simulink model "DynamicsAaa"  (R2017a)
(part 6 of 8)

% tau4 = -0.00358942*c4*(c3*(qdd(1) + qdd(2)) - qd(3)*s3*(qd(1) + qd(2))) - c5*(-3.01352e-6*c6*(-c5*(-qdd(3) + qdd(4)) - qd(5)*(c5*(-c3*s4*(qd(1) + qd(2)) + c4*s3*(qd(1) + qd(2))) - s5*(-qd(3) + qd(4))) - s5*(c4*(c3*qd(3)*(qd(1) + qd(2)) + s3*(qdd(1) + qdd(2))) + qd(4)*(-c3*c4*(qd(1) + qd(2)) - s3*s4*(qd(1) + qd(2))) - s4*(c3*(qdd(1) + qdd(2)) - qd(3)*s3*(qd(1) + qd(2))))) - 3.01352e-6*qd(6)*(c6*(c5*(-c3*s4*(qd(1) + qd(2)) + c4*s3*(qd(1) + qd(2))) - s5*(-qd(3) + qd(4))) - s6*(-c5*(-qd(3) + qd(4)) - s5*(-c3*s4*(qd(1) + qd(2)) + c4*s3*(qd(1) + qd(2))))) - 3.01352e-6*s6*(c5*(c4*(c3*qd(3)*(qd(1) + qd(2)) + s3*(qdd(1) + qdd(2))) + qd(4)*(-c3*c4*(qd(1) + qd(2)) - s3*s4*(qd(1) + qd(2))) - s4*(c3*(qdd(1) + qdd(2)) - qd(3)*s3*(qd(1) + qd(2)))) + qd(5)*(-c5*(-qd(3) + qd(4)) - s5*(-c3*s4*(qd(1) + qd(2)) + c4*s3*(qd(1) + qd(2)))) - s5*(-qdd(3) + qdd(4))) + (6.20477e-6*c6*(c5*(-c3*s4*(qd(1) + qd(2)) + c4*s3*(qd(1) + qd(2))) - s5*(-qd(3) + qd(4))) - 6.20477e-6*s6*(-c5*(-qd(3) + qd(4)) - s5*(-c3*s4*(qd(1) + qd(2)) + c4*s3*(qd(1) + qd(2)))))*(c3*c4*(qd(1) + qd(2)) - qd(5) + qd(6) + s3*s4*(qd(1) + qd(2))) - (c6*(c5*(-c3*s4*(qd(1) + qd(2)) + c4*s3*(qd(1) + qd(2))) - s5*(-qd(3) + qd(4))) - s6*(-c5*(-qd(3) + qd(4)) - s5*(-c3*s4*(qd(1) + qd(2)) + c4*s3*(qd(1) + qd(2)))))*(3.29301e-6*c3*c4*(qd(1) + qd(2)) - 3.29301e-6*qd(5) + 3.29301e-6*qd(6) + 3.29301e-6*s3*s4*(qd(1) + qd(2)))) - 0.00358942*qd(4)*(-c3*s4*(qd(1) + qd(2)) + c4*s3*(qd(1) + qd(2))) + 0.00358942*qdd(5) - 0.00358942*s4*(c3*qd(3)*(qd(1) + qd(2)) + s3*(qdd(1) + qdd(2))) - s5*(6.20477e-6*c6*(c5*(c4*(c3*qd(3)*(qd(1) + qd(2)) + s3*(qdd(1) + qdd(2))) + qd(4)*(-c3*c4*(qd(1) + qd(2)) - s3*s4*(qd(1) + qd(2))) - s4*(c3*(qdd(1) + qdd(2)) - qd(3)*s3*(qd(1) + qd(2)))) + qd(5)*(-c5*(-qd(3) + qd(4)) - s5*(-c3*s4*(qd(1) + qd(2)) + c4*s3*(qd(1) + qd(2)))) - s5*(-qdd(3) + qdd(4))) + 6.20477e-6*qd(6)*(-c6*(-c5*(-qd(3) + qd(4)) - s5*(-c3*s4*(qd(1) + qd(2)) + c4*s3*(qd(1) + qd(2)))) - s6*(c5*(-c3*s4*(qd(1) + qd(2)) + c4*s3*(qd(1) + qd(2))) - s5*(-qd(3) + qd(4)))) - 6.20477e-6*s6*(-c5*(-qdd(3) + qdd(4)) - qd(5)*(c5*(-c3*s4*(qd(1) + qd(2)) + c4*s3*(qd(1) + qd(2))) - s5*(-qd(3) + qd(4))) - s5*(c4*(c3*qd(3)*(qd(1) + qd(2)) + s3*(qdd(1) + qdd(2))) + qd(4)*(-c3*c4*(qd(1) + qd(2)) - s3*s4*(qd(1) + qd(2))) - s4*(c3*(qdd(1) + qdd(2)) - qd(3)*s3*(qd(1) + qd(2))))) + (-c6*(-c5*(-qd(3) + qd(4)) - s5*(-c3*s4*(qd(1) + qd(2)) + c4*s3*(qd(1) + qd(2)))) - s6*(c5*(-c3*s4*(qd(1) + qd(2)) + c4*s3*(qd(1) + qd(2))) - s5*(-qd(3) + qd(4))))*(3.29301e-6*c3*c4*(qd(1) + qd(2)) - 3.29301e-6*qd(5) + 3.29301e-6*qd(6) + 3.29301e-6*s3*s4*(qd(1) + qd(2))) - (-3.01352e-6*c6*(-c5*(-qd(3) + qd(4)) - s5*(-c3*s4*(qd(1) + qd(2)) + c4*s3*(qd(1) + qd(2)))) - 3.01352e-6*s6*(c5*(-c3*s4*(qd(1) + qd(2)) + c4*s3*(qd(1) + qd(2))) - s5*(-qd(3) + qd(4))))*(c3*c4*(qd(1) + qd(2)) - qd(5) + qd(6) + s3*s4*(qd(1) + qd(2)))) - (-c5*(-qd(3) + qd(4)) - s5*(-c3*s4*(qd(1) + qd(2)) + c4*s3*(qd(1) + qd(2))))*(0.000409305*c5*(-qd(3) + qd(4)) + 0.00151607*c5*(-c3*s4*(qd(1) + qd(2)) + c4*s3*(qd(1) + qd(2))) - 0.00151607*s5*(-qd(3) + qd(4)) + 0.000409305*s5*(-c3*s4*(qd(1) + qd(2)) + c4*s3*(qd(1) + qd(2)))) + (c5*(-c3*s4*(qd(1) + qd(2)) + c4*s3*(qd(1) + qd(2))) - s5*(-qd(3) + qd(4)))*(-0.00355535*c5*(-qd(3) + qd(4)) - 0.000409305*c5*(-c3*s4*(qd(1) + qd(2)) + c4*s3*(qd(1) + qd(2))) + 0.000409305*s5*(-qd(3) + qd(4)) - 0.00355535*s5*(-c3*s4*(qd(1) + qd(2)) + c4*s3*(qd(1) + qd(2))));
%  
% tau5 = 3.29301e-6*c4*(c3*(qdd(1) + qdd(2)) - qd(3)*s3*(qd(1) + qd(2))) + 3.29301e-6*qd(4)*(-c3*s4*(qd(1) + qd(2)) + c4*s3*(qd(1) + qd(2))) - 3.29301e-6*qdd(5) + 3.29301e-6*qdd(6) + 3.29301e-6*s4*(c3*qd(3)*(qd(1) + qd(2)) + s3*(qdd(1) + qdd(2))) - (-c6*(-c5*(-qd(3) + qd(4)) - s5*(-c3*s4*(qd(1) + qd(2)) + c4*s3*(qd(1) + qd(2)))) - s6*(c5*(-c3*s4*(qd(1) + qd(2)) + c4*s3*(qd(1) + qd(2))) - s5*(-qd(3) + qd(4))))*(6.20477e-6*c6*(c5*(-c3*s4*(qd(1) + qd(2)) + c4*s3*(qd(1) + qd(2))) - s5*(-qd(3) + qd(4))) - 6.20477e-6*s6*(-c5*(-qd(3) + qd(4)) - s5*(-c3*s4*(qd(1) + qd(2)) + c4*s3*(qd(1) + qd(2))))) + (-3.01352e-6*c6*(-c5*(-qd(3) + qd(4)) - s5*(-c3*s4*(qd(1) + qd(2)) + c4*s3*(qd(1) + qd(2)))) - 3.01352e-6*s6*(c5*(-c3*s4*(qd(1) + qd(2)) + c4*s3*(qd(1) + qd(2))) - s5*(-qd(3) + qd(4))))*(c6*(c5*(-c3*s4*(qd(1) + qd(2)) + c4*s3*(qd(1) + qd(2))) - s5*(-qd(3) + qd(4))) - s6*(-c5*(-qd(3) + qd(4)) - s5*(-c3*s4*(qd(1) + qd(2)) + c4*s3*(qd(1) + qd(2)))));
%  
% tau6 = 0;


%% matrix M
% m11 = diff(tau1,qdd(1))*qdd(1) ;
% m12 = diff(tau1,qdd(2))*qdd(2) ;
% m13 = diff(tau1,qdd(3))*qdd(3) ;
% m14 = diff(tau1,qdd(4))*qdd(4) ;
% m15 = diff(tau1,qdd(5))*qdd(5) ;
% m16 = diff(tau1,qdd(6))*qdd(6) ;
% 
% m21 = diff(tau2,qdd(1))*qdd(1) ;
% m22 = diff(tau2,qdd(2))*qdd(2) ;
% m23 = diff(tau2,qdd(3))*qdd(3) ;
% m24 = diff(tau2,qdd(4))*qdd(4) ;
% m25 = diff(tau2,qdd(5))*qdd(5) ;
% m26 = diff(tau2,qdd(6))*qdd(6) ;
% 
% m31 = diff(tau3,qdd(1))*qdd(1) ;
% m32 = diff(tau3,qdd(2))*qdd(2) ;
% m33 = diff(tau3,qdd(3))*qdd(3) ;
% m34 = diff(tau3,qdd(4))*qdd(4) ;
% m35 = diff(tau3,qdd(5))*qdd(5) ;
% m36 = diff(tau3,qdd(6))*qdd(6) ;
% 
% 
% m41 = diff(tau4,qdd(1))*qdd(1) ;
% m42 = diff(tau4,qdd(2))*qdd(2) ;
% m43 = diff(tau4,qdd(3))*qdd(3) ;
% m44 = diff(tau4,qdd(4))*qdd(4) ;
% m45 = diff(tau4,qdd(5))*qdd(5) ;
% m46 = diff(tau4,qdd(6))*qdd(6) ;
% 
% 
% m51 = diff(tau5,qdd(1))*qdd(1) ;
% m52 = diff(tau5,qdd(2))*qdd(2) ;
% m53 = diff(tau5,qdd(3))*qdd(3) ;
% m54 = diff(tau5,qdd(4))*qdd(4) ;
% m55 = diff(tau5,qdd(5))*qdd(5) ;
% m56 = diff(tau5,qdd(6))*qdd(6) ;
% 
% 
% m61 = diff(tau6,qdd(1))*qdd(1) ;
% m62 = diff(tau6,qdd(2))*qdd(2) ;
% m63 = diff(tau6,qdd(3))*qdd(3) ;
% m64 = diff(tau6,qdd(4))*qdd(4) ;
% m65 = diff(tau6,qdd(5))*qdd(5) ;
% m66 = diff(tau6,qdd(6))*qdd(6) ;

% m11 =  -qdd(1)*((8581632868960513*c3)/1152921504606846976 + 75*c2*(m6*(s4*(295*c3 - 270*c3*s2) - c4*(295*s3 - 270*s2*s3)) + m5*(270*c2 + 90) + m7*s5*(s6*(s5*(c4*(295*c3 - 270*c3*s2) + s4*(295*s3 - 270*s2*s3)) - 80*c5*(c3*s4 - c4*s3) + c5*(270*c2 + 90)) + c6*(c5*(c4*(295*c3 - 270*c3*s2) + s4*(295*s3 - 270*s2*s3)) + 80*s5*(c3*s4 - c4*s3) - s5*(270*c2 + 90)) + 80*c5*s6*(c3*s4 - c4*s3) - 80*c6*s5*(c3*s4 - c4*s3)) + 270*m4*s2*s3 + c5*m7*(c6*(s5*(c4*(295*c3 - 270*c3*s2) + s4*(295*s3 - 270*s2*s3)) - 80*c5*(c3*s4 - c4*s3) + c5*(270*c2 + 90)) - s6*(c5*(c4*(295*c3 - 270*c3*s2) + s4*(295*s3 - 270*s2*s3)) + 80*s5*(c3*s4 - c4*s3) - s5*(270*c2 + 90)) + 80*s5*s6*(c3*s4 - c4*s3) + 80*c5*c6*(c3*s4 - c4*s3))) - 335*c2*(c3*(c4*(m6*(c5*(c4*(295*c3 - 270*c3*s2) + s4*(295*s3 - 270*s2*s3)) - s5*(270*c2 + 90)) - m7*s5*(c6*(s5*(c4*(295*c3 - 270*c3*s2) + s4*(295*s3 - 270*s2*s3)) - 80*c5*(c3*s4 - c4*s3) + c5*(270*c2 + 90)) - s6*(c5*(c4*(295*c3 - 270*c3*s2) + s4*(295*s3 - 270*s2*s3)) + 80*s5*(c3*s4 - c4*s3) - s5*(270*c2 + 90)) + 80*s5*s6*(c3*s4 - c4*s3) + 80*c5*c6*(c3*s4 - c4*s3)) + c5*m7*(s6*(s5*(c4*(295*c3 - 270*c3*s2) + s4*(295*s3 - 270*s2*s3)) - 80*c5*(c3*s4 - c4*s3) + c5*(270*c2 + 90)) + c6*(c5*(c4*(295*c3 - 270*c3*s2) + s4*(295*s3 - 270*s2*s3)) + 80*s5*(c3*s4 - c4*s3) - s5*(270*c2 + 90)) + 80*c5*s6*(c3*s4 - c4*s3) - 80*c6*s5*(c3*s4 - c4*s3))) - s4*(m7*(s4*(295*c3 - 270*c3*s2) - c4*(295*s3 - 270*s2*s3)) - m6*(s5*(c4*(295*c3 - 270*c3*s2) + s4*(295*s3 - 270*s2*s3)) + c5*(270*c2 + 90))) + m5*(c4*(295*c3 - 270*c3*s2) - 295*c3*c4 - 295*s3*s4 + s4*(295*s3 - 270*s2*s3))) + s3*(c4*(m7*(s4*(295*c3 - 270*c3*s2) - c4*(295*s3 - 270*s2*s3)) - m6*(s5*(c4*(295*c3 - 270*c3*s2) + s4*(295*s3 - 270*s2*s3)) + c5*(270*c2 + 90))) + s4*(m6*(c5*(c4*(295*c3 - 270*c3*s2) + s4*(295*s3 - 270*s2*s3)) - s5*(270*c2 + 90)) - m7*s5*(c6*(s5*(c4*(295*c3 - 270*c3*s2) + s4*(295*s3 - 270*s2*s3)) - 80*c5*(c3*s4 - c4*s3) + c5*(270*c2 + 90)) - s6*(c5*(c4*(295*c3 - 270*c3*s2) + s4*(295*s3 - 270*s2*s3)) + 80*s5*(c3*s4 - c4*s3) - s5*(270*c2 + 90)) + 80*s5*s6*(c3*s4 - c4*s3) + 80*c5*c6*(c3*s4 - c4*s3)) + c5*m7*(s6*(s5*(c4*(295*c3 - 270*c3*s2) + s4*(295*s3 - 270*s2*s3)) - 80*c5*(c3*s4 - c4*s3) + c5*(270*c2 + 90)) + c6*(c5*(c4*(295*c3 - 270*c3*s2) + s4*(295*s3 - 270*s2*s3)) + 80*s5*(c3*s4 - c4*s3) - s5*(270*c2 + 90)) + 80*c5*s6*(c3*s4 - c4*s3) - 80*c6*s5*(c3*s4 - c4*s3))) + m5*(s4*(295*c3 - 270*c3*s2) - 295*c3*s4 + 295*c4*s3 - c4*(295*s3 - 270*s2*s3))) - 270*c3*m4*s2) - c3*(s4*(c5*((1831324867619693*s5*s6*(c3*s4 - c4*s3))/295147905179352825856 + (1831324867619693*c5*c6*(c3*s4 - c4*s3))/295147905179352825856) + s5*((7115472921728667*c5*s6*(c3*s4 - c4*s3))/2361183241434822606848 - (7115472921728667*c6*s5*(c3*s4 - c4*s3))/2361183241434822606848) + (3495819410978605*c5*(c3*s4 - c4*s3))/2305843009213693952 + 295*m7*(s4*(295*c3 - 270*c3*s2) - c4*(295*s3 - 270*s2*s3)) + (943793072886211*s5*(c3*s4 - c4*s3))/2305843009213693952 - 295*m6*(s5*(c4*(295*c3 - 270*c3*s2) + s4*(295*s3 - 270*s2*s3)) + c5*(270*c2 + 90))) - c4*((7775400025877285*c3*c4)/2361183241434822606848 + (7775400025877285*s3*s4)/2361183241434822606848 + (943793072886211*c5*(c3*s4 - c4*s3))/2305843009213693952 + (8198078942807907*s5*(c3*s4 - c4*s3))/2305843009213693952 + 295*m6*(c5*(c4*(295*c3 - 270*c3*s2) + s4*(295*s3 - 270*s2*s3)) - s5*(270*c2 + 90)) - 295*m7*s5*(c6*(s5*(c4*(295*c3 - 270*c3*s2) + s4*(295*s3 - 270*s2*s3)) - 80*c5*(c3*s4 - c4*s3) + c5*(270*c2 + 90)) - s6*(c5*(c4*(295*c3 - 270*c3*s2) + s4*(295*s3 - 270*s2*s3)) + 80*s5*(c3*s4 - c4*s3) - s5*(270*c2 + 90)) + 80*s5*s6*(c3*s4 - c4*s3) + 80*c5*c6*(c3*s4 - c4*s3)) + 295*c5*m7*(s6*(s5*(c4*(295*c3 - 270*c3*s2) + s4*(295*s3 - 270*s2*s3)) - 80*c5*(c3*s4 - c4*s3) + c5*(270*c2 + 90)) + c6*(c5*(c4*(295*c3 - 270*c3*s2) + s4*(295*s3 - 270*s2*s3)) + 80*s5*(c3*s4 - c4*s3) - s5*(270*c2 + 90)) + 80*c5*s6*(c3*s4 - c4*s3) - 80*c6*s5*(c3*s4 - c4*s3))) - (5813615622121687*c3*c4)/288230376151711744 + (1883354923850515*c3*s4)/1152921504606846976 - (1883354923850515*c4*s3)/1152921504606846976 - (5813615622121687*s3*s4)/288230376151711744 + 90*m6*(s4*(295*c3 - 270*c3*s2) - c4*(295*s3 - 270*s2*s3)) + 90*m5*(270*c2 + 90) + 90*m7*s5*(s6*(s5*(c4*(295*c3 - 270*c3*s2) + s4*(295*s3 - 270*s2*s3)) - 80*c5*(c3*s4 - c4*s3) + c5*(270*c2 + 90)) + c6*(c5*(c4*(295*c3 - 270*c3*s2) + s4*(295*s3 - 270*s2*s3)) + 80*s5*(c3*s4 - c4*s3) - s5*(270*c2 + 90)) + 80*c5*s6*(c3*s4 - c4*s3) - 80*c6*s5*(c3*s4 - c4*s3)) + 90*c5*m7*(c6*(s5*(c4*(295*c3 - 270*c3*s2) + s4*(295*s3 - 270*s2*s3)) - 80*c5*(c3*s4 - c4*s3) + c5*(270*c2 + 90)) - s6*(c5*(c4*(295*c3 - 270*c3*s2) + s4*(295*s3 - 270*s2*s3)) + 80*s5*(c3*s4 - c4*s3) - s5*(270*c2 + 90)) + 80*s5*s6*(c3*s4 - c4*s3) + 80*c5*c6*(c3*s4 - c4*s3))) + 270*c5*m7*((7145951600741313*s3)/288230376151711744 + 90450*m3*s2 + 335*s2*(m6*(s4*(295*c3 - 270*c3*s2) - c4*(295*s3 - 270*s2*s3)) + m5*(270*c2 + 90) + m7*s5*(s6*(s5*(c4*(295*c3 - 270*c3*s2) + s4*(295*s3 - 270*s2*s3)) - 80*c5*(c3*s4 - c4*s3) + c5*(270*c2 + 90)) + c6*(c5*(c4*(295*c3 - 270*c3*s2) + s4*(295*s3 - 270*s2*s3)) + 80*s5*(c3*s4 - c4*s3) - s5*(270*c2 + 90)) + 80*c5*s6*(c3*s4 - c4*s3) - 80*c6*s5*(c3*s4 - c4*s3)) + 270*m4*s2*s3 + c5*m7*(c6*(s5*(c4*(295*c3 - 270*c3*s2) + s4*(295*s3 - 270*s2*s3)) - 80*c5*(c3*s4 - c4*s3) + c5*(270*c2 + 90)) - s6*(c5*(c4*(295*c3 - 270*c3*s2) + s4*(295*s3 - 270*s2*s3)) + 80*s5*(c3*s4 - c4*s3) - s5*(270*c2 + 90)) + 80*s5*s6*(c3*s4 - c4*s3) + 80*c5*c6*(c3*s4 - c4*s3))) + s3*(c4*(c5*((1831324867619693*s5*s6*(c3*s4 - c4*s3))/295147905179352825856 + (1831324867619693*c5*c6*(c3*s4 - c4*s3))/295147905179352825856) + s5*((7115472921728667*c5*s6*(c3*s4 - c4*s3))/2361183241434822606848 - (7115472921728667*c6*s5*(c3*s4 - c4*s3))/2361183241434822606848) + (3495819410978605*c5*(c3*s4 - c4*s3))/2305843009213693952 + 295*m7*(s4*(295*c3 - 270*c3*s2) - c4*(295*s3 - 270*s2*s3)) + (943793072886211*s5*(c3*s4 - c4*s3))/2305843009213693952 - 295*m6*(s5*(c4*(295*c3 - 270*c3*s2) + s4*(295*s3 - 270*s2*s3)) + c5*(270*c2 + 90))) - (1883354923850515*c3*c4)/1152921504606846976 + s4*((7775400025877285*c3*c4)/2361183241434822606848 + (7775400025877285*s3*s4)/2361183241434822606848 + (943793072886211*c5*(c3*s4 - c4*s3))/2305843009213693952 + (8198078942807907*s5*(c3*s4 - c4*s3))/2305843009213693952 + 295*m6*(c5*(c4*(295*c3 - 270*c3*s2) + s4*(295*s3 - 270*s2*s3)) - s5*(270*c2 + 90)) - 295*m7*s5*(c6*(s5*(c4*(295*c3 - 270*c3*s2) + s4*(295*s3 - 270*s2*s3)) - 80*c5*(c3*s4 - c4*s3) + c5*(270*c2 + 90)) - s6*(c5*(c4*(295*c3 - 270*c3*s2) + s4*(295*s3 - 270*s2*s3)) + 80*s5*(c3*s4 - c4*s3) - s5*(270*c2 + 90)) + 80*s5*s6*(c3*s4 - c4*s3) + 80*c5*c6*(c3*s4 - c4*s3)) + 295*c5*m7*(s6*(s5*(c4*(295*c3 - 270*c3*s2) + s4*(295*s3 - 270*s2*s3)) - 80*c5*(c3*s4 - c4*s3) + c5*(270*c2 + 90)) + c6*(c5*(c4*(295*c3 - 270*c3*s2) + s4*(295*s3 - 270*s2*s3)) + 80*s5*(c3*s4 - c4*s3) - s5*(270*c2 + 90)) + 80*c5*s6*(c3*s4 - c4*s3) - 80*c6*s5*(c3*s4 - c4*s3))) + (1369254254579395*c3*s4)/144115188075855872 - (1369254254579395*c4*s3)/144115188075855872 - (1883354923850515*s3*s4)/1152921504606846976) + 270*m6*(s4*(295*c3 - 270*c3*s2) - c4*(295*s3 - 270*s2*s3)) + 75*s2*(c3*(c4*(m6*(c5*(c4*(295*c3 - 270*c3*s2) + s4*(295*s3 - 270*s2*s3)) - s5*(270*c2 + 90)) - m7*s5*(c6*(s5*(c4*(295*c3 - 270*c3*s2) + s4*(295*s3 - 270*s2*s3)) - 80*c5*(c3*s4 - c4*s3) + c5*(270*c2 + 90)) - s6*(c5*(c4*(295*c3 - 270*c3*s2) + s4*(295*s3 - 270*s2*s3)) + 80*s5*(c3*s4 - c4*s3) - s5*(270*c2 + 90)) + 80*s5*s6*(c3*s4 - c4*s3) + 80*c5*c6*(c3*s4 - c4*s3)) + c5*m7*(s6*(s5*(c4*(295*c3 - 270*c3*s2) + s4*(295*s3 - 270*s2*s3)) - 80*c5*(c3*s4 - c4*s3) + c5*(270*c2 + 90)) + c6*(c5*(c4*(295*c3 - 270*c3*s2) + s4*(295*s3 - 270*s2*s3)) + 80*s5*(c3*s4 - c4*s3) - s5*(270*c2 + 90)) + 80*c5*s6*(c3*s4 - c4*s3) - 80*c6*s5*(c3*s4 - c4*s3))) - s4*(m7*(s4*(295*c3 - 270*c3*s2) - c4*(295*s3 - 270*s2*s3)) - m6*(s5*(c4*(295*c3 - 270*c3*s2) + s4*(295*s3 - 270*s2*s3)) + c5*(270*c2 + 90))) + m5*(c4*(295*c3 - 270*c3*s2) - 295*c3*c4 - 295*s3*s4 + s4*(295*s3 - 270*s2*s3))) + s3*(c4*(m7*(s4*(295*c3 - 270*c3*s2) - c4*(295*s3 - 270*s2*s3)) - m6*(s5*(c4*(295*c3 - 270*c3*s2) + s4*(295*s3 - 270*s2*s3)) + c5*(270*c2 + 90))) + s4*(m6*(c5*(c4*(295*c3 - 270*c3*s2) + s4*(295*s3 - 270*s2*s3)) - s5*(270*c2 + 90)) - m7*s5*(c6*(s5*(c4*(295*c3 - 270*c3*s2) + s4*(295*s3 - 270*s2*s3)) - 80*c5*(c3*s4 - c4*s3) + c5*(270*c2 + 90)) - s6*(c5*(c4*(295*c3 - 270*c3*s2) + s4*(295*s3 - 270*s2*s3)) + 80*s5*(c3*s4 - c4*s3) - s5*(270*c2 + 90)) + 80*s5*s6*(c3*s4 - c4*s3) + 80*c5*c6*(c3*s4 - c4*s3)) + c5*m7*(s6*(s5*(c4*(295*c3 - 270*c3*s2) + s4*(295*s3 - 270*s2*s3)) - 80*c5*(c3*s4 - c4*s3) + c5*(270*c2 + 90)) + c6*(c5*(c4*(295*c3 - 270*c3*s2) + s4*(295*s3 - 270*s2*s3)) + 80*s5*(c3*s4 - c4*s3) - s5*(270*c2 + 90)) + 80*c5*s6*(c3*s4 - c4*s3) - 80*c6*s5*(c3*s4 - c4*s3))) + m5*(s4*(295*c3 - 270*c3*s2) - 295*c3*s4 + 295*c4*s3 - c4*(295*s3 - 270*s2*s3))) - 270*c3*m4*s2) - c6*(80*c5*(c3*s4 - c4*s3) - s6*(c5*(c4*(295*c3 - 270*c3*s2) + s4*(295*s3 - 270*s2*s3)) + 80*s5*(c3*s4 - c4*s3) - s5*(270*c2 + 90)) + c5*(s5*(c4*(295*c3 - 270*c3*s2) + s4*(295*s3 - 270*s2*s3)) - 270*c2 + 26550*c3^2) + 80*s5*s6*(c3*s4 - c4*s3)) + 270*m5*(270*c2 + 90) - 75*m3*(270*c2 + 270) + 270*m7*s5*(s6*(s5*(c4*(295*c3 - 270*c3*s2) + s4*(295*s3 - 270*s2*s3)) - 80*c5*(c3*s4 - c4*s3) + c5*(270*c2 + 90)) + c6*(c5*(c4*(295*c3 - 270*c3*s2) + s4*(295*s3 - 270*s2*s3)) + 80*s5*(c3*s4 - c4*s3) - s5*(270*c2 + 90)) + 80*c5*s6*(c3*s4 - c4*s3) - 80*c6*s5*(c3*s4 - c4*s3)) + 72900*m4*s2*s3 + 80*c5*c6*(c3*s4 - c4*s3) - 6288408585614741/144115188075855872))
% 
% m12 = -qdd(2)*((8581632868960513*c3)/1152921504606846976 + 75*c2*(90*m5 + m6*(295*c3*s4 - 295*c4*s3) + c5*m7*(c6*(90*c5 - 80*c5*(c3*s4 - c4*s3) + s5*(295*c3*c4 + 295*s3*s4)) - s6*(c5*(295*c3*c4 + 295*s3*s4) - 90*s5 + 80*s5*(c3*s4 - c4*s3)) + 80*s5*s6*(c3*s4 - c4*s3) + 80*c5*c6*(c3*s4 - c4*s3)) + m7*s5*(c6*(c5*(295*c3*c4 + 295*s3*s4) - 90*s5 + 80*s5*(c3*s4 - c4*s3)) + s6*(90*c5 - 80*c5*(c3*s4 - c4*s3) + s5*(295*c3*c4 + 295*s3*s4)) + 80*c5*s6*(c3*s4 - c4*s3) - 80*c6*s5*(c3*s4 - c4*s3))) + 335*c2*(c3*(c4*(m6*(90*s5 - c5*(295*c3*c4 + 295*s3*s4)) - c5*m7*(c6*(c5*(295*c3*c4 + 295*s3*s4) - 90*s5 + 80*s5*(c3*s4 - c4*s3)) + s6*(90*c5 - 80*c5*(c3*s4 - c4*s3) + s5*(295*c3*c4 + 295*s3*s4)) + 80*c5*s6*(c3*s4 - c4*s3) - 80*c6*s5*(c3*s4 - c4*s3)) + m7*s5*(c6*(90*c5 - 80*c5*(c3*s4 - c4*s3) + s5*(295*c3*c4 + 295*s3*s4)) - s6*(c5*(295*c3*c4 + 295*s3*s4) - 90*s5 + 80*s5*(c3*s4 - c4*s3)) + 80*s5*s6*(c3*s4 - c4*s3) + 80*c5*c6*(c3*s4 - c4*s3))) - s4*(m6*(90*c5 + s5*(295*c3*c4 + 295*s3*s4)) - m7*(295*c3*s4 - 295*c4*s3))) + s3*(c4*(m6*(90*c5 + s5*(295*c3*c4 + 295*s3*s4)) - m7*(295*c3*s4 - 295*c4*s3)) + s4*(m6*(90*s5 - c5*(295*c3*c4 + 295*s3*s4)) - c5*m7*(c6*(c5*(295*c3*c4 + 295*s3*s4) - 90*s5 + 80*s5*(c3*s4 - c4*s3)) + s6*(90*c5 - 80*c5*(c3*s4 - c4*s3) + s5*(295*c3*c4 + 295*s3*s4)) + 80*c5*s6*(c3*s4 - c4*s3) - 80*c6*s5*(c3*s4 - c4*s3)) + m7*s5*(c6*(90*c5 - 80*c5*(c3*s4 - c4*s3) + s5*(295*c3*c4 + 295*s3*s4)) - s6*(c5*(295*c3*c4 + 295*s3*s4) - 90*s5 + 80*s5*(c3*s4 - c4*s3)) + 80*s5*s6*(c3*s4 - c4*s3) + 80*c5*c6*(c3*s4 - c4*s3))))) - c3*(8100*m5 + s4*(c5*((1831324867619693*s5*s6*(c3*s4 - c4*s3))/295147905179352825856 + (1831324867619693*c5*c6*(c3*s4 - c4*s3))/295147905179352825856) + s5*((7115472921728667*c5*s6*(c3*s4 - c4*s3))/2361183241434822606848 - (7115472921728667*c6*s5*(c3*s4 - c4*s3))/2361183241434822606848) - 295*m6*(90*c5 + s5*(295*c3*c4 + 295*s3*s4)) + (3495819410978605*c5*(c3*s4 - c4*s3))/2305843009213693952 + 295*m7*(295*c3*s4 - 295*c4*s3) + (943793072886211*s5*(c3*s4 - c4*s3))/2305843009213693952) - (5813615622121687*c3*c4)/288230376151711744 + (1883354923850515*c3*s4)/1152921504606846976 - (1883354923850515*c4*s3)/1152921504606846976 - (5813615622121687*s3*s4)/288230376151711744 + 90*m6*(295*c3*s4 - 295*c4*s3) - c4*((7775400025877285*c3*c4)/2361183241434822606848 + (7775400025877285*s3*s4)/2361183241434822606848 - 295*m6*(90*s5 - c5*(295*c3*c4 + 295*s3*s4)) + (943793072886211*c5*(c3*s4 - c4*s3))/2305843009213693952 + (8198078942807907*s5*(c3*s4 - c4*s3))/2305843009213693952 + 295*c5*m7*(c6*(c5*(295*c3*c4 + 295*s3*s4) - 90*s5 + 80*s5*(c3*s4 - c4*s3)) + s6*(90*c5 - 80*c5*(c3*s4 - c4*s3) + s5*(295*c3*c4 + 295*s3*s4)) + 80*c5*s6*(c3*s4 - c4*s3) - 80*c6*s5*(c3*s4 - c4*s3)) - 295*m7*s5*(c6*(90*c5 - 80*c5*(c3*s4 - c4*s3) + s5*(295*c3*c4 + 295*s3*s4)) - s6*(c5*(295*c3*c4 + 295*s3*s4) - 90*s5 + 80*s5*(c3*s4 - c4*s3)) + 80*s5*s6*(c3*s4 - c4*s3) + 80*c5*c6*(c3*s4 - c4*s3))) + 90*c5*m7*(c6*(90*c5 - 80*c5*(c3*s4 - c4*s3) + s5*(295*c3*c4 + 295*s3*s4)) - s6*(c5*(295*c3*c4 + 295*s3*s4) - 90*s5 + 80*s5*(c3*s4 - c4*s3)) + 80*s5*s6*(c3*s4 - c4*s3) + 80*c5*c6*(c3*s4 - c4*s3)) + 90*m7*s5*(c6*(c5*(295*c3*c4 + 295*s3*s4) - 90*s5 + 80*s5*(c3*s4 - c4*s3)) + s6*(90*c5 - 80*c5*(c3*s4 - c4*s3) + s5*(295*c3*c4 + 295*s3*s4)) + 80*c5*s6*(c3*s4 - c4*s3) - 80*c6*s5*(c3*s4 - c4*s3))) + 270*c5*m7*(24300*m5 - 20250*m3 + (7145951600741313*s3)/288230376151711744 + 335*s2*(90*m5 + m6*(295*c3*s4 - 295*c4*s3) + c5*m7*(c6*(90*c5 - 80*c5*(c3*s4 - c4*s3) + s5*(295*c3*c4 + 295*s3*s4)) - s6*(c5*(295*c3*c4 + 295*s3*s4) - 90*s5 + 80*s5*(c3*s4 - c4*s3)) + 80*s5*s6*(c3*s4 - c4*s3) + 80*c5*c6*(c3*s4 - c4*s3)) + m7*s5*(c6*(c5*(295*c3*c4 + 295*s3*s4) - 90*s5 + 80*s5*(c3*s4 - c4*s3)) + s6*(90*c5 - 80*c5*(c3*s4 - c4*s3) + s5*(295*c3*c4 + 295*s3*s4)) + 80*c5*s6*(c3*s4 - c4*s3) - 80*c6*s5*(c3*s4 - c4*s3))) + 270*m6*(295*c3*s4 - 295*c4*s3) - c6*(80*c5*(c3*s4 - c4*s3) - s6*(c5*(295*c3*c4 + 295*s3*s4) - 90*s5 + 80*s5*(c3*s4 - c4*s3)) + c5*(s5*(295*c3*c4 + 295*s3*s4) + 26550*c3^2) + 80*s5*s6*(c3*s4 - c4*s3)) - 75*s2*(c3*(c4*(m6*(90*s5 - c5*(295*c3*c4 + 295*s3*s4)) - c5*m7*(c6*(c5*(295*c3*c4 + 295*s3*s4) - 90*s5 + 80*s5*(c3*s4 - c4*s3)) + s6*(90*c5 - 80*c5*(c3*s4 - c4*s3) + s5*(295*c3*c4 + 295*s3*s4)) + 80*c5*s6*(c3*s4 - c4*s3) - 80*c6*s5*(c3*s4 - c4*s3)) + m7*s5*(c6*(90*c5 - 80*c5*(c3*s4 - c4*s3) + s5*(295*c3*c4 + 295*s3*s4)) - s6*(c5*(295*c3*c4 + 295*s3*s4) - 90*s5 + 80*s5*(c3*s4 - c4*s3)) + 80*s5*s6*(c3*s4 - c4*s3) + 80*c5*c6*(c3*s4 - c4*s3))) - s4*(m6*(90*c5 + s5*(295*c3*c4 + 295*s3*s4)) - m7*(295*c3*s4 - 295*c4*s3))) + s3*(c4*(m6*(90*c5 + s5*(295*c3*c4 + 295*s3*s4)) - m7*(295*c3*s4 - 295*c4*s3)) + s4*(m6*(90*s5 - c5*(295*c3*c4 + 295*s3*s4)) - c5*m7*(c6*(c5*(295*c3*c4 + 295*s3*s4) - 90*s5 + 80*s5*(c3*s4 - c4*s3)) + s6*(90*c5 - 80*c5*(c3*s4 - c4*s3) + s5*(295*c3*c4 + 295*s3*s4)) + 80*c5*s6*(c3*s4 - c4*s3) - 80*c6*s5*(c3*s4 - c4*s3)) + m7*s5*(c6*(90*c5 - 80*c5*(c3*s4 - c4*s3) + s5*(295*c3*c4 + 295*s3*s4)) - s6*(c5*(295*c3*c4 + 295*s3*s4) - 90*s5 + 80*s5*(c3*s4 - c4*s3)) + 80*s5*s6*(c3*s4 - c4*s3) + 80*c5*c6*(c3*s4 - c4*s3))))) - s3*((1883354923850515*c3*c4)/1152921504606846976 - (1369254254579395*c3*s4)/144115188075855872 + (1369254254579395*c4*s3)/144115188075855872 + (1883354923850515*s3*s4)/1152921504606846976 - s4*((7775400025877285*c3*c4)/2361183241434822606848 + (7775400025877285*s3*s4)/2361183241434822606848 - 295*m6*(90*s5 - c5*(295*c3*c4 + 295*s3*s4)) + (943793072886211*c5*(c3*s4 - c4*s3))/2305843009213693952 + (8198078942807907*s5*(c3*s4 - c4*s3))/2305843009213693952 + 295*c5*m7*(c6*(c5*(295*c3*c4 + 295*s3*s4) - 90*s5 + 80*s5*(c3*s4 - c4*s3)) + s6*(90*c5 - 80*c5*(c3*s4 - c4*s3) + s5*(295*c3*c4 + 295*s3*s4)) + 80*c5*s6*(c3*s4 - c4*s3) - 80*c6*s5*(c3*s4 - c4*s3)) - 295*m7*s5*(c6*(90*c5 - 80*c5*(c3*s4 - c4*s3) + s5*(295*c3*c4 + 295*s3*s4)) - s6*(c5*(295*c3*c4 + 295*s3*s4) - 90*s5 + 80*s5*(c3*s4 - c4*s3)) + 80*s5*s6*(c3*s4 - c4*s3) + 80*c5*c6*(c3*s4 - c4*s3))) - c4*(c5*((1831324867619693*s5*s6*(c3*s4 - c4*s3))/295147905179352825856 + (1831324867619693*c5*c6*(c3*s4 - c4*s3))/295147905179352825856) + s5*((7115472921728667*c5*s6*(c3*s4 - c4*s3))/2361183241434822606848 - (7115472921728667*c6*s5*(c3*s4 - c4*s3))/2361183241434822606848) - 295*m6*(90*c5 + s5*(295*c3*c4 + 295*s3*s4)) + (3495819410978605*c5*(c3*s4 - c4*s3))/2305843009213693952 + 295*m7*(295*c3*s4 - 295*c4*s3) + (943793072886211*s5*(c3*s4 - c4*s3))/2305843009213693952)) + 270*m7*s5*(c6*(c5*(295*c3*c4 + 295*s3*s4) - 90*s5 + 80*s5*(c3*s4 - c4*s3)) + s6*(90*c5 - 80*c5*(c3*s4 - c4*s3) + s5*(295*c3*c4 + 295*s3*s4)) + 80*c5*s6*(c3*s4 - c4*s3) - 80*c6*s5*(c3*s4 - c4*s3)) + 80*c5*c6*(c3*s4 - c4*s3) - 6288408585614741/144115188075855872));
%  
% m13 = qdd(3)*(6750*c2*m4 + c3*(s4*((943793072886211*c5)/2305843009213693952 - (3495819410978605*s5)/2305843009213693952 + c5*((1831324867619693*c5*s6)/295147905179352825856 - (1831324867619693*c6*s5)/295147905179352825856) - s5*((7115472921728667*c5*c6)/2361183241434822606848 + (7115472921728667*s5*s6)/2361183241434822606848)) - c4*((8198078942807907*c5)/2305843009213693952 - (943793072886211*s5)/2305843009213693952) + 397124457897871/147573952589676412928) + 270*c5*m7*(24300*m4 + 80*c6*s5 + 30150*m4*s2 - s3*(c4*((943793072886211*c5)/2305843009213693952 - (3495819410978605*s5)/2305843009213693952 + c5*((1831324867619693*c5*s6)/295147905179352825856 - (1831324867619693*c6*s5)/295147905179352825856) - s5*((7115472921728667*c5*c6)/2361183241434822606848 + (7115472921728667*s5*s6)/2361183241434822606848)) + s4*((8198078942807907*c5)/2305843009213693952 - (943793072886211*s5)/2305843009213693952) - 4965898922391233/590295810358705651712) + 80*c5*c6*s5 + 7478065051662123/36028797018963968));
% 
% m14 = -qdd(4)*(c3*(s4*((943793072886211*c5)/2305843009213693952 - (3495819410978605*s5)/2305843009213693952 + c5*((1831324867619693*c5*s6)/295147905179352825856 - (1831324867619693*c6*s5)/295147905179352825856) - s5*((7115472921728667*c5*c6)/2361183241434822606848 + (7115472921728667*s5*s6)/2361183241434822606848)) - c4*((8198078942807907*c5)/2305843009213693952 - (943793072886211*s5)/2305843009213693952) + 397124457897871/147573952589676412928) + 270*c5*m7*(80*c6*s5 - s3*(c4*((943793072886211*c5)/2305843009213693952 - (3495819410978605*s5)/2305843009213693952 + c5*((1831324867619693*c5*s6)/295147905179352825856 - (1831324867619693*c6*s5)/295147905179352825856) - s5*((7115472921728667*c5*c6)/2361183241434822606848 + (7115472921728667*s5*s6)/2361183241434822606848)) + s4*((8198078942807907*c5)/2305843009213693952 - (943793072886211*s5)/2305843009213693952) - 4965898922391233/590295810358705651712) + 80*c5*c6*s5));
%  
% m15 = qdd(5)*((7775400025877285*c3*c4)/2361183241434822606848 + (1049679003493433475*c5*m7*s3*s4)/1180591620717411303424);
%  
% m16 = -qdd(6)*((7775400025877285*c3*c4)/2361183241434822606848 + (1049679003493433475*c5*m7*s3*s4)/1180591620717411303424);
%  
% 
% m21= -qdd1*((8581632868960513*c3)/1152921504606846976 + c3*((7145951600741313*s3)/288230376151711744 + (5813615622121687*c3*c4)/288230376151711744 + (1883354923850515*c4*s3)/1152921504606846976 + 270*m6*(s4*(295*c3 - 270*c3*s2) - c4*(295*s3 - 270*s2*s3)) + s3*(c4*(c5*((1831324867619693*s5*s6*(c3*s4 - c4*s3))/295147905179352825856 + (1831324867619693*c5*c6*(c3*s4 - c4*s3))/295147905179352825856) + s5*((7115472921728667*c5*s6*(c3*s4 - c4*s3))/2361183241434822606848 - (7115472921728667*c6*s5*(c3*s4 - c4*s3))/2361183241434822606848) + (3495819410978605*c5*(c3*s4 - c4*s3))/2305843009213693952 + 295*m7*(s4*(295*c3 - 270*c3*s2) - c4*(295*s3 - 270*s2*s3)) + (943793072886211*s5*(c3*s4 - c4*s3))/2305843009213693952 - 295*m6*(s5*(c4*(295*c3 - 270*c3*s2) + s4*(295*s3 - 270*s2*s3)) + c5*(270*c2 + 90))) - (1883354923850515*c3*c4)/1152921504606846976 + (1369254254579395*c3*s4)/144115188075855872 - (1369254254579395*c4*s3)/144115188075855872 - (1883354923850515*s3*s4)/1152921504606846976 + s4*((7775400025877285*c3*c4)/2361183241434822606848 - 295*c5*m7*((7775400025877285*s3*s4)/2361183241434822606848 - c6*(c5*(c4*(295*c3 - 270*c3*s2) + s4*(295*s3 - 270*s2*s3)) + 80*s5*(c3*s4 - c4*s3) - s5*(270*c2 + 90)) + (943793072886211*c5*(c3*s4 - c4*s3))/2305843009213693952 - s6*(c5*(270*c2 + 90) - 80*c5*(c3*s4 - c4*s3) + s5*(c4*(295*c3 - 270*c3*s2) + s4*(295*s3 - 270*c2*s2*s3))) + (8198078942807907*s5*(c3*s4 - c4*s3))/2305843009213693952 + 295*m6*(c5*(c4*(295*c3 - 270*c3*s2) + s4*(295*s3 - 270*s2*s3)) - s5*(270*c2 + 90)) - 295*m7*s5*(c6*(s5*(c4*(295*c3 - 270*c3*s2) + s4*(295*s3 - 270*s2*s3)) - 80*c5*(c3*s4 - c4*s3) + c5*(270*c2 + 90)) - s6*(c5*(c4*(295*c3 - 270*c3*s2) + s4*(295*s3 - 270*s2*s3)) + 80*s5*(c3*s4 - c4*s3) - s5*(270*c2 + 90)) + 80*s5*s6*(c3*s4 - c4*s3) + 80*c5*c6*(c3*s4 - c4*s3)) - 80*c5*s6*(c3*s4 - c4*s3) + 80*c6*s5*(c3*s4 - c4*s3)))) + c4*(s4*(c5*((1831324867619693*s5*s6*(c3*s4 - c4*s3))/295147905179352825856 + (1831324867619693*c5*c6*(c3*s4 - c4*s3))/295147905179352825856) + s5*((7115472921728667*c5*s6*(c3*s4 - c4*s3))/2361183241434822606848 - (7115472921728667*c6*s5*(c3*s4 - c4*s3))/2361183241434822606848) + (3495819410978605*c5*(c3*s4 - c4*s3))/2305843009213693952 + 295*m7*(s4*(295*c3 - 270*c3*s2) - c4*(295*s3 - 270*s2*s3)) + (943793072886211*s5*(c3*s4 - c4*s3))/2305843009213693952 - 295*m6*(s5*(c4*(295*c3 - 270*c3*s2) + s4*(295*s3 - 270*s2*s3)) + c5*(270*c2 + 90))) + (7775400025877285*c3*c4)/2361183241434822606848 + (1883354923850515*c3*s4)/1152921504606846976 - (5813615622121687*s3*s4)/288230376151711744 + (943793072886211*c5*(c3*s4 - c4*s3))/2305843009213693952 + 90*m6*(s4*(295*c3 - 270*c3*s2) - c4*(295*s3 - 270*s2*s3)) + 90*m5*(270*c2 + 90) - 295*m6*((7775400025877285*s3*s4)/2361183241434822606848 - c5*(c4*(295*c3 - 270*c3*s2) + s4*(295*s3 - 270*s2*s3)) + (8198078942807907*s5*(c3*s4 - c4*s3))/2305843009213693952 + s5*(270*c2 + 90) - 295*m7*s5*(c6*(s5*(c4*(295*c3 - 270*c3*s2) + s4*(295*s3 - 270*s2*s3)) - 80*c5*(c3*s4 - c4*s3) + c5*(270*c2 + 90)) - s6*(c5*(c4*(295*c3 - 270*c3*s2) + s4*(295*s3 - 270*s2*s3)) + 80*s5*(c3*s4 - c4*s3) - s5*(270*c2 + 90)) + 80*s5*s6*(c3*s4 - c4*s3) + 80*c5*c6*(c3*s4 - c4*s3))) + 90*m7*s5*(s6*(s5*(c4*(295*c3 - 270*c3*s2) + s4*(295*s3 - 270*s2*s3)) - 80*c5*(c3*s4 - c4*s3) + c5*(270*c2 + 90)) + c6*(c5*(c4*(295*c3 - 270*c3*s2) + s4*(295*s3 - 270*s2*s3)) + 80*s5*(c3*s4 - c4*s3) - s5*(270*c2 + 90)) + 80*c5*s6*(c3*s4 - c4*s3) - 80*c6*s5*(c3*s4 - c4*s3)) + 295*c5*m7*(s6*(s5*(c4*(295*c3 - 270*c3*s2) + s4*(295*s3 - 270*s2*s3)) - 80*c5*(c3*s4 - c4*s3) + c5*(270*c2 + 90)) + c6*(c5*(c4*(295*c3 - 270*c3*s2) + s4*(295*s3 - 270*s2*s3)) + 80*s5*(c3*s4 - c4*s3) - s5*(270*c2 + 90)) + 80*c5*s6*(c3*s4 - c4*s3) - 80*c6*s5*(c3*s4 - c4*s3)) + 90*c5*m7*(c6*(s5*(c4*(295*c3 - 270*c3*s2) + s4*(295*s3 - 270*s2*s3)) - 80*c5*(c3*s4 - c4*s3) + c5*(270*c2 + 90)) - s6*(c5*(c4*(295*c3 - 270*c3*s2) + s4*(295*s3 - 270*s2*s3)) + 80*s5*(c3*s4 - c4*s3) - s5*(270*c2 + 90)) + 80*s5*s6*(c3*s4 - c4*s3) + 80*c5*c6*(c3*s4 - c4*s3))) + 270*m5*(270*c2 + 90) + 270*m7*s5*(s6*(s5*(c4*(295*c3 - 270*c3*s2) + s4*(295*s3 - 270*s2*s3)) - 80*c5*(c3*s4 - c4*s3) + c5*(270*c2 + 90)) + c6*(c5*(c4*(295*c3 - 270*c3*s2) + s4*(295*s3 - 270*s2*s3)) + 80*s5*(c3*s4 - c4*s3) - s5*(270*c2 + 90)) + 80*c5*s6*(c3*s4 - c4*s3) - 80*c6*s5*(c3*s4 - c4*s3)) + 72900*m4*s2*s3 + 270*c5*m7*(c6*(s5*(c4*(295*c3 - 270*c3*s2) + s4*(295*s3 - 270*s2*s3)) - 80*c5*(c3*s4 - c4*s3) + c5*(270*c2 + 90)) - s6*(c5*(c4*(295*c3 - 270*c3*s2) + s4*(295*s3 - 270*s2*s3)) + 80*s5*(c3*s4 - c4*s3) - s5*(270*c2 + 90)) + 80*s5*s6*(c3*s4 - c4*s3) + 80*c5*c6*(c3*s4 - c4*s3))));
%  
% m22 = -qdd(2)*((8581632868960513*c3)/1152921504606846976 + c3*(24300*m5 + (7145951600741313*s3)/288230376151711744 + (5813615622121687*c3*c4)/288230376151711744 + (1883354923850515*c4*s3)/1152921504606846976 + 270*m6*(295*c3*s4 - 295*c4*s3) + c4*(8100*m5 + s4*(c5*((1831324867619693*s5*s6*(c3*s4 - c4*s3))/295147905179352825856 + (1831324867619693*c5*c6*(c3*s4 - c4*s3))/295147905179352825856) + s5*((7115472921728667*c5*s6*(c3*s4 - c4*s3))/2361183241434822606848 - (7115472921728667*c6*s5*(c3*s4 - c4*s3))/2361183241434822606848) - 295*m6*(90*c5 + s5*(295*c3*c4 + 295*s3*s4)) + (3495819410978605*c5*(c3*s4 - c4*s3))/2305843009213693952 + 295*m7*(295*c3*s4 - 295*c4*s3) + (943793072886211*s5*(c3*s4 - c4*s3))/2305843009213693952) + (7775400025877285*c3*c4)/2361183241434822606848 + (1883354923850515*c3*s4)/1152921504606846976 - (5813615622121687*s3*s4)/288230376151711744 + (943793072886211*c5*(c3*s4 - c4*s3))/2305843009213693952 + 90*m6*(295*c3*s4 - 295*c4*s3) - 295*m6*(90*s5 + (7775400025877285*s3*s4)/2361183241434822606848 - c5*(295*c3*c4 + 295*s3*s4) + (8198078942807907*s5*(c3*s4 - c4*s3))/2305843009213693952 - 295*m7*s5*(c6*(90*c5 - 80*c5*(c3*s4 - c4*s3) + s5*(295*c3*c4 + 295*s3*s4)) - s6*(c5*(295*c3*c4 + 295*s3*s4) - 90*s5 + 80*s5*(c3*s4 - c4*s3)) + 80*s5*s6*(c3*s4 - c4*s3) + 80*c5*c6*(c3*s4 - c4*s3))) + 295*c5*m7*(c6*(c5*(295*c3*c4 + 295*s3*s4) - 90*s5 + 80*s5*(c3*s4 - c4*s3)) + s6*(90*c5 - 80*c5*(c3*s4 - c4*s3) + s5*(295*c3*c4 + 295*s3*s4)) + 80*c5*s6*(c3*s4 - c4*s3) - 80*c6*s5*(c3*s4 - c4*s3)) + 90*c5*m7*(c6*(90*c5 - 80*c5*(c3*s4 - c4*s3) + s5*(295*c3*c4 + 295*s3*s4)) - s6*(c5*(295*c3*c4 + 295*s3*s4) - 90*s5 + 80*s5*(c3*s4 - c4*s3)) + 80*s5*s6*(c3*s4 - c4*s3) + 80*c5*c6*(c3*s4 - c4*s3)) + 90*m7*s5*(c6*(c5*(295*c3*c4 + 295*s3*s4) - 90*s5 + 80*s5*(c3*s4 - c4*s3)) + s6*(90*c5 - 80*c5*(c3*s4 - c4*s3) + s5*(295*c3*c4 + 295*s3*s4)) + 80*c5*s6*(c3*s4 - c4*s3) - 80*c6*s5*(c3*s4 - c4*s3))) - s3*((1883354923850515*c3*c4)/1152921504606846976 - (1369254254579395*c3*s4)/144115188075855872 + (1369254254579395*c4*s3)/144115188075855872 + (1883354923850515*s3*s4)/1152921504606846976 - s4*((7775400025877285*c3*c4)/2361183241434822606848 + 295*c5*m7*(c6*(c5*(295*c3*c4 + 295*s3*s4) - 90*s5 + 80*s5*(c3*s4 - c4*s3)) + s6*(90*c5 - 80*c5*(c3*s4 - c4*s3) + s5*(295*c3*c4 + 295*s3*s4)) - (7775400025877285*s3*s4)/2361183241434822606848 + 295*m6*(90*s5 - c5*(295*c3*c4 + 295*s3*s4)) - (943793072886211*c5*(c3*s4 - c4*s3))/2305843009213693952 - (8198078942807907*s5*(c3*s4 - c4*s3))/2305843009213693952 + 295*m7*s5*(c6*(90*c5 - 80*c5*(c3*s4 - c4*s3) + s5*(295*c3*c4 + 295*s3*s4)) - s6*(c5*(295*c3*c4 + 295*s3*s4) - 90*s5 + 80*s5*(c3*s4 - c4*s3)) + 80*s5*s6*(c3*s4 - c4*s3) + 80*c5*c6*(c3*s4 - c4*s3)) + 80*c5*s6*(c3*s4 - c4*s3) - 80*c6*s5*(c3*s4 - c4*s3))) - c4*(c5*((1831324867619693*s5*s6*(c3*s4 - c4*s3))/295147905179352825856 + (1831324867619693*c5*c6*(c3*s4 - c4*s3))/295147905179352825856) + s5*((7115472921728667*c5*s6*(c3*s4 - c4*s3))/2361183241434822606848 - (7115472921728667*c6*s5*(c3*s4 - c4*s3))/2361183241434822606848) - 295*m6*(90*c5 + s5*(295*c3*c4 + 295*s3*s4)) + (3495819410978605*c5*(c3*s4 - c4*s3))/2305843009213693952 + 295*m7*(295*c3*s4 - 295*c4*s3) + (943793072886211*s5*(c3*s4 - c4*s3))/2305843009213693952)) + 270*c5*m7*(c6*(90*c5 - 80*c5*(c3*s4 - c4*s3) + s5*(295*c3*c4 + 295*s3*s4)) - s6*(c5*(295*c3*c4 + 295*s3*s4) - 90*s5 + 80*s5*(c3*s4 - c4*s3)) + 80*s5*s6*(c3*s4 - c4*s3) + 80*c5*c6*(c3*s4 - c4*s3)) + 270*m7*s5*(c6*(c5*(295*c3*c4 + 295*s3*s4) - 90*s5 + 80*s5*(c3*s4 - c4*s3)) + s6*(90*c5 - 80*c5*(c3*s4 - c4*s3) + s5*(295*c3*c4 + 295*s3*s4)) + 80*c5*s6*(c3*s4 - c4*s3) - 80*c6*s5*(c3*s4 - c4*s3))));
%  
% m23 = c3*qdd(3)*(24300*m4 + s3*(295*c5*m7*s4*((8198078942807907*c5)/2305843009213693952 - (943793072886211*s5)/2305843009213693952) - c4*((943793072886211*c5)/2305843009213693952 - (3495819410978605*s5)/2305843009213693952 + c5*((1831324867619693*c5*s6)/295147905179352825856 - (1831324867619693*c6*s5)/295147905179352825856) - s5*((7115472921728667*c5*c6)/2361183241434822606848 + (7115472921728667*s5*s6)/2361183241434822606848)) + 4965898922391233/590295810358705651712) - c4*((8198078942807907*c5)/2305843009213693952 + s4*((943793072886211*c5)/2305843009213693952 - (3495819410978605*s5)/2305843009213693952 + c5*((1831324867619693*c5*s6)/295147905179352825856 - (1831324867619693*c6*s5)/295147905179352825856) - s5*((7115472921728667*c5*c6)/2361183241434822606848 + (7115472921728667*s5*s6)/2361183241434822606848)) + (278418956501432245*m6*s5)/2305843009213693952 + 397124457897871/147573952589676412928) + 7478065051662123/36028797018963968);
%  
% m24 = -c3*qdd(4)*(s3*(295*c5*m7*s4*((8198078942807907*c5)/2305843009213693952 - (943793072886211*s5)/2305843009213693952) - c4*((943793072886211*c5)/2305843009213693952 - (3495819410978605*s5)/2305843009213693952 + c5*((1831324867619693*c5*s6)/295147905179352825856 - (1831324867619693*c6*s5)/295147905179352825856) - s5*((7115472921728667*c5*c6)/2361183241434822606848 + (7115472921728667*s5*s6)/2361183241434822606848)) + 4965898922391233/590295810358705651712) - c4*((8198078942807907*c5)/2305843009213693952 + s4*((943793072886211*c5)/2305843009213693952 - (3495819410978605*s5)/2305843009213693952 + c5*((1831324867619693*c5*s6)/295147905179352825856 - (1831324867619693*c6*s5)/295147905179352825856) - s5*((7115472921728667*c5*c6)/2361183241434822606848 + (7115472921728667*s5*s6)/2361183241434822606848)) + (278418956501432245*m6*s5)/2305843009213693952 + 397124457897871/147573952589676412928));
%  
% m25 = -c3*qdd(5)*((2293743007633799075*c4*m6)/2361183241434822606848 + (2293743007633799075*c5*m7*s3*s4)/2361183241434822606848);
% 
% m26 = c3*qdd(6)*((2293743007633799075*c4*m6)/2361183241434822606848 + (2293743007633799075*c5*m7*s3*s4)/2361183241434822606848);
%  
% 
% m31 = qdd1*((1035355510473309*c3*c4)/288230376151711744 + (4965898922391233*c3*s4)/590295810358705651712 - (4965898922391233*c4*s3)/590295810358705651712 + (1035355510473309*s3*s4)/288230376151711744 - s5*((1831324867619693*s5*s6*(c3*s4 - c4*s3))/295147905179352825856 + (1831324867619693*c5*c6*(c3*s4 - c4*s3))/295147905179352825856) + 90*c4*(m7*(s4*(295*c3 - 270*c3*s2) - c4*(295*s3 - 270*s2*s3)) - m6*(s5*(c4*(295*c3 - 270*c3*s2) + s4*(295*s3 - 270*s2*s3)) + c5*(270*c2 + 90))) + c5*((7115472921728667*c5*s6*(c3*s4 - c4*s3))/2361183241434822606848 - (7115472921728667*c6*s5*(c3*s4 - c4*s3))/2361183241434822606848) + 90*s4*(m6*(c5*(c4*(295*c3 - 270*c3*s2) + s4*(295*s3 - 270*s2*s3)) - s5*(270*c2 + 90)) - m7*s5*(c6*(s5*(c4*(295*c3 - 270*c3*s2) + s4*(295*s3 - 270*s2*s3)) - 80*c5*(c3*s4 - c4*s3) + c5*(270*c2 + 90)) - s6*(c5*(c4*(295*c3 - 270*c3*s2) + s4*(295*s3 - 270*s2*s3)) + 80*s5*(c3*s4 - c4*s3) - s5*(270*c2 + 90)) + 80*s5*s6*(c3*s4 - c4*s3) + 80*c5*c6*(c3*s4 - c4*s3)) + c5*m7*(s6*(s5*(c4*(295*c3 - 270*c3*s2) + s4*(295*s3 - 270*s2*s3)) - 80*c5*(c3*s4 - c4*s3) + c5*(270*c2 + 90)) + c6*(c5*(c4*(295*c3 - 270*c3*s2) + s4*(295*s3 - 270*s2*s3)) + 80*s5*(c3*s4 - c4*s3) - s5*(270*c2 + 90)) + 80*c5*s6*(c3*s4 - c4*s3) - 80*c6*s5*(c3*s4 - c4*s3))) + 90*m5*(s4*(295*c3 - 270*c3*s2) - 295*c3*s4 + 295*c4*s3 - c4*(295*s3 - 270*s2*s3)));
%  
% m32 = qdd(2)*((1035355510473309*c3*c4)/288230376151711744 + (4965898922391233*c3*s4)/590295810358705651712 - (4965898922391233*c4*s3)/590295810358705651712 - 90*c4*(m6*(90*c5 + s5*(295*c3*c4 + 295*s3*s4)) - m7*(295*c3*s4 - 295*c4*s3)) + (1035355510473309*s3*s4)/288230376151711744 - s5*((1831324867619693*s5*s6*(c3*s4 - c4*s3))/295147905179352825856 + (1831324867619693*c5*c6*(c3*s4 - c4*s3))/295147905179352825856) - 90*s4*(m6*(90*s5 - c5*(295*c3*c4 + 295*s3*s4)) - c5*m7*(c6*(c5*(295*c3*c4 + 295*s3*s4) - 90*s5 + 80*s5*(c3*s4 - c4*s3)) + s6*(90*c5 - 80*c5*(c3*s4 - c4*s3) + s5*(295*c3*c4 + 295*s3*s4)) + 80*c5*s6*(c3*s4 - c4*s3) - 80*c6*s5*(c3*s4 - c4*s3)) + m7*s5*(c6*(90*c5 - 80*c5*(c3*s4 - c4*s3) + s5*(295*c3*c4 + 295*s3*s4)) - s6*(c5*(295*c3*c4 + 295*s3*s4) - 90*s5 + 80*s5*(c3*s4 - c4*s3)) + 80*s5*s6*(c3*s4 - c4*s3) + 80*c5*c6*(c3*s4 - c4*s3))) + c5*((7115472921728667*c5*s6*(c3*s4 - c4*s3))/2361183241434822606848 - (7115472921728667*c6*s5*(c3*s4 - c4*s3))/2361183241434822606848));
%  
% m33 = -qdd(3)*(s5*((1831324867619693*c5*s6)/295147905179352825856 - (1831324867619693*c6*s5)/295147905179352825856) + c5*((7115472921728667*c5*c6)/2361183241434822606848 + (7115472921728667*s5*s6)/2361183241434822606848) + 869375736758729/36028797018963968);
%  
% m34 = qdd(4)*(s5*((1831324867619693*c5*s6)/295147905179352825856 - (1831324867619693*c6*s5)/295147905179352825856) + c5*((7115472921728667*c5*c6)/2361183241434822606848 + (7115472921728667*s5*s6)/2361183241434822606848) + 869375736758729/36028797018963968);
% 
% m35 = -(8276639014131817*qdd(5))/2305843009213693952;
%  
% m36 = 0;
% 
% m41 = -qdd1*((8276639014131817*c3*c4)/2305843009213693952 + (8276639014131817*s3*s4)/2305843009213693952 - s5*((1831324867619693*s5*s6*(c3*s4 - c4*s3))/295147905179352825856 + (1831324867619693*c5*c6*(c3*s4 - c4*s3))/295147905179352825856) + c5*((7115472921728667*c5*s6*(c3*s4 - c4*s3))/2361183241434822606848 - (7115472921728667*c6*s5*(c3*s4 - c4*s3))/2361183241434822606848));
% 
% m42 = -qdd(2)*((8276639014131817*c3*c4)/2305843009213693952 + (8276639014131817*s3*s4)/2305843009213693952 - s5*((1831324867619693*s5*s6*(c3*s4 - c4*s3))/295147905179352825856 + (1831324867619693*c5*c6*(c3*s4 - c4*s3))/295147905179352825856) + c5*((7115472921728667*c5*s6*(c3*s4 - c4*s3))/2361183241434822606848 - (7115472921728667*c6*s5*(c3*s4 - c4*s3))/2361183241434822606848));
%  
% m43 = qdd(3)*(s5*((1831324867619693*c5*s6)/295147905179352825856 - (1831324867619693*c6*s5)/295147905179352825856) + c5*((7115472921728667*c5*c6)/2361183241434822606848 + (7115472921728667*s5*s6)/2361183241434822606848));
%  
% m44 = -qdd(4)*(s5*((1831324867619693*c5*s6)/295147905179352825856 - (1831324867619693*c6*s5)/295147905179352825856) + c5*((7115472921728667*c5*c6)/2361183241434822606848 + (7115472921728667*s5*s6)/2361183241434822606848));
%  
% m45 = (8276639014131817*qdd(5))/2305843009213693952;
%  
% m46 = 0;
% 
% m51 = qdd1*((7775400025877285*c3*c4)/2361183241434822606848 + (7775400025877285*s3*s4)/2361183241434822606848);
% 
% m52 = qdd(2)*((7775400025877285*c3*c4)/2361183241434822606848 + (7775400025877285*s3*s4)/2361183241434822606848);
%  
% m53 = 0;
% m54 = 0;
% m55 = -(7775400025877285*qdd(5))/2361183241434822606848;
%  
% m56 = (7775400025877285*qdd(6))/2361183241434822606848;
m11 =  -((8581632868960513*c3)/1152921504606846976 + 75*c2*(m6*(s4*(295*c3 - 270*c3*s2) - c4*(295*s3 - 270*s2*s3)) + m5*(270*c2 + 90) + m7*s5*(s6*(s5*(c4*(295*c3 - 270*c3*s2) + s4*(295*s3 - 270*s2*s3)) - 80*c5*(c3*s4 - c4*s3) + c5*(270*c2 + 90)) + c6*(c5*(c4*(295*c3 - 270*c3*s2) + s4*(295*s3 - 270*s2*s3)) + 80*s5*(c3*s4 - c4*s3) - s5*(270*c2 + 90)) + 80*c5*s6*(c3*s4 - c4*s3) - 80*c6*s5*(c3*s4 - c4*s3)) + 270*m4*s2*s3 + c5*m7*(c6*(s5*(c4*(295*c3 - 270*c3*s2) + s4*(295*s3 - 270*s2*s3)) - 80*c5*(c3*s4 - c4*s3) + c5*(270*c2 + 90)) - s6*(c5*(c4*(295*c3 - 270*c3*s2) + s4*(295*s3 - 270*s2*s3)) + 80*s5*(c3*s4 - c4*s3) - s5*(270*c2 + 90)) + 80*s5*s6*(c3*s4 - c4*s3) + 80*c5*c6*(c3*s4 - c4*s3))) - 335*c2*(c3*(c4*(m6*(c5*(c4*(295*c3 - 270*c3*s2) + s4*(295*s3 - 270*s2*s3)) - s5*(270*c2 + 90)) - m7*s5*(c6*(s5*(c4*(295*c3 - 270*c3*s2) + s4*(295*s3 - 270*s2*s3)) - 80*c5*(c3*s4 - c4*s3) + c5*(270*c2 + 90)) - s6*(c5*(c4*(295*c3 - 270*c3*s2) + s4*(295*s3 - 270*s2*s3)) + 80*s5*(c3*s4 - c4*s3) - s5*(270*c2 + 90)) + 80*s5*s6*(c3*s4 - c4*s3) + 80*c5*c6*(c3*s4 - c4*s3)) + c5*m7*(s6*(s5*(c4*(295*c3 - 270*c3*s2) + s4*(295*s3 - 270*s2*s3)) - 80*c5*(c3*s4 - c4*s3) + c5*(270*c2 + 90)) + c6*(c5*(c4*(295*c3 - 270*c3*s2) + s4*(295*s3 - 270*s2*s3)) + 80*s5*(c3*s4 - c4*s3) - s5*(270*c2 + 90)) + 80*c5*s6*(c3*s4 - c4*s3) - 80*c6*s5*(c3*s4 - c4*s3))) - s4*(m7*(s4*(295*c3 - 270*c3*s2) - c4*(295*s3 - 270*s2*s3)) - m6*(s5*(c4*(295*c3 - 270*c3*s2) + s4*(295*s3 - 270*s2*s3)) + c5*(270*c2 + 90))) + m5*(c4*(295*c3 - 270*c3*s2) - 295*c3*c4 - 295*s3*s4 + s4*(295*s3 - 270*s2*s3))) + s3*(c4*(m7*(s4*(295*c3 - 270*c3*s2) - c4*(295*s3 - 270*s2*s3)) - m6*(s5*(c4*(295*c3 - 270*c3*s2) + s4*(295*s3 - 270*s2*s3)) + c5*(270*c2 + 90))) + s4*(m6*(c5*(c4*(295*c3 - 270*c3*s2) + s4*(295*s3 - 270*s2*s3)) - s5*(270*c2 + 90)) - m7*s5*(c6*(s5*(c4*(295*c3 - 270*c3*s2) + s4*(295*s3 - 270*s2*s3)) - 80*c5*(c3*s4 - c4*s3) + c5*(270*c2 + 90)) - s6*(c5*(c4*(295*c3 - 270*c3*s2) + s4*(295*s3 - 270*s2*s3)) + 80*s5*(c3*s4 - c4*s3) - s5*(270*c2 + 90)) + 80*s5*s6*(c3*s4 - c4*s3) + 80*c5*c6*(c3*s4 - c4*s3)) + c5*m7*(s6*(s5*(c4*(295*c3 - 270*c3*s2) + s4*(295*s3 - 270*s2*s3)) - 80*c5*(c3*s4 - c4*s3) + c5*(270*c2 + 90)) + c6*(c5*(c4*(295*c3 - 270*c3*s2) + s4*(295*s3 - 270*s2*s3)) + 80*s5*(c3*s4 - c4*s3) - s5*(270*c2 + 90)) + 80*c5*s6*(c3*s4 - c4*s3) - 80*c6*s5*(c3*s4 - c4*s3))) + m5*(s4*(295*c3 - 270*c3*s2) - 295*c3*s4 + 295*c4*s3 - c4*(295*s3 - 270*s2*s3))) - 270*c3*m4*s2) - c3*(s4*(c5*((1831324867619693*s5*s6*(c3*s4 - c4*s3))/295147905179352825856 + (1831324867619693*c5*c6*(c3*s4 - c4*s3))/295147905179352825856) + s5*((7115472921728667*c5*s6*(c3*s4 - c4*s3))/2361183241434822606848 - (7115472921728667*c6*s5*(c3*s4 - c4*s3))/2361183241434822606848) + (3495819410978605*c5*(c3*s4 - c4*s3))/2305843009213693952 + 295*m7*(s4*(295*c3 - 270*c3*s2) - c4*(295*s3 - 270*s2*s3)) + (943793072886211*s5*(c3*s4 - c4*s3))/2305843009213693952 - 295*m6*(s5*(c4*(295*c3 - 270*c3*s2) + s4*(295*s3 - 270*s2*s3)) + c5*(270*c2 + 90))) - c4*((7775400025877285*c3*c4)/2361183241434822606848 + (7775400025877285*s3*s4)/2361183241434822606848 + (943793072886211*c5*(c3*s4 - c4*s3))/2305843009213693952 + (8198078942807907*s5*(c3*s4 - c4*s3))/2305843009213693952 + 295*m6*(c5*(c4*(295*c3 - 270*c3*s2) + s4*(295*s3 - 270*s2*s3)) - s5*(270*c2 + 90)) - 295*m7*s5*(c6*(s5*(c4*(295*c3 - 270*c3*s2) + s4*(295*s3 - 270*s2*s3)) - 80*c5*(c3*s4 - c4*s3) + c5*(270*c2 + 90)) - s6*(c5*(c4*(295*c3 - 270*c3*s2) + s4*(295*s3 - 270*s2*s3)) + 80*s5*(c3*s4 - c4*s3) - s5*(270*c2 + 90)) + 80*s5*s6*(c3*s4 - c4*s3) + 80*c5*c6*(c3*s4 - c4*s3)) + 295*c5*m7*(s6*(s5*(c4*(295*c3 - 270*c3*s2) + s4*(295*s3 - 270*s2*s3)) - 80*c5*(c3*s4 - c4*s3) + c5*(270*c2 + 90)) + c6*(c5*(c4*(295*c3 - 270*c3*s2) + s4*(295*s3 - 270*s2*s3)) + 80*s5*(c3*s4 - c4*s3) - s5*(270*c2 + 90)) + 80*c5*s6*(c3*s4 - c4*s3) - 80*c6*s5*(c3*s4 - c4*s3))) - (5813615622121687*c3*c4)/288230376151711744 + (1883354923850515*c3*s4)/1152921504606846976 - (1883354923850515*c4*s3)/1152921504606846976 - (5813615622121687*s3*s4)/288230376151711744 + 90*m6*(s4*(295*c3 - 270*c3*s2) - c4*(295*s3 - 270*s2*s3)) + 90*m5*(270*c2 + 90) + 90*m7*s5*(s6*(s5*(c4*(295*c3 - 270*c3*s2) + s4*(295*s3 - 270*s2*s3)) - 80*c5*(c3*s4 - c4*s3) + c5*(270*c2 + 90)) + c6*(c5*(c4*(295*c3 - 270*c3*s2) + s4*(295*s3 - 270*s2*s3)) + 80*s5*(c3*s4 - c4*s3) - s5*(270*c2 + 90)) + 80*c5*s6*(c3*s4 - c4*s3) - 80*c6*s5*(c3*s4 - c4*s3)) + 90*c5*m7*(c6*(s5*(c4*(295*c3 - 270*c3*s2) + s4*(295*s3 - 270*s2*s3)) - 80*c5*(c3*s4 - c4*s3) + c5*(270*c2 + 90)) - s6*(c5*(c4*(295*c3 - 270*c3*s2) + s4*(295*s3 - 270*s2*s3)) + 80*s5*(c3*s4 - c4*s3) - s5*(270*c2 + 90)) + 80*s5*s6*(c3*s4 - c4*s3) + 80*c5*c6*(c3*s4 - c4*s3))) + 270*c5*m7*((7145951600741313*s3)/288230376151711744 + 90450*m3*s2 + 335*s2*(m6*(s4*(295*c3 - 270*c3*s2) - c4*(295*s3 - 270*s2*s3)) + m5*(270*c2 + 90) + m7*s5*(s6*(s5*(c4*(295*c3 - 270*c3*s2) + s4*(295*s3 - 270*s2*s3)) - 80*c5*(c3*s4 - c4*s3) + c5*(270*c2 + 90)) + c6*(c5*(c4*(295*c3 - 270*c3*s2) + s4*(295*s3 - 270*s2*s3)) + 80*s5*(c3*s4 - c4*s3) - s5*(270*c2 + 90)) + 80*c5*s6*(c3*s4 - c4*s3) - 80*c6*s5*(c3*s4 - c4*s3)) + 270*m4*s2*s3 + c5*m7*(c6*(s5*(c4*(295*c3 - 270*c3*s2) + s4*(295*s3 - 270*s2*s3)) - 80*c5*(c3*s4 - c4*s3) + c5*(270*c2 + 90)) - s6*(c5*(c4*(295*c3 - 270*c3*s2) + s4*(295*s3 - 270*s2*s3)) + 80*s5*(c3*s4 - c4*s3) - s5*(270*c2 + 90)) + 80*s5*s6*(c3*s4 - c4*s3) + 80*c5*c6*(c3*s4 - c4*s3))) + s3*(c4*(c5*((1831324867619693*s5*s6*(c3*s4 - c4*s3))/295147905179352825856 + (1831324867619693*c5*c6*(c3*s4 - c4*s3))/295147905179352825856) + s5*((7115472921728667*c5*s6*(c3*s4 - c4*s3))/2361183241434822606848 - (7115472921728667*c6*s5*(c3*s4 - c4*s3))/2361183241434822606848) + (3495819410978605*c5*(c3*s4 - c4*s3))/2305843009213693952 + 295*m7*(s4*(295*c3 - 270*c3*s2) - c4*(295*s3 - 270*s2*s3)) + (943793072886211*s5*(c3*s4 - c4*s3))/2305843009213693952 - 295*m6*(s5*(c4*(295*c3 - 270*c3*s2) + s4*(295*s3 - 270*s2*s3)) + c5*(270*c2 + 90))) - (1883354923850515*c3*c4)/1152921504606846976 + s4*((7775400025877285*c3*c4)/2361183241434822606848 + (7775400025877285*s3*s4)/2361183241434822606848 + (943793072886211*c5*(c3*s4 - c4*s3))/2305843009213693952 + (8198078942807907*s5*(c3*s4 - c4*s3))/2305843009213693952 + 295*m6*(c5*(c4*(295*c3 - 270*c3*s2) + s4*(295*s3 - 270*s2*s3)) - s5*(270*c2 + 90)) - 295*m7*s5*(c6*(s5*(c4*(295*c3 - 270*c3*s2) + s4*(295*s3 - 270*s2*s3)) - 80*c5*(c3*s4 - c4*s3) + c5*(270*c2 + 90)) - s6*(c5*(c4*(295*c3 - 270*c3*s2) + s4*(295*s3 - 270*s2*s3)) + 80*s5*(c3*s4 - c4*s3) - s5*(270*c2 + 90)) + 80*s5*s6*(c3*s4 - c4*s3) + 80*c5*c6*(c3*s4 - c4*s3)) + 295*c5*m7*(s6*(s5*(c4*(295*c3 - 270*c3*s2) + s4*(295*s3 - 270*s2*s3)) - 80*c5*(c3*s4 - c4*s3) + c5*(270*c2 + 90)) + c6*(c5*(c4*(295*c3 - 270*c3*s2) + s4*(295*s3 - 270*s2*s3)) + 80*s5*(c3*s4 - c4*s3) - s5*(270*c2 + 90)) + 80*c5*s6*(c3*s4 - c4*s3) - 80*c6*s5*(c3*s4 - c4*s3))) + (1369254254579395*c3*s4)/144115188075855872 - (1369254254579395*c4*s3)/144115188075855872 - (1883354923850515*s3*s4)/1152921504606846976) + 270*m6*(s4*(295*c3 - 270*c3*s2) - c4*(295*s3 - 270*s2*s3)) + 75*s2*(c3*(c4*(m6*(c5*(c4*(295*c3 - 270*c3*s2) + s4*(295*s3 - 270*s2*s3)) - s5*(270*c2 + 90)) - m7*s5*(c6*(s5*(c4*(295*c3 - 270*c3*s2) + s4*(295*s3 - 270*s2*s3)) - 80*c5*(c3*s4 - c4*s3) + c5*(270*c2 + 90)) - s6*(c5*(c4*(295*c3 - 270*c3*s2) + s4*(295*s3 - 270*s2*s3)) + 80*s5*(c3*s4 - c4*s3) - s5*(270*c2 + 90)) + 80*s5*s6*(c3*s4 - c4*s3) + 80*c5*c6*(c3*s4 - c4*s3)) + c5*m7*(s6*(s5*(c4*(295*c3 - 270*c3*s2) + s4*(295*s3 - 270*s2*s3)) - 80*c5*(c3*s4 - c4*s3) + c5*(270*c2 + 90)) + c6*(c5*(c4*(295*c3 - 270*c3*s2) + s4*(295*s3 - 270*s2*s3)) + 80*s5*(c3*s4 - c4*s3) - s5*(270*c2 + 90)) + 80*c5*s6*(c3*s4 - c4*s3) - 80*c6*s5*(c3*s4 - c4*s3))) - s4*(m7*(s4*(295*c3 - 270*c3*s2) - c4*(295*s3 - 270*s2*s3)) - m6*(s5*(c4*(295*c3 - 270*c3*s2) + s4*(295*s3 - 270*s2*s3)) + c5*(270*c2 + 90))) + m5*(c4*(295*c3 - 270*c3*s2) - 295*c3*c4 - 295*s3*s4 + s4*(295*s3 - 270*s2*s3))) + s3*(c4*(m7*(s4*(295*c3 - 270*c3*s2) - c4*(295*s3 - 270*s2*s3)) - m6*(s5*(c4*(295*c3 - 270*c3*s2) + s4*(295*s3 - 270*s2*s3)) + c5*(270*c2 + 90))) + s4*(m6*(c5*(c4*(295*c3 - 270*c3*s2) + s4*(295*s3 - 270*s2*s3)) - s5*(270*c2 + 90)) - m7*s5*(c6*(s5*(c4*(295*c3 - 270*c3*s2) + s4*(295*s3 - 270*s2*s3)) - 80*c5*(c3*s4 - c4*s3) + c5*(270*c2 + 90)) - s6*(c5*(c4*(295*c3 - 270*c3*s2) + s4*(295*s3 - 270*s2*s3)) + 80*s5*(c3*s4 - c4*s3) - s5*(270*c2 + 90)) + 80*s5*s6*(c3*s4 - c4*s3) + 80*c5*c6*(c3*s4 - c4*s3)) + c5*m7*(s6*(s5*(c4*(295*c3 - 270*c3*s2) + s4*(295*s3 - 270*s2*s3)) - 80*c5*(c3*s4 - c4*s3) + c5*(270*c2 + 90)) + c6*(c5*(c4*(295*c3 - 270*c3*s2) + s4*(295*s3 - 270*s2*s3)) + 80*s5*(c3*s4 - c4*s3) - s5*(270*c2 + 90)) + 80*c5*s6*(c3*s4 - c4*s3) - 80*c6*s5*(c3*s4 - c4*s3))) + m5*(s4*(295*c3 - 270*c3*s2) - 295*c3*s4 + 295*c4*s3 - c4*(295*s3 - 270*s2*s3))) - 270*c3*m4*s2) - c6*(80*c5*(c3*s4 - c4*s3) - s6*(c5*(c4*(295*c3 - 270*c3*s2) + s4*(295*s3 - 270*s2*s3)) + 80*s5*(c3*s4 - c4*s3) - s5*(270*c2 + 90)) + c5*(s5*(c4*(295*c3 - 270*c3*s2) + s4*(295*s3 - 270*s2*s3)) - 270*c2 + 26550*c3^2) + 80*s5*s6*(c3*s4 - c4*s3)) + 270*m5*(270*c2 + 90) - 75*m3*(270*c2 + 270) + 270*m7*s5*(s6*(s5*(c4*(295*c3 - 270*c3*s2) + s4*(295*s3 - 270*s2*s3)) - 80*c5*(c3*s4 - c4*s3) + c5*(270*c2 + 90)) + c6*(c5*(c4*(295*c3 - 270*c3*s2) + s4*(295*s3 - 270*s2*s3)) + 80*s5*(c3*s4 - c4*s3) - s5*(270*c2 + 90)) + 80*c5*s6*(c3*s4 - c4*s3) - 80*c6*s5*(c3*s4 - c4*s3)) + 72900*m4*s2*s3 + 80*c5*c6*(c3*s4 - c4*s3) - 6288408585614741/144115188075855872))

m12 = -((8581632868960513*c3)/1152921504606846976 + 75*c2*(90*m5 + m6*(295*c3*s4 - 295*c4*s3) + c5*m7*(c6*(90*c5 - 80*c5*(c3*s4 - c4*s3) + s5*(295*c3*c4 + 295*s3*s4)) - s6*(c5*(295*c3*c4 + 295*s3*s4) - 90*s5 + 80*s5*(c3*s4 - c4*s3)) + 80*s5*s6*(c3*s4 - c4*s3) + 80*c5*c6*(c3*s4 - c4*s3)) + m7*s5*(c6*(c5*(295*c3*c4 + 295*s3*s4) - 90*s5 + 80*s5*(c3*s4 - c4*s3)) + s6*(90*c5 - 80*c5*(c3*s4 - c4*s3) + s5*(295*c3*c4 + 295*s3*s4)) + 80*c5*s6*(c3*s4 - c4*s3) - 80*c6*s5*(c3*s4 - c4*s3))) + 335*c2*(c3*(c4*(m6*(90*s5 - c5*(295*c3*c4 + 295*s3*s4)) - c5*m7*(c6*(c5*(295*c3*c4 + 295*s3*s4) - 90*s5 + 80*s5*(c3*s4 - c4*s3)) + s6*(90*c5 - 80*c5*(c3*s4 - c4*s3) + s5*(295*c3*c4 + 295*s3*s4)) + 80*c5*s6*(c3*s4 - c4*s3) - 80*c6*s5*(c3*s4 - c4*s3)) + m7*s5*(c6*(90*c5 - 80*c5*(c3*s4 - c4*s3) + s5*(295*c3*c4 + 295*s3*s4)) - s6*(c5*(295*c3*c4 + 295*s3*s4) - 90*s5 + 80*s5*(c3*s4 - c4*s3)) + 80*s5*s6*(c3*s4 - c4*s3) + 80*c5*c6*(c3*s4 - c4*s3))) - s4*(m6*(90*c5 + s5*(295*c3*c4 + 295*s3*s4)) - m7*(295*c3*s4 - 295*c4*s3))) + s3*(c4*(m6*(90*c5 + s5*(295*c3*c4 + 295*s3*s4)) - m7*(295*c3*s4 - 295*c4*s3)) + s4*(m6*(90*s5 - c5*(295*c3*c4 + 295*s3*s4)) - c5*m7*(c6*(c5*(295*c3*c4 + 295*s3*s4) - 90*s5 + 80*s5*(c3*s4 - c4*s3)) + s6*(90*c5 - 80*c5*(c3*s4 - c4*s3) + s5*(295*c3*c4 + 295*s3*s4)) + 80*c5*s6*(c3*s4 - c4*s3) - 80*c6*s5*(c3*s4 - c4*s3)) + m7*s5*(c6*(90*c5 - 80*c5*(c3*s4 - c4*s3) + s5*(295*c3*c4 + 295*s3*s4)) - s6*(c5*(295*c3*c4 + 295*s3*s4) - 90*s5 + 80*s5*(c3*s4 - c4*s3)) + 80*s5*s6*(c3*s4 - c4*s3) + 80*c5*c6*(c3*s4 - c4*s3))))) - c3*(8100*m5 + s4*(c5*((1831324867619693*s5*s6*(c3*s4 - c4*s3))/295147905179352825856 + (1831324867619693*c5*c6*(c3*s4 - c4*s3))/295147905179352825856) + s5*((7115472921728667*c5*s6*(c3*s4 - c4*s3))/2361183241434822606848 - (7115472921728667*c6*s5*(c3*s4 - c4*s3))/2361183241434822606848) - 295*m6*(90*c5 + s5*(295*c3*c4 + 295*s3*s4)) + (3495819410978605*c5*(c3*s4 - c4*s3))/2305843009213693952 + 295*m7*(295*c3*s4 - 295*c4*s3) + (943793072886211*s5*(c3*s4 - c4*s3))/2305843009213693952) - (5813615622121687*c3*c4)/288230376151711744 + (1883354923850515*c3*s4)/1152921504606846976 - (1883354923850515*c4*s3)/1152921504606846976 - (5813615622121687*s3*s4)/288230376151711744 + 90*m6*(295*c3*s4 - 295*c4*s3) - c4*((7775400025877285*c3*c4)/2361183241434822606848 + (7775400025877285*s3*s4)/2361183241434822606848 - 295*m6*(90*s5 - c5*(295*c3*c4 + 295*s3*s4)) + (943793072886211*c5*(c3*s4 - c4*s3))/2305843009213693952 + (8198078942807907*s5*(c3*s4 - c4*s3))/2305843009213693952 + 295*c5*m7*(c6*(c5*(295*c3*c4 + 295*s3*s4) - 90*s5 + 80*s5*(c3*s4 - c4*s3)) + s6*(90*c5 - 80*c5*(c3*s4 - c4*s3) + s5*(295*c3*c4 + 295*s3*s4)) + 80*c5*s6*(c3*s4 - c4*s3) - 80*c6*s5*(c3*s4 - c4*s3)) - 295*m7*s5*(c6*(90*c5 - 80*c5*(c3*s4 - c4*s3) + s5*(295*c3*c4 + 295*s3*s4)) - s6*(c5*(295*c3*c4 + 295*s3*s4) - 90*s5 + 80*s5*(c3*s4 - c4*s3)) + 80*s5*s6*(c3*s4 - c4*s3) + 80*c5*c6*(c3*s4 - c4*s3))) + 90*c5*m7*(c6*(90*c5 - 80*c5*(c3*s4 - c4*s3) + s5*(295*c3*c4 + 295*s3*s4)) - s6*(c5*(295*c3*c4 + 295*s3*s4) - 90*s5 + 80*s5*(c3*s4 - c4*s3)) + 80*s5*s6*(c3*s4 - c4*s3) + 80*c5*c6*(c3*s4 - c4*s3)) + 90*m7*s5*(c6*(c5*(295*c3*c4 + 295*s3*s4) - 90*s5 + 80*s5*(c3*s4 - c4*s3)) + s6*(90*c5 - 80*c5*(c3*s4 - c4*s3) + s5*(295*c3*c4 + 295*s3*s4)) + 80*c5*s6*(c3*s4 - c4*s3) - 80*c6*s5*(c3*s4 - c4*s3))) + 270*c5*m7*(24300*m5 - 20250*m3 + (7145951600741313*s3)/288230376151711744 + 335*s2*(90*m5 + m6*(295*c3*s4 - 295*c4*s3) + c5*m7*(c6*(90*c5 - 80*c5*(c3*s4 - c4*s3) + s5*(295*c3*c4 + 295*s3*s4)) - s6*(c5*(295*c3*c4 + 295*s3*s4) - 90*s5 + 80*s5*(c3*s4 - c4*s3)) + 80*s5*s6*(c3*s4 - c4*s3) + 80*c5*c6*(c3*s4 - c4*s3)) + m7*s5*(c6*(c5*(295*c3*c4 + 295*s3*s4) - 90*s5 + 80*s5*(c3*s4 - c4*s3)) + s6*(90*c5 - 80*c5*(c3*s4 - c4*s3) + s5*(295*c3*c4 + 295*s3*s4)) + 80*c5*s6*(c3*s4 - c4*s3) - 80*c6*s5*(c3*s4 - c4*s3))) + 270*m6*(295*c3*s4 - 295*c4*s3) - c6*(80*c5*(c3*s4 - c4*s3) - s6*(c5*(295*c3*c4 + 295*s3*s4) - 90*s5 + 80*s5*(c3*s4 - c4*s3)) + c5*(s5*(295*c3*c4 + 295*s3*s4) + 26550*c3^2) + 80*s5*s6*(c3*s4 - c4*s3)) - 75*s2*(c3*(c4*(m6*(90*s5 - c5*(295*c3*c4 + 295*s3*s4)) - c5*m7*(c6*(c5*(295*c3*c4 + 295*s3*s4) - 90*s5 + 80*s5*(c3*s4 - c4*s3)) + s6*(90*c5 - 80*c5*(c3*s4 - c4*s3) + s5*(295*c3*c4 + 295*s3*s4)) + 80*c5*s6*(c3*s4 - c4*s3) - 80*c6*s5*(c3*s4 - c4*s3)) + m7*s5*(c6*(90*c5 - 80*c5*(c3*s4 - c4*s3) + s5*(295*c3*c4 + 295*s3*s4)) - s6*(c5*(295*c3*c4 + 295*s3*s4) - 90*s5 + 80*s5*(c3*s4 - c4*s3)) + 80*s5*s6*(c3*s4 - c4*s3) + 80*c5*c6*(c3*s4 - c4*s3))) - s4*(m6*(90*c5 + s5*(295*c3*c4 + 295*s3*s4)) - m7*(295*c3*s4 - 295*c4*s3))) + s3*(c4*(m6*(90*c5 + s5*(295*c3*c4 + 295*s3*s4)) - m7*(295*c3*s4 - 295*c4*s3)) + s4*(m6*(90*s5 - c5*(295*c3*c4 + 295*s3*s4)) - c5*m7*(c6*(c5*(295*c3*c4 + 295*s3*s4) - 90*s5 + 80*s5*(c3*s4 - c4*s3)) + s6*(90*c5 - 80*c5*(c3*s4 - c4*s3) + s5*(295*c3*c4 + 295*s3*s4)) + 80*c5*s6*(c3*s4 - c4*s3) - 80*c6*s5*(c3*s4 - c4*s3)) + m7*s5*(c6*(90*c5 - 80*c5*(c3*s4 - c4*s3) + s5*(295*c3*c4 + 295*s3*s4)) - s6*(c5*(295*c3*c4 + 295*s3*s4) - 90*s5 + 80*s5*(c3*s4 - c4*s3)) + 80*s5*s6*(c3*s4 - c4*s3) + 80*c5*c6*(c3*s4 - c4*s3))))) - s3*((1883354923850515*c3*c4)/1152921504606846976 - (1369254254579395*c3*s4)/144115188075855872 + (1369254254579395*c4*s3)/144115188075855872 + (1883354923850515*s3*s4)/1152921504606846976 - s4*((7775400025877285*c3*c4)/2361183241434822606848 + (7775400025877285*s3*s4)/2361183241434822606848 - 295*m6*(90*s5 - c5*(295*c3*c4 + 295*s3*s4)) + (943793072886211*c5*(c3*s4 - c4*s3))/2305843009213693952 + (8198078942807907*s5*(c3*s4 - c4*s3))/2305843009213693952 + 295*c5*m7*(c6*(c5*(295*c3*c4 + 295*s3*s4) - 90*s5 + 80*s5*(c3*s4 - c4*s3)) + s6*(90*c5 - 80*c5*(c3*s4 - c4*s3) + s5*(295*c3*c4 + 295*s3*s4)) + 80*c5*s6*(c3*s4 - c4*s3) - 80*c6*s5*(c3*s4 - c4*s3)) - 295*m7*s5*(c6*(90*c5 - 80*c5*(c3*s4 - c4*s3) + s5*(295*c3*c4 + 295*s3*s4)) - s6*(c5*(295*c3*c4 + 295*s3*s4) - 90*s5 + 80*s5*(c3*s4 - c4*s3)) + 80*s5*s6*(c3*s4 - c4*s3) + 80*c5*c6*(c3*s4 - c4*s3))) - c4*(c5*((1831324867619693*s5*s6*(c3*s4 - c4*s3))/295147905179352825856 + (1831324867619693*c5*c6*(c3*s4 - c4*s3))/295147905179352825856) + s5*((7115472921728667*c5*s6*(c3*s4 - c4*s3))/2361183241434822606848 - (7115472921728667*c6*s5*(c3*s4 - c4*s3))/2361183241434822606848) - 295*m6*(90*c5 + s5*(295*c3*c4 + 295*s3*s4)) + (3495819410978605*c5*(c3*s4 - c4*s3))/2305843009213693952 + 295*m7*(295*c3*s4 - 295*c4*s3) + (943793072886211*s5*(c3*s4 - c4*s3))/2305843009213693952)) + 270*m7*s5*(c6*(c5*(295*c3*c4 + 295*s3*s4) - 90*s5 + 80*s5*(c3*s4 - c4*s3)) + s6*(90*c5 - 80*c5*(c3*s4 - c4*s3) + s5*(295*c3*c4 + 295*s3*s4)) + 80*c5*s6*(c3*s4 - c4*s3) - 80*c6*s5*(c3*s4 - c4*s3)) + 80*c5*c6*(c3*s4 - c4*s3) - 6288408585614741/144115188075855872));
 
m13 = (6750*c2*m4 + c3*(s4*((943793072886211*c5)/2305843009213693952 - (3495819410978605*s5)/2305843009213693952 + c5*((1831324867619693*c5*s6)/295147905179352825856 - (1831324867619693*c6*s5)/295147905179352825856) - s5*((7115472921728667*c5*c6)/2361183241434822606848 + (7115472921728667*s5*s6)/2361183241434822606848)) - c4*((8198078942807907*c5)/2305843009213693952 - (943793072886211*s5)/2305843009213693952) + 397124457897871/147573952589676412928) + 270*c5*m7*(24300*m4 + 80*c6*s5 + 30150*m4*s2 - s3*(c4*((943793072886211*c5)/2305843009213693952 - (3495819410978605*s5)/2305843009213693952 + c5*((1831324867619693*c5*s6)/295147905179352825856 - (1831324867619693*c6*s5)/295147905179352825856) - s5*((7115472921728667*c5*c6)/2361183241434822606848 + (7115472921728667*s5*s6)/2361183241434822606848)) + s4*((8198078942807907*c5)/2305843009213693952 - (943793072886211*s5)/2305843009213693952) - 4965898922391233/590295810358705651712) + 80*c5*c6*s5 + 7478065051662123/36028797018963968));

m14 = -(c3*(s4*((943793072886211*c5)/2305843009213693952 - (3495819410978605*s5)/2305843009213693952 + c5*((1831324867619693*c5*s6)/295147905179352825856 - (1831324867619693*c6*s5)/295147905179352825856) - s5*((7115472921728667*c5*c6)/2361183241434822606848 + (7115472921728667*s5*s6)/2361183241434822606848)) - c4*((8198078942807907*c5)/2305843009213693952 - (943793072886211*s5)/2305843009213693952) + 397124457897871/147573952589676412928) + 270*c5*m7*(80*c6*s5 - s3*(c4*((943793072886211*c5)/2305843009213693952 - (3495819410978605*s5)/2305843009213693952 + c5*((1831324867619693*c5*s6)/295147905179352825856 - (1831324867619693*c6*s5)/295147905179352825856) - s5*((7115472921728667*c5*c6)/2361183241434822606848 + (7115472921728667*s5*s6)/2361183241434822606848)) + s4*((8198078942807907*c5)/2305843009213693952 - (943793072886211*s5)/2305843009213693952) - 4965898922391233/590295810358705651712) + 80*c5*c6*s5));
 
m15 = ((7775400025877285*c3*c4)/2361183241434822606848 + (1049679003493433475*c5*m7*s3*s4)/1180591620717411303424);
 
m16 = -((7775400025877285*c3*c4)/2361183241434822606848 + (1049679003493433475*c5*m7*s3*s4)/1180591620717411303424);
 

m21= -((8581632868960513*c3)/1152921504606846976 + c3*((7145951600741313*s3)/288230376151711744 + (5813615622121687*c3*c4)/288230376151711744 + (1883354923850515*c4*s3)/1152921504606846976 + 270*m6*(s4*(295*c3 - 270*c3*s2) - c4*(295*s3 - 270*s2*s3)) + s3*(c4*(c5*((1831324867619693*s5*s6*(c3*s4 - c4*s3))/295147905179352825856 + (1831324867619693*c5*c6*(c3*s4 - c4*s3))/295147905179352825856) + s5*((7115472921728667*c5*s6*(c3*s4 - c4*s3))/2361183241434822606848 - (7115472921728667*c6*s5*(c3*s4 - c4*s3))/2361183241434822606848) + (3495819410978605*c5*(c3*s4 - c4*s3))/2305843009213693952 + 295*m7*(s4*(295*c3 - 270*c3*s2) - c4*(295*s3 - 270*s2*s3)) + (943793072886211*s5*(c3*s4 - c4*s3))/2305843009213693952 - 295*m6*(s5*(c4*(295*c3 - 270*c3*s2) + s4*(295*s3 - 270*s2*s3)) + c5*(270*c2 + 90))) - (1883354923850515*c3*c4)/1152921504606846976 + (1369254254579395*c3*s4)/144115188075855872 - (1369254254579395*c4*s3)/144115188075855872 - (1883354923850515*s3*s4)/1152921504606846976 + s4*((7775400025877285*c3*c4)/2361183241434822606848 - 295*c5*m7*((7775400025877285*s3*s4)/2361183241434822606848 - c6*(c5*(c4*(295*c3 - 270*c3*s2) + s4*(295*s3 - 270*s2*s3)) + 80*s5*(c3*s4 - c4*s3) - s5*(270*c2 + 90)) + (943793072886211*c5*(c3*s4 - c4*s3))/2305843009213693952 - s6*(c5*(270*c2 + 90) - 80*c5*(c3*s4 - c4*s3) + s5*(c4*(295*c3 - 270*c3*s2) + s4*(295*s3 - 270*c2*s2*s3))) + (8198078942807907*s5*(c3*s4 - c4*s3))/2305843009213693952 + 295*m6*(c5*(c4*(295*c3 - 270*c3*s2) + s4*(295*s3 - 270*s2*s3)) - s5*(270*c2 + 90)) - 295*m7*s5*(c6*(s5*(c4*(295*c3 - 270*c3*s2) + s4*(295*s3 - 270*s2*s3)) - 80*c5*(c3*s4 - c4*s3) + c5*(270*c2 + 90)) - s6*(c5*(c4*(295*c3 - 270*c3*s2) + s4*(295*s3 - 270*s2*s3)) + 80*s5*(c3*s4 - c4*s3) - s5*(270*c2 + 90)) + 80*s5*s6*(c3*s4 - c4*s3) + 80*c5*c6*(c3*s4 - c4*s3)) - 80*c5*s6*(c3*s4 - c4*s3) + 80*c6*s5*(c3*s4 - c4*s3)))) + c4*(s4*(c5*((1831324867619693*s5*s6*(c3*s4 - c4*s3))/295147905179352825856 + (1831324867619693*c5*c6*(c3*s4 - c4*s3))/295147905179352825856) + s5*((7115472921728667*c5*s6*(c3*s4 - c4*s3))/2361183241434822606848 - (7115472921728667*c6*s5*(c3*s4 - c4*s3))/2361183241434822606848) + (3495819410978605*c5*(c3*s4 - c4*s3))/2305843009213693952 + 295*m7*(s4*(295*c3 - 270*c3*s2) - c4*(295*s3 - 270*s2*s3)) + (943793072886211*s5*(c3*s4 - c4*s3))/2305843009213693952 - 295*m6*(s5*(c4*(295*c3 - 270*c3*s2) + s4*(295*s3 - 270*s2*s3)) + c5*(270*c2 + 90))) + (7775400025877285*c3*c4)/2361183241434822606848 + (1883354923850515*c3*s4)/1152921504606846976 - (5813615622121687*s3*s4)/288230376151711744 + (943793072886211*c5*(c3*s4 - c4*s3))/2305843009213693952 + 90*m6*(s4*(295*c3 - 270*c3*s2) - c4*(295*s3 - 270*s2*s3)) + 90*m5*(270*c2 + 90) - 295*m6*((7775400025877285*s3*s4)/2361183241434822606848 - c5*(c4*(295*c3 - 270*c3*s2) + s4*(295*s3 - 270*s2*s3)) + (8198078942807907*s5*(c3*s4 - c4*s3))/2305843009213693952 + s5*(270*c2 + 90) - 295*m7*s5*(c6*(s5*(c4*(295*c3 - 270*c3*s2) + s4*(295*s3 - 270*s2*s3)) - 80*c5*(c3*s4 - c4*s3) + c5*(270*c2 + 90)) - s6*(c5*(c4*(295*c3 - 270*c3*s2) + s4*(295*s3 - 270*s2*s3)) + 80*s5*(c3*s4 - c4*s3) - s5*(270*c2 + 90)) + 80*s5*s6*(c3*s4 - c4*s3) + 80*c5*c6*(c3*s4 - c4*s3))) + 90*m7*s5*(s6*(s5*(c4*(295*c3 - 270*c3*s2) + s4*(295*s3 - 270*s2*s3)) - 80*c5*(c3*s4 - c4*s3) + c5*(270*c2 + 90)) + c6*(c5*(c4*(295*c3 - 270*c3*s2) + s4*(295*s3 - 270*s2*s3)) + 80*s5*(c3*s4 - c4*s3) - s5*(270*c2 + 90)) + 80*c5*s6*(c3*s4 - c4*s3) - 80*c6*s5*(c3*s4 - c4*s3)) + 295*c5*m7*(s6*(s5*(c4*(295*c3 - 270*c3*s2) + s4*(295*s3 - 270*s2*s3)) - 80*c5*(c3*s4 - c4*s3) + c5*(270*c2 + 90)) + c6*(c5*(c4*(295*c3 - 270*c3*s2) + s4*(295*s3 - 270*s2*s3)) + 80*s5*(c3*s4 - c4*s3) - s5*(270*c2 + 90)) + 80*c5*s6*(c3*s4 - c4*s3) - 80*c6*s5*(c3*s4 - c4*s3)) + 90*c5*m7*(c6*(s5*(c4*(295*c3 - 270*c3*s2) + s4*(295*s3 - 270*s2*s3)) - 80*c5*(c3*s4 - c4*s3) + c5*(270*c2 + 90)) - s6*(c5*(c4*(295*c3 - 270*c3*s2) + s4*(295*s3 - 270*s2*s3)) + 80*s5*(c3*s4 - c4*s3) - s5*(270*c2 + 90)) + 80*s5*s6*(c3*s4 - c4*s3) + 80*c5*c6*(c3*s4 - c4*s3))) + 270*m5*(270*c2 + 90) + 270*m7*s5*(s6*(s5*(c4*(295*c3 - 270*c3*s2) + s4*(295*s3 - 270*s2*s3)) - 80*c5*(c3*s4 - c4*s3) + c5*(270*c2 + 90)) + c6*(c5*(c4*(295*c3 - 270*c3*s2) + s4*(295*s3 - 270*s2*s3)) + 80*s5*(c3*s4 - c4*s3) - s5*(270*c2 + 90)) + 80*c5*s6*(c3*s4 - c4*s3) - 80*c6*s5*(c3*s4 - c4*s3)) + 72900*m4*s2*s3 + 270*c5*m7*(c6*(s5*(c4*(295*c3 - 270*c3*s2) + s4*(295*s3 - 270*s2*s3)) - 80*c5*(c3*s4 - c4*s3) + c5*(270*c2 + 90)) - s6*(c5*(c4*(295*c3 - 270*c3*s2) + s4*(295*s3 - 270*s2*s3)) + 80*s5*(c3*s4 - c4*s3) - s5*(270*c2 + 90)) + 80*s5*s6*(c3*s4 - c4*s3) + 80*c5*c6*(c3*s4 - c4*s3))));
 
m22 = -((8581632868960513*c3)/1152921504606846976 + c3*(24300*m5 + (7145951600741313*s3)/288230376151711744 + (5813615622121687*c3*c4)/288230376151711744 + (1883354923850515*c4*s3)/1152921504606846976 + 270*m6*(295*c3*s4 - 295*c4*s3) + c4*(8100*m5 + s4*(c5*((1831324867619693*s5*s6*(c3*s4 - c4*s3))/295147905179352825856 + (1831324867619693*c5*c6*(c3*s4 - c4*s3))/295147905179352825856) + s5*((7115472921728667*c5*s6*(c3*s4 - c4*s3))/2361183241434822606848 - (7115472921728667*c6*s5*(c3*s4 - c4*s3))/2361183241434822606848) - 295*m6*(90*c5 + s5*(295*c3*c4 + 295*s3*s4)) + (3495819410978605*c5*(c3*s4 - c4*s3))/2305843009213693952 + 295*m7*(295*c3*s4 - 295*c4*s3) + (943793072886211*s5*(c3*s4 - c4*s3))/2305843009213693952) + (7775400025877285*c3*c4)/2361183241434822606848 + (1883354923850515*c3*s4)/1152921504606846976 - (5813615622121687*s3*s4)/288230376151711744 + (943793072886211*c5*(c3*s4 - c4*s3))/2305843009213693952 + 90*m6*(295*c3*s4 - 295*c4*s3) - 295*m6*(90*s5 + (7775400025877285*s3*s4)/2361183241434822606848 - c5*(295*c3*c4 + 295*s3*s4) + (8198078942807907*s5*(c3*s4 - c4*s3))/2305843009213693952 - 295*m7*s5*(c6*(90*c5 - 80*c5*(c3*s4 - c4*s3) + s5*(295*c3*c4 + 295*s3*s4)) - s6*(c5*(295*c3*c4 + 295*s3*s4) - 90*s5 + 80*s5*(c3*s4 - c4*s3)) + 80*s5*s6*(c3*s4 - c4*s3) + 80*c5*c6*(c3*s4 - c4*s3))) + 295*c5*m7*(c6*(c5*(295*c3*c4 + 295*s3*s4) - 90*s5 + 80*s5*(c3*s4 - c4*s3)) + s6*(90*c5 - 80*c5*(c3*s4 - c4*s3) + s5*(295*c3*c4 + 295*s3*s4)) + 80*c5*s6*(c3*s4 - c4*s3) - 80*c6*s5*(c3*s4 - c4*s3)) + 90*c5*m7*(c6*(90*c5 - 80*c5*(c3*s4 - c4*s3) + s5*(295*c3*c4 + 295*s3*s4)) - s6*(c5*(295*c3*c4 + 295*s3*s4) - 90*s5 + 80*s5*(c3*s4 - c4*s3)) + 80*s5*s6*(c3*s4 - c4*s3) + 80*c5*c6*(c3*s4 - c4*s3)) + 90*m7*s5*(c6*(c5*(295*c3*c4 + 295*s3*s4) - 90*s5 + 80*s5*(c3*s4 - c4*s3)) + s6*(90*c5 - 80*c5*(c3*s4 - c4*s3) + s5*(295*c3*c4 + 295*s3*s4)) + 80*c5*s6*(c3*s4 - c4*s3) - 80*c6*s5*(c3*s4 - c4*s3))) - s3*((1883354923850515*c3*c4)/1152921504606846976 - (1369254254579395*c3*s4)/144115188075855872 + (1369254254579395*c4*s3)/144115188075855872 + (1883354923850515*s3*s4)/1152921504606846976 - s4*((7775400025877285*c3*c4)/2361183241434822606848 + 295*c5*m7*(c6*(c5*(295*c3*c4 + 295*s3*s4) - 90*s5 + 80*s5*(c3*s4 - c4*s3)) + s6*(90*c5 - 80*c5*(c3*s4 - c4*s3) + s5*(295*c3*c4 + 295*s3*s4)) - (7775400025877285*s3*s4)/2361183241434822606848 + 295*m6*(90*s5 - c5*(295*c3*c4 + 295*s3*s4)) - (943793072886211*c5*(c3*s4 - c4*s3))/2305843009213693952 - (8198078942807907*s5*(c3*s4 - c4*s3))/2305843009213693952 + 295*m7*s5*(c6*(90*c5 - 80*c5*(c3*s4 - c4*s3) + s5*(295*c3*c4 + 295*s3*s4)) - s6*(c5*(295*c3*c4 + 295*s3*s4) - 90*s5 + 80*s5*(c3*s4 - c4*s3)) + 80*s5*s6*(c3*s4 - c4*s3) + 80*c5*c6*(c3*s4 - c4*s3)) + 80*c5*s6*(c3*s4 - c4*s3) - 80*c6*s5*(c3*s4 - c4*s3))) - c4*(c5*((1831324867619693*s5*s6*(c3*s4 - c4*s3))/295147905179352825856 + (1831324867619693*c5*c6*(c3*s4 - c4*s3))/295147905179352825856) + s5*((7115472921728667*c5*s6*(c3*s4 - c4*s3))/2361183241434822606848 - (7115472921728667*c6*s5*(c3*s4 - c4*s3))/2361183241434822606848) - 295*m6*(90*c5 + s5*(295*c3*c4 + 295*s3*s4)) + (3495819410978605*c5*(c3*s4 - c4*s3))/2305843009213693952 + 295*m7*(295*c3*s4 - 295*c4*s3) + (943793072886211*s5*(c3*s4 - c4*s3))/2305843009213693952)) + 270*c5*m7*(c6*(90*c5 - 80*c5*(c3*s4 - c4*s3) + s5*(295*c3*c4 + 295*s3*s4)) - s6*(c5*(295*c3*c4 + 295*s3*s4) - 90*s5 + 80*s5*(c3*s4 - c4*s3)) + 80*s5*s6*(c3*s4 - c4*s3) + 80*c5*c6*(c3*s4 - c4*s3)) + 270*m7*s5*(c6*(c5*(295*c3*c4 + 295*s3*s4) - 90*s5 + 80*s5*(c3*s4 - c4*s3)) + s6*(90*c5 - 80*c5*(c3*s4 - c4*s3) + s5*(295*c3*c4 + 295*s3*s4)) + 80*c5*s6*(c3*s4 - c4*s3) - 80*c6*s5*(c3*s4 - c4*s3))));
 
m23 = c3*(24300*m4 + s3*(295*c5*m7*s4*((8198078942807907*c5)/2305843009213693952 - (943793072886211*s5)/2305843009213693952) - c4*((943793072886211*c5)/2305843009213693952 - (3495819410978605*s5)/2305843009213693952 + c5*((1831324867619693*c5*s6)/295147905179352825856 - (1831324867619693*c6*s5)/295147905179352825856) - s5*((7115472921728667*c5*c6)/2361183241434822606848 + (7115472921728667*s5*s6)/2361183241434822606848)) + 4965898922391233/590295810358705651712) - c4*((8198078942807907*c5)/2305843009213693952 + s4*((943793072886211*c5)/2305843009213693952 - (3495819410978605*s5)/2305843009213693952 + c5*((1831324867619693*c5*s6)/295147905179352825856 - (1831324867619693*c6*s5)/295147905179352825856) - s5*((7115472921728667*c5*c6)/2361183241434822606848 + (7115472921728667*s5*s6)/2361183241434822606848)) + (278418956501432245*m6*s5)/2305843009213693952 + 397124457897871/147573952589676412928) + 7478065051662123/36028797018963968);
 
m24 = -c3*(s3*(295*c5*m7*s4*((8198078942807907*c5)/2305843009213693952 - (943793072886211*s5)/2305843009213693952) - c4*((943793072886211*c5)/2305843009213693952 - (3495819410978605*s5)/2305843009213693952 + c5*((1831324867619693*c5*s6)/295147905179352825856 - (1831324867619693*c6*s5)/295147905179352825856) - s5*((7115472921728667*c5*c6)/2361183241434822606848 + (7115472921728667*s5*s6)/2361183241434822606848)) + 4965898922391233/590295810358705651712) - c4*((8198078942807907*c5)/2305843009213693952 + s4*((943793072886211*c5)/2305843009213693952 - (3495819410978605*s5)/2305843009213693952 + c5*((1831324867619693*c5*s6)/295147905179352825856 - (1831324867619693*c6*s5)/295147905179352825856) - s5*((7115472921728667*c5*c6)/2361183241434822606848 + (7115472921728667*s5*s6)/2361183241434822606848)) + (278418956501432245*m6*s5)/2305843009213693952 + 397124457897871/147573952589676412928));
 
m25 = -c3*((2293743007633799075*c4*m6)/2361183241434822606848 + (2293743007633799075*c5*m7*s3*s4)/2361183241434822606848);

m26 = c3*((2293743007633799075*c4*m6)/2361183241434822606848 + (2293743007633799075*c5*m7*s3*s4)/2361183241434822606848);
 

m31 = ((1035355510473309*c3*c4)/288230376151711744 + (4965898922391233*c3*s4)/590295810358705651712 - (4965898922391233*c4*s3)/590295810358705651712 + (1035355510473309*s3*s4)/288230376151711744 - s5*((1831324867619693*s5*s6*(c3*s4 - c4*s3))/295147905179352825856 + (1831324867619693*c5*c6*(c3*s4 - c4*s3))/295147905179352825856) + 90*c4*(m7*(s4*(295*c3 - 270*c3*s2) - c4*(295*s3 - 270*s2*s3)) - m6*(s5*(c4*(295*c3 - 270*c3*s2) + s4*(295*s3 - 270*s2*s3)) + c5*(270*c2 + 90))) + c5*((7115472921728667*c5*s6*(c3*s4 - c4*s3))/2361183241434822606848 - (7115472921728667*c6*s5*(c3*s4 - c4*s3))/2361183241434822606848) + 90*s4*(m6*(c5*(c4*(295*c3 - 270*c3*s2) + s4*(295*s3 - 270*s2*s3)) - s5*(270*c2 + 90)) - m7*s5*(c6*(s5*(c4*(295*c3 - 270*c3*s2) + s4*(295*s3 - 270*s2*s3)) - 80*c5*(c3*s4 - c4*s3) + c5*(270*c2 + 90)) - s6*(c5*(c4*(295*c3 - 270*c3*s2) + s4*(295*s3 - 270*s2*s3)) + 80*s5*(c3*s4 - c4*s3) - s5*(270*c2 + 90)) + 80*s5*s6*(c3*s4 - c4*s3) + 80*c5*c6*(c3*s4 - c4*s3)) + c5*m7*(s6*(s5*(c4*(295*c3 - 270*c3*s2) + s4*(295*s3 - 270*s2*s3)) - 80*c5*(c3*s4 - c4*s3) + c5*(270*c2 + 90)) + c6*(c5*(c4*(295*c3 - 270*c3*s2) + s4*(295*s3 - 270*s2*s3)) + 80*s5*(c3*s4 - c4*s3) - s5*(270*c2 + 90)) + 80*c5*s6*(c3*s4 - c4*s3) - 80*c6*s5*(c3*s4 - c4*s3))) + 90*m5*(s4*(295*c3 - 270*c3*s2) - 295*c3*s4 + 295*c4*s3 - c4*(295*s3 - 270*s2*s3)));
 
m32 = ((1035355510473309*c3*c4)/288230376151711744 + (4965898922391233*c3*s4)/590295810358705651712 - (4965898922391233*c4*s3)/590295810358705651712 - 90*c4*(m6*(90*c5 + s5*(295*c3*c4 + 295*s3*s4)) - m7*(295*c3*s4 - 295*c4*s3)) + (1035355510473309*s3*s4)/288230376151711744 - s5*((1831324867619693*s5*s6*(c3*s4 - c4*s3))/295147905179352825856 + (1831324867619693*c5*c6*(c3*s4 - c4*s3))/295147905179352825856) - 90*s4*(m6*(90*s5 - c5*(295*c3*c4 + 295*s3*s4)) - c5*m7*(c6*(c5*(295*c3*c4 + 295*s3*s4) - 90*s5 + 80*s5*(c3*s4 - c4*s3)) + s6*(90*c5 - 80*c5*(c3*s4 - c4*s3) + s5*(295*c3*c4 + 295*s3*s4)) + 80*c5*s6*(c3*s4 - c4*s3) - 80*c6*s5*(c3*s4 - c4*s3)) + m7*s5*(c6*(90*c5 - 80*c5*(c3*s4 - c4*s3) + s5*(295*c3*c4 + 295*s3*s4)) - s6*(c5*(295*c3*c4 + 295*s3*s4) - 90*s5 + 80*s5*(c3*s4 - c4*s3)) + 80*s5*s6*(c3*s4 - c4*s3) + 80*c5*c6*(c3*s4 - c4*s3))) + c5*((7115472921728667*c5*s6*(c3*s4 - c4*s3))/2361183241434822606848 - (7115472921728667*c6*s5*(c3*s4 - c4*s3))/2361183241434822606848));
 
m33 = -(s5*((1831324867619693*c5*s6)/295147905179352825856 - (1831324867619693*c6*s5)/295147905179352825856) + c5*((7115472921728667*c5*c6)/2361183241434822606848 + (7115472921728667*s5*s6)/2361183241434822606848) + 869375736758729/36028797018963968);
 
m34 = (s5*((1831324867619693*c5*s6)/295147905179352825856 - (1831324867619693*c6*s5)/295147905179352825856) + c5*((7115472921728667*c5*c6)/2361183241434822606848 + (7115472921728667*s5*s6)/2361183241434822606848) + 869375736758729/36028797018963968);

m35 = -(8276639014131817)/2305843009213693952;
 
m36 = 0;


m41 = -((8276639014131817*c3*c4)/2305843009213693952 + (8276639014131817*s3*s4)/2305843009213693952 - s5*((1831324867619693*s5*s6*(c3*s4 - c4*s3))/295147905179352825856 + (1831324867619693*c5*c6*(c3*s4 - c4*s3))/295147905179352825856) + c5*((7115472921728667*c5*s6*(c3*s4 - c4*s3))/2361183241434822606848 - (7115472921728667*c6*s5*(c3*s4 - c4*s3))/2361183241434822606848));

m42 = -((8276639014131817*c3*c4)/2305843009213693952 + (8276639014131817*s3*s4)/2305843009213693952 - s5*((1831324867619693*s5*s6*(c3*s4 - c4*s3))/295147905179352825856 + (1831324867619693*c5*c6*(c3*s4 - c4*s3))/295147905179352825856) + c5*((7115472921728667*c5*s6*(c3*s4 - c4*s3))/2361183241434822606848 - (7115472921728667*c6*s5*(c3*s4 - c4*s3))/2361183241434822606848));
 
m43 = (s5*((1831324867619693*c5*s6)/295147905179352825856 - (1831324867619693*c6*s5)/295147905179352825856) + c5*((7115472921728667*c5*c6)/2361183241434822606848 + (7115472921728667*s5*s6)/2361183241434822606848));
 
m44 = -(s5*((1831324867619693*c5*s6)/295147905179352825856 - (1831324867619693*c6*s5)/295147905179352825856) + c5*((7115472921728667*c5*c6)/2361183241434822606848 + (7115472921728667*s5*s6)/2361183241434822606848));
 
m45 = (8276639014131817)/2305843009213693952;
 
m46 = 0;


m51 = ((7775400025877285*c3*c4)/2361183241434822606848 + (7775400025877285*s3*s4)/2361183241434822606848);

m52 = ((7775400025877285*c3*c4)/2361183241434822606848 + (7775400025877285*s3*s4)/2361183241434822606848);

m53 = 0;

m54 = 0;

m55 = -(7775400025877285)/2361183241434822606848;

m56 = (7775400025877285)/2361183241434822606848;
 


m61 = 0;
m62 = 0;
m63 = 0;
m64 = 0;
m65 = 0;
m66 = 0;

M = [m11 m12 m13 m14 m15 m16; ...
    m21 m22 m23 m24 m25 m26; ...
    m31 m32 m33 m34 m35 m36; ...
    m41 m42 m43 m44 m45 m56; ...
    m51 m52 m53 m54 m55 m56;...
    m61 m62 m63 m64 m65 m66]




%% matrix v

v11 = -335*c2*(c3*(c4*(c5*m7*(80*c6*(- qd(5)*(c5*(-c3*s4*(qd(1) + qd(2)) + c4*s3*(qd(1) + qd(2))) - s5*(-qd(3) + qd(4))) - s5*(c4*(c3*qd(3)*(qd(1) + qd(2))) + qd(4)*(-c3*c4*(qd(1) + qd(2)) - s3*s4*(qd(1) + qd(2))) - qd(3)*s3*(qd(1) + qd(2))))) + c6*(80*c5*(c5*(c4*(c3*(c2*(- 270*qd(1)^2) - (qd(1) + qd(2))*(90*qd(1) + 90*qd(2)))) - s3*(c2*(- 270*qd(1)^2) - (qd(1) + qd(2))*(90*qd(1) + 90*qd(2))))) + 80*qd(5)*(c5*(-c3*s4*(qd(1) + qd(2)) + c4*s3*(qd(1) + qd(2))) - s5*(-qd(3) + qd(4))) + 80*s5*(c4*(c3*qd(3)*(qd(1) + qd(2))) + qd(4)*(-c3*c4*(qd(1) + qd(2)) - s3*s4*(qd(1) + qd(2))) - s4*(- qd(3)*s3*(qd(1) + qd(2)))) - s5*(- 295*c3^2*(qd(1) + qd(2))^2 + s2*(- 270*qd(1)^2) - 295*s3^2*(qd(1) + qd(2))^2) - (80*c5*(-c3*s4*(qd(1) + qd(2)) + c4*s3*(qd(1) + qd(2))) - 80*s5*(-qd(3) + qd(4)))*(-c3*c4*(qd(1) + qd(2)) + qd(5) - s3*s4*(qd(1) + qd(2)))) + 80*qd(6)*(c6*(c5*(-c3*s4*(qd(1) + qd(2)) + c4*s3*(qd(1) + qd(2))) - s5*(-qd(3) + qd(4))) - s6*(-c5*(-qd(3) + qd(4)) - s5*(-c3*s4*(qd(1) + qd(2)) + c4*s3*(qd(1) + qd(2))))) + 80*s6*(c5*(c4*(c3*qd(3)*(qd(1) + qd(2))) + qd(4)*(-c3*c4*(qd(1) + qd(2)) - s3*s4*(qd(1) + qd(2))) - s4*(- qd(3)*s3*(qd(1) + qd(2)))) + qd(5)*(-c5*(-qd(3) + qd(4)) - s5*(-c3*s4*(qd(1) + qd(2)) + c4*s3*(qd(1) + qd(2))))) - s6*(80*c5*(c4*(c3*qd(3)*(qd(1) + qd(2))) + qd(4)*(-c3*c4*(qd(1) + qd(2)) - s3*s4*(qd(1) + qd(2))) - s4*(- qd(3)*s3*(qd(1) + qd(2)))) - c5*(- 295*c3^2*(qd(1) + qd(2))^2 + s2*(- 270*qd(1)^2) - 295*s3^2*(qd(1) + qd(2))^2) + 80*qd(5)*(-c5*(-qd(3) + qd(4)) - s5*(-c3*s4*(qd(1) + qd(2)) + c4*s3*(qd(1) + qd(2)))) - s5*(c4*(c3*(c2*(- 270*qd(1)^2) - (qd(1) + qd(2))*(90*qd(1) + 90*qd(2)))) - s3*(c2*(- 270*qd(1)^2) - (qd(1) + qd(2))*(90*qd(1) + 90*qd(2))))) + (80*c5*(-qd(3) + qd(4)) + 80*s5*(-c3*s4*(qd(1) + qd(2)) + c4*s3*(qd(1) + qd(2))))*(-c3*c4*(qd(1) + qd(2)) + qd(5) - s3*s4*(qd(1) + qd(2)))) - (80*c6*(c5*(-c3*s4*(qd(1) + qd(2)) + c4*s3*(qd(1) + qd(2))) - s5*(-qd(3) + qd(4))) - 80*s6*(-c5*(-qd(3) + qd(4)) - s5*(-c3*s4*(qd(1) + qd(2)) + c4*s3*(qd(1) + qd(2)))))*(c3*c4*(qd(1) + qd(2)) - qd(5) + qd(6) + s3*s4*(qd(1) + qd(2)))) + m6*(c5*(c4*(c3*(c2*(- 270*qd(1)^2) - (qd(1) + qd(2))*(90*qd(1) + 90*qd(2)))) - s3*(c2*(- 270*qd(1)^2) - (qd(1) + qd(2))*(90*qd(1) + 90*qd(2))))) - s5*(- 295*c3^2*(qd(1) + qd(2))^2 + s2*(- 270*qd(1)^2) - 295*s3^2*(qd(1) + qd(2))^2)) - m7*s5*(80*c6*(c5*(c4*(c3*qd(3)*(qd(1) + qd(2))) + qd(4)*(-c3*c4*(qd(1) + qd(2)) - s3*s4*(qd(1) + qd(2))) - qd(3)*s3*(qd(1) + qd(2)))) + qd(5)*(-c5*(-qd(3) + qd(4)) - s5*(-c3*s4*(qd(1) + qd(2)) + c4*s3*(qd(1) + qd(2))))) - c6*(80*c5*(c4*(c3*qd(3)*(qd(1) + qd(2))) + qd(4)*(-c3*c4*(qd(1) + qd(2)) - s3*s4*(qd(1) + qd(2))) - s4*(- qd(3)*s3*(qd(1) + qd(2)))) - c5*(- 295*(c3^2)*(qd(1) + qd(2))^2 + s2*(- 270*qd(1)^2) - 295*(s3^2)*(qd(1) + qd(2))^2) + 80*qd(5)*(-c5*(-qd(3) + qd(4)) - s5*(-c3*s4*(qd(1) + qd(2)) + c4*s3*(qd(1) + qd(2)))) - s5*(c4*(c3*(c2*(- 270*(qd(1)^2)) - (qd(1) + qd(2))*(90*qd(1) + 90*qd(2)))) - s4*(- s3*(c2*(- 270*(qd(1)^2)) - (qd(1) + qd(2))*(90*qd(1) + 90*qd(2))))) + (80*c5*(-qd(3) + qd(4)) + 80*s5*(-c3*s4*(qd(1) + qd(2)) + c4*s3*(qd(1) + qd(2))))*(-c3*c4*(qd(1) + qd(2)) + qd(5) - s3*s4*(qd(1) + qd(2)))) + 80*qd(6)*(-c6*(-c5*(-qd(3) + qd(4)) - s5*(-c3*s4*(qd(1) + qd(2)) + c4*s3*(qd(1) + qd(2)))) - s6*(c5*(-c3*s4*(qd(1) + qd(2)) + c4*s3*(qd(1) + qd(2))) - s5*(-qd(3) + qd(4)))) - 80*s6*(- qd(5)*(c5*(-c3*s4*(qd(1) + qd(2)) + c4*s3*(qd(1) + qd(2))) - s5*(-qd(3) + qd(4))) - s5*(c4*(c3*qd(3)*(qd(1) + qd(2))) + qd(4)*(-c3*c4*(qd(1) + qd(2)) - s3*s4*(qd(1) + qd(2))) - s4*(- qd(3)*s3*(qd(1) + qd(2))))) - s6*(c5*(c4*(c3*(c2*(- 270*(qd(1)^2)) - (qd(1) + qd(2))*(90*qd(1) + 90*qd(2)))) - s4*(- s3*(c2*(- 270*(qd(1)^2)) - (qd(1) + qd(2))*(90*qd(1) + 90*qd(2))))) + 80*qd(5)*(c5*(-c3*s4*(qd(1) + qd(2)) + c4*s3*(qd(1) + qd(2))) - s5*(-qd(3) + qd(4))) + 80*s5*(c4*(c3*qd(3)*(qd(1) + qd(2))) + qd(4)*(-c3*c4*(qd(1) + qd(2)) - s3*s4*(qd(1) + qd(2))) - s4*(- qd(3)*s3*(qd(1) + qd(2)))) - s5*( - 295*(c3^2)*(qd(1) + qd(2))^2 + s2*(- 270*(qd(1)^2)) - 295*(s3^2)*(qd(1) + qd(2))^2) - (80*c5*(-c3*s4*(qd(1) + qd(2)) + c4*s3*(qd(1) + qd(2))) - 80*s5*(-qd(3) + qd(4)))*(-c3*c4*(qd(1) + qd(2)) + qd(5) - s3*s4*(qd(1) + qd(2)))) + (80*c6*(-c5*(-qd(3) + qd(4)) - s5*(-c3*s4*(qd(1) + qd(2)) + c4*s3*(qd(1) + qd(2)))) + 80*s6*(c5*(-c3*s4*(qd(1) + qd(2)) + c4*s3*(qd(1) + qd(2))) - s5*(-qd(3) + qd(4))))*(c3*c4*(qd(1) + qd(2)) - qd(5) + qd(6) + s3*s4*(qd(1) + qd(2))) + m5*(c4*(c3*(c2*(- 270*(qd(1)^2)) - (qd(1) + qd(2))*(90*qd(1) + 90*qd(2)))) + 295*c4*(- qd(3)*s3*(qd(1) + qd(2))) + 295*qd(4)*(-c3*s4*(qd(1) + qd(2)) + c4*s3*(qd(1) + qd(2))) - s4*(- s3*(c2*(- 270*(qd(1)^2)) - (qd(1) + qd(2))*(90*qd(1) + 90*qd(2)))) + 295*s4*(c3*qd(3)*(qd(1) + qd(2))) - (-qd(3) + qd(4))*(-295*c3*s4*(qd(1) + qd(2)) + 295*c4*s3*(qd(1) + qd(2)))) - s4*(m6*(-c5*(- 295*(c3^2)*(qd(1) + qd(2))^2 + s2*(- 270*(qd(1)^2)) - 295*(s3^2)*(qd(1) + qd(2))^2) - s5*(c4*(c3*(c2*(- 270*(qd(1)^2))  - (qd(1) + qd(2))*(90*qd(1) + 90*qd(2)))) - s4*(- s3*(c2*(- 270*(qd(1)^2)) - (qd(1) + qd(2))*(90*qd(1) + 90*qd(2)))))) + m7*(c4*(- s3*(c2*(- 270*qd(1)^2) - (qd(1) + qd(2))*(90*qd(1) + 90*qd(2)))) + s4*(c3*(c2*( - 270*qd(1)^2) - (qd(1) + qd(2))*(90*qd(1) + 90*qd(2)))) + (-c5*(-qd(3) + qd(4)) - s5*(-c3*s4*(qd(1) + qd(2)) + c4*s3*(qd(1) + qd(2))))*(80*c5*(-qd(3) + qd(4)) + 80*s5*(-c3*s4*(qd(1) + qd(2)) + c4*s3*(qd(1) + qd(2)))) - (c5*(-c3*s4*(qd(1) + qd(2)) + c4*s3*(qd(1) + qd(2))) - s5*(-qd(3) + qd(4)))*(80*c5*(-c3*s4*(qd(1) + qd(2)) + c4*s3*(qd(1) + qd(2))) - 80*s5*(-qd(3) + qd(4))) - (-c6*(-c5*(-qd(3) + qd(4)) - s5*(-c3*s4*(qd(1) + qd(2)) + c4*s3*(qd(1) + qd(2)))) - s6*(c5*(-c3*s4*(qd(1) + qd(2)) + c4*s3*(qd(1) + qd(2))) - s5*(-qd(3) + qd(4))))*(80*c6*(-c5*(-qd(3) + qd(4)) - s5*(-c3*s4*(qd(1) + qd(2)) + c4*s3*(qd(1) + qd(2)))) + 80*s6*(c5*(-c3*s4*(qd(1) + qd(2)) + c4*s3*(qd(1) + qd(2))) - s5*(-qd(3) + qd(4)))) + (c6*(c5*(-c3*s4*(qd(1) + qd(2)) + c4*s3*(qd(1) + qd(2))) - s5*(-qd(3) + qd(4))) - s6*(-c5*(-qd(3) + qd(4)) - s5*(-c3*s4*(qd(1) + qd(2)) + c4*s3*(qd(1) + qd(2)))))*(80*c6*(c5*(-c3*s4*(qd(1) + qd(2)) + c4*s3*(qd(1) + qd(2))) - s5*(-qd(3) + qd(4))) - 80*s6*(-c5*(-qd(3) + qd(4)) - s5*(-c3*s4*(qd(1) + qd(2)) + c4*s3*(qd(1) + qd(2))))))) + m4*(-90*c3^2*(qd(1) + qd(2))^2 + c3*(c2*(- 270*qd(1)^2)  - (qd(1) + qd(2))*(90*qd(1) + 90*qd(2))) - 90*qd(3)^2) - s3*(-c4*(m6*(-c5*( - 295*c3^2*(qd(1) + qd(2))^2 + s2*(- 270*qd(1)^2) - 295*s3^2*(qd(1) + qd(2))^2) - s5*(c4*(c3*(c2*(- 270*qd(1)^2) - (qd(1) + qd(2))*(90*qd(1) + 90*qd(2)))) - s4*(- s3*(c2*(- 270*qd(1)^2) - (qd(1) + qd(2))*(90*qd(1) + 90*qd(2)))))) + m7*(c4*(- s3*(c2*(- 270*qd(1)^2) - (qd(1) + qd(2))*(90*qd(1) + 90*qd(2)))) + s4*(c3*(c2*(- 270*qd(1)^2) - (qd(1) + qd(2))*(90*qd(1) + 90*qd(2)))) + (-c5*(-qd(3) + qd(4)) - s5*(-c3*s4*(qd(1) + qd(2)) + c4*s3*(qd(1) + qd(2))))*(80*c5*(-qd(3) + qd(4)) + 80*s5*(-c3*s4*(qd(1) + qd(2)) + c4*s3*(qd(1) + qd(2)))) - (c5*(-c3*s4*(qd(1) + qd(2)) + c4*s3*(qd(1) + qd(2))) - s5*(-qd(3) + qd(4)))*(80*c5*(-c3*s4*(qd(1) + qd(2)) + c4*s3*(qd(1) + qd(2))) - 80*s5*(-qd(3) + qd(4))) - (-c6*(-c5*(-qd(3) + qd(4)) - s5*(-c3*s4*(qd(1) + qd(2)) + c4*s3*(qd(1) + qd(2)))) - s6*(c5*(-c3*s4*(qd(1) + qd(2)) + c4*s3*(qd(1) + qd(2))) - s5*(-qd(3) + qd(4))))*(80*c6*(-c5*(-qd(3) + qd(4)) - s5*(-c3*s4*(qd(1) + qd(2)) + c4*s3*(qd(1) + qd(2)))) + 80*s6*(c5*(-c3*s4*(qd(1) + qd(2)) + c4*s3*(qd(1) + qd(2))) - s5*(-qd(3) + qd(4)))) + (c6*(c5*(-c3*s4*(qd(1) + qd(2)) + c4*s3*(qd(1) + qd(2))) - s5*(-qd(3) + qd(4))) - s6*(-c5*(-qd(3) + qd(4)) - s5*(-c3*s4*(qd(1) + qd(2)) + c4*s3*(qd(1) + qd(2)))))*(80*c6*(c5*(-c3*s4*(qd(1) + qd(2)) + c4*s3*(qd(1) + qd(2))) - s5*(-qd(3) + qd(4))) - 80*s6*(-c5*(-qd(3) + qd(4)) - s5*(-c3*s4*(qd(1) + qd(2)) + c4*s3*(qd(1) + qd(2))))))) + m5*(-c4*(- s3*(c2*(- 270*qd(1)^2) - (qd(1) + qd(2))*(90*qd(1) + 90*qd(2)))) + 295*c4*(c3*qd(3)*(qd(1) + qd(2))) + 295*qd(4)*(-c3*c4*(qd(1) + qd(2)) - s3*s4*(qd(1) + qd(2))) - s4*(+ c3*(c2*(- 270*qd(1)^2) - (qd(1) + qd(2))*(90*qd(1) + 90*qd(2)))) - 295*s4*(- qd(3)*s3*(qd(1) + qd(2))) + (-qd(3) + qd(4))*(295*c3*c4*(qd(1) + qd(2)) + 295*s3*s4*(qd(1) + qd(2)))) - s4*(c5*m7*(80*c6*(- qd(5)*(c5*(-c3*s4*(qd(1) + qd(2)) + c4*s3*(qd(1) + qd(2))) - s5*(-qd(3) + qd(4))) - s5*(c4*(c3*qd(3)*(qd(1) + qd(2))) + qd(4)*(-c3*c4*(qd(1) + qd(2)) - s3*s4*(qd(1) + qd(2))) - s4*( - qd(3)*s3*(qd(1) + qd(2))))) + c6*(c5*(c4*(c3*(c2*(- 270*qd(1)^2) - (qd(1) + qd(2))*(90*qd(1) + 90*qd(2)))) - s4*(- s3*(c2*(- 270*qd(1)^2) - (qd(1) + qd(2))*(90*qd(1) + 90*qd(2))))) + 80*qd(5)*(c5*(-c3*s4*(qd(1) + qd(2)) + c4*s3*(qd(1) + qd(2))) - s5*(-qd(3) + qd(4))) + 80*s5*(c4*(c3*qd(3)*(qd(1) + qd(2))) + qd(4)*(-c3*c4*(qd(1) + qd(2)) - s3*s4*(qd(1) + qd(2))) - s4*(- qd(3)*s3*(qd(1) + qd(2)))) - s5*(- 295*c3^2*(qd(1) + qd(2))^2 + s2*(- 270*qd(1)^2) - 295*s3^2*(qd(1) + qd(2))^2) - (80*c5*(-c3*s4*(qd(1) + qd(2)) + c4*s3*(qd(1) + qd(2))) - 80*s5*(-qd(3) + qd(4)))*(-c3*c4*(qd(1) + qd(2)) + qd(5) - s3*s4*(qd(1) + qd(2)))) + 80*qd(6)*(c6*(c5*(-c3*s4*(qd(1) + qd(2)) + c4*s3*(qd(1) + qd(2))) - s5*(-qd(3) + qd(4))) - s6*(-c5*(-qd(3) + qd(4)) - s5*(-c3*s4*(qd(1) + qd(2)) + c4*s3*(qd(1) + qd(2))))) + 80*s6*(c5*(c4*(c3*qd(3)*(qd(1) + qd(2))) + qd(4)*(-c3*c4*(qd(1) + qd(2)) - s3*s4*(qd(1) + qd(2))) - s4*(- qd(3)*s3*(qd(1) + qd(2)))) + qd(5)*(-c5*(-qd(3) + qd(4)) - s5*(-c3*s4*(qd(1) + qd(2)) + c4*s3*(qd(1) + qd(2))))) - s6*(80*c5*(c4*(c3*qd(3)*(qd(1) + qd(2))) + qd(4)*(-c3*c4*(qd(1) + qd(2)) - s3*s4*(qd(1) + qd(2))) - s4*(- qd(3)*s3*(qd(1) + qd(2)))) - c5*( - 295*c3^2*(qd(1) + qd(2))^2 + s2*(- 270*qd(1)^2) - 295*s3^2*(qd(1) + qd(2))^2) + 80*qd(5)*(-c5*(-qd(3) + qd(4)) - s5*(-c3*s4*(qd(1) + qd(2)) + c4*s3*(qd(1) + qd(2)))) - s5*(c4*(c3*(c2*( - 270*qd(1)^2) - (qd(1) + qd(2))*(90*qd(1) + 90*qd(2)))) - s4*(- s3*(c2*(- 270*qd(1)^2) - (qd(1) + qd(2))*(90*qd(1) + 90*qd(2))))) + (80*c5*(-qd(3) + qd(4)) + 80*s5*(-c3*s4*(qd(1) + qd(2)) + c4*s3*(qd(1) + qd(2))))*(-c3*c4*(qd(1) + qd(2)) + qd(5) - s3*s4*(qd(1) + qd(2)))) - (80*c6*(c5*(-c3*s4*(qd(1) + qd(2)) + c4*s3*(qd(1) + qd(2))) - s5*(-qd(3) + qd(4))) - 80*s6*(-c5*(-qd(3) + qd(4)) - s5*(-c3*s4*(qd(1) + qd(2)) + c4*s3*(qd(1) + qd(2)))))*(c3*c4*(qd(1) + qd(2)) - qd(5) + qd(6) + s3*s4*(qd(1) + qd(2)))) + m6*(c5*(c4*(c3*(c2*(- 270*qd(1)^2) - (qd(1) + qd(2))*(90*qd(1) + 90*qd(2)))) - s4*(- s3*(c2*(- 270*qd(1)^2) - (qd(1) + qd(2))*(90*qd(1) + 90*qd(2))))) - 295*c3^2*(qd(1) + qd(2))^2 + s2*(- 270*qd(1)^2) - 295*s3^2*(qd(1) + qd(2))^2)) - m7*s5*(80*c6*(c5*(c4*(c3*qd(3)*(qd(1) + qd(2)))) + qd(4)*(-c3*c4*(qd(1) + qd(2)) - s3*s4*(qd(1) + qd(2))) - s4*(- qd(3)*s3*(qd(1) + qd(2)))) + qd(5)*(-c5*(-qd(3) + qd(4)) - s5*(-c3*s4*(qd(1) + qd(2)) + c4*s3*(qd(1) + qd(2))))) - c6*(80*c5*(c4*(c3*qd(3)*(qd(1) + qd(2))) + qd(4)*(-c3*c4*(qd(1) + qd(2)) - s3*s4*(qd(1) + qd(2))) - s4*(- qd(3)*s3*(qd(1) + qd(2)))) - c5*(- 295*c3^2*(qd(1) + qd(2))^2 + s2*(- 270*qd(1)^2) - 295*s3^2*(qd(1) + qd(2))^2) + 80*qd(5)*(-c5*(-qd(3) + qd(4)) - s5*(-c3*s4*(qd(1) + qd(2)) + c4*s3*(qd(1) + qd(2)))) - s5*(c4*(c3*(c2*(- 270*qd(1)^2) - (qd(1) + qd(2))*(90*qd(1) + 90*qd(2)))) - s4*(- s3*(c2*(- 270*qd(1)^2) - (qd(1) + qd(2))*(90*qd(1) + 90*qd(2))))) + (80*c5*(-qd(3) + qd(4)) + 80*s5*(-c3*s4*(qd(1) + qd(2)) + c4*s3*(qd(1) + qd(2))))*(-c3*c4*(qd(1) + qd(2)) + qd(5) - s3*s4*(qd(1) + qd(2)))) + 80*qd(6)*(-c6*(-c5*(-qd(3) + qd(4)) - s5*(-c3*s4*(qd(1) + qd(2)) + c4*s3*(qd(1) + qd(2)))) - s6*(c5*(-c3*s4*(qd(1) + qd(2)) + c4*s3*(qd(1) + qd(2))) - s5*(-qd(3) + qd(4)))) - 80*s6*(- qd(5)*(c5*(-c3*s4*(qd(1) + qd(2)) + c4*s3*(qd(1) + qd(2))) - s5*(-qd(3) + qd(4))) - s5*(c4*(c3*qd(3)*(qd(1) + qd(2))) + qd(4)*(-c3*c4*(qd(1) + qd(2)) - s3*s4*(qd(1) + qd(2))) - s4*(- qd(3)*s3*(qd(1) + qd(2))))) - s6*(+ c5*(c4*(c3*(c2*(- 270*qd(1)^2) - (qd(1) + qd(2))*(90*qd(1) + 90*qd(2)))) - s4*(- s3*(c2*(- 270*qd(1)^2) - (qd(1) + qd(2))*(90*qd(1) + 90*qd(2))))) + 80*qd(5)*(c5*(-c3*s4*(qd(1) + qd(2)) + c4*s3*(qd(1) + qd(2))) - s5*(-qd(3) + qd(4))) + 80*s5*(c4*(c3*qd(3)*(qd(1) + qd(2))) + qd(4)*(-c3*c4*(qd(1) + qd(2)) - s3*s4*(qd(1) + qd(2))) - s4*(- qd(3)*s3*(qd(1) + qd(2)))) - s5*(- 295*c3^2*(qd(1) + qd(2))^2+ s2*(- 270*qd(1)^2) - 295*s3^2*(qd(1) + qd(2))^2) - (80*c5*(-c3*s4*(qd(1) + qd(2)) + c4*s3*(qd(1) + qd(2))) - 80*s5*(-qd(3) + qd(4)))*(-c3*c4*(qd(1) + qd(2)) + qd(5) - s3*s4*(qd(1) + qd(2)))) + (80*c6*(-c5*(-qd(3) + qd(4)) - s5*(-c3*s4*(qd(1) + qd(2)) + c4*s3*(qd(1) + qd(2)))) + 80*s6*(c5*(-c3*s4*(qd(1) + qd(2)) + c4*s3*(qd(1) + qd(2))) - s5*(-qd(3) + qd(4))))*(c3*c4*(qd(1) + qd(2)) - qd(5) + qd(6) + s3*s4*(qd(1) + qd(2)))) + 75*c2*(c5*m7*(80*c6*(c5*(c4*(c3*qd(3)*(qd(1) + qd(2))) + qd(4)*(-c3*c4*(qd(1) + qd(2)) - s3*s4*(qd(1) + qd(2))) - s4*( - qd(3)*s3*(qd(1) + qd(2)))) + qd(5)*(-c5*(-qd(3) + qd(4)) - s5*(-c3*s4*(qd(1) + qd(2)) + c4*s3*(qd(1) + qd(2))))) - c6*(80*c5*(c4*(c3*qd(3)*(qd(1) + qd(2))) + qd(4)*(-c3*c4*(qd(1) + qd(2)) - s3*s4*(qd(1) + qd(2))) - s4*(- qd(3)*s3*(qd(1) + qd(2)))) - c5*(- 295*c3^2*(qd(1) + qd(2))^2 + s2*(- 270*qd(1)^2) - 295*s3^2*(qd(1) + qd(2))^2) + 80*qd(5)*(-c5*(-qd(3) + qd(4)) - s5*(-c3*s4*(qd(1) + qd(2)) + c4*s3*(qd(1) + qd(2)))) - s5*(c4*(c3*(c2*(- 270*qd(1)^2) - (qd(1) + qd(2))*(90*qd(1) + 90*qd(2)))) - s4*(- s3*(c2*(- 270*qd(1)^2) - (qd(1) + qd(2))*(90*qd(1) + 90*qd(2))))) + (80*c5*(-qd(3) + qd(4)) + 80*s5*(-c3*s4*(qd(1) + qd(2)) + c4*s3*(qd(1) + qd(2))))*(-c3*c4*(qd(1) + qd(2)) + qd(5) - s3*s4*(qd(1) + qd(2)))) + 80*qd(6)*(-c6*(-c5*(-qd(3) + qd(4)) - s5*(-c3*s4*(qd(1) + qd(2)) + c4*s3*(qd(1) + qd(2)))) - s6*(c5*(-c3*s4*(qd(1) + qd(2)) + c4*s3*(qd(1) + qd(2))) - s5*(-qd(3) + qd(4)))) - 80*s6*(- qd(5)*(c5*(-c3*s4*(qd(1) + qd(2)) + c4*s3*(qd(1) + qd(2))) - s5*(-qd(3) + qd(4))) - s5*(c4*(c3*qd(3)*(qd(1) + qd(2))) + qd(4)*(-c3*c4*(qd(1) + qd(2)) - s3*s4*(qd(1) + qd(2))) - s4*(- qd(3)*s3*(qd(1) + qd(2))))) - s6*(c5*(c4*(c3*(c2*(- 270*qd(1)^2) - (qd(1) + qd(2))*(90*qd(1) + 90*qd(2)))) - s4*(- s3*(c2*(- 270*qd(1)^2) - (qd(1) + qd(2))*(90*qd(1) + 90*qd(2))))) + 80*qd(5)*(c5*(-c3*s4*(qd(1) + qd(2)) + c4*s3*(qd(1) + qd(2))) - s5*(-qd(3) + qd(4))) + 80*s5*(c4*(c3*qd(3)*(qd(1) + qd(2))) + qd(4)*(-c3*c4*(qd(1) + qd(2)) - s3*s4*(qd(1) + qd(2))) - s4*(- qd(3)*s3*(qd(1) + qd(2)))) - s5*(- 295*c3^2*(qd(1) + qd(2))^2 + s2*(- 270*qd(1)^2) - 295*s3^2*(qd(1) + qd(2))^2) - (80*c5*(-c3*s4*(qd(1) + qd(2)) + c4*s3*(qd(1) + qd(2))) - 80*s5*(-qd(3) + qd(4)))*(-c3*c4*(qd(1) + qd(2)) + qd(5) - s3*s4*(qd(1) + qd(2)))) + (80*c6*(-c5*(-qd(3) + qd(4)) - s5*(-c3*s4*(qd(1) + qd(2)) + c4*s3*(qd(1) + qd(2)))) + 80*s6*(c5*(-c3*s4*(qd(1) + qd(2)) + c4*s3*(qd(1) + qd(2))) - s5*(-qd(3) + qd(4))))*(c3*c4*(qd(1) + qd(2)) - qd(5) + qd(6) + s3*s4*(qd(1) + qd(2)))) + m4*(90*c3*s3*(qd(1) + qd(2))^2 - s3*(c2*(- 270*qd(1)^2) - (qd(1) + qd(2))*(90*qd(1) + 90*qd(2)))) + m5*(- 295*c3^2*(qd(1) + qd(2))^2 + s2*(- 270*qd(1)^2) - 295*s3^2*(qd(1) + qd(2))^2 - (-c3*c4*(qd(1) + qd(2)) - s3*s4*(qd(1) + qd(2)))*(295*c3*c4*(qd(1) + qd(2)) + 295*s3*s4*(qd(1) + qd(2))) + (-295*c3*s4*(qd(1) + qd(2)) + 295*c4*s3*(qd(1) + qd(2)))*(-c3*s4*(qd(1) + qd(2)) + c4*s3*(qd(1) + qd(2)))) - m6*(-c4*(-s3*(c2*(-270*qd(1)^2) - (qd(1) + qd(2))*(90*qd(1) + 90*qd(2)))) - s4*(c3*(c2*(- 270*qd(1)^2) - (qd(1) + qd(2))*(90*qd(1) + 90*qd(2))))) + m7*s5*(80*c6*(- qd(5)*(c5*(-c3*s4*(qd(1) + qd(2)) + c4*s3*(qd(1) + qd(2))) - s5*(-qd(3) + qd(4))) - s5*(c4*(c3*qd(3)*(qd(1) + qd(2))) + qd(4)*(-c3*c4*(qd(1) + qd(2)) - s3*s4*(qd(1) + qd(2))) - s4*(- qd(3)*s3*(qd(1) + qd(2))))) + c6*(c5*(c4*(c3*(c2*(- 270*qd(1)^2) - (qd(1) + qd(2))*(90*qd(1) + 90*qd(2)))) - s4*(- s3*(c2*(- 270*qd(1)^2) - (qd(1) + qd(2))*(90*qd(1) + 90*qd(2))))) + 80*qd(5)*(c5*(-c3*s4*(qd(1) + qd(2)) + c4*s3*(qd(1) + qd(2))) - s5*(-qd(3) + qd(4))) + 80*s5*(c4*(c3*qd(3)*(qd(1) + qd(2))) + qd(4)*(-c3*c4*(qd(1) + qd(2)) - s3*s4*(qd(1) + qd(2))) - qd(3)*s3*(qd(1) + qd(2)))) - s5*(- 295*c3^2*(qd(1) + qd(2))^2 + s2*(- 270*qd(1)^2) - 295*s3^2*(qd(1) + qd(2))^2) - (80*c5*(-c3*s4*(qd(1) + qd(2)) + c4*s3*(qd(1) + qd(2))) - 80*s5*(-qd(3) + qd(4)))*(-c3*c4*(qd(1) + qd(2)) + qd(5) - s3*s4*(qd(1) + qd(2)))) + 80*qd(6)*(c6*(c5*(-c3*s4*(qd(1) + qd(2)) + c4*s3*(qd(1) + qd(2))) - s5*(-qd(3) + qd(4))) - s6*(-c5*(-qd(3) + qd(4)) - s5*(-c3*s4*(qd(1) + qd(2)) + c4*s3*(qd(1) + qd(2))))) + 80*s6*(c5*(c4*(c3*qd(3)*(qd(1) + qd(2))) + qd(4)*(-c3*c4*(qd(1) + qd(2)) - s3*s4*(qd(1) + qd(2))) - s4*(- qd(3)*s3*(qd(1) + qd(2)))) + qd(5)*(-c5*(-qd(3) + qd(4)) - s5*(-c3*s4*(qd(1) + qd(2)) + c4*s3*(qd(1) + qd(2))))) - s6*(80*c5*(c4*(c3*qd(3)*(qd(1) + qd(2))) + qd(4)*(-c3*c4*(qd(1) + qd(2)) - s3*s4*(qd(1) + qd(2))) - s4*(- qd(3)*s3*(qd(1) + qd(2)))) - c5*(- 295*c3^2*(qd(1) + qd(2))^2 + s2*(- 270*qd(1)^2) - 295*s3^2*(qd(1) + qd(2))^2) + 80*qd(5)*(-c5*(-qd(3) + qd(4)) - s5*(-c3*s4*(qd(1) + qd(2)) + c4*s3*(qd(1) + qd(2)))) - s5*(c4*(c3*(c2*(- 270*qd(1)^2) - (qd(1) + qd(2))*(90*qd(1) + 90*qd(2)))) - s4*(- s3*(c2*(- 270*qd(1)^2) - (qd(1) + qd(2))*(90*qd(1) + 90*qd(2))))) + (80*c5*(-qd(3) + qd(4)) + 80*s5*(-c3*s4*(qd(1) + qd(2)) + c4*s3*(qd(1) + qd(2))))*(-c3*c4*(qd(1) + qd(2)) + qd(5) - s3*s4*(qd(1) + qd(2)))) - (80*c6*(c5*(-c3*s4*(qd(1) + qd(2)) + c4*s3*(qd(1) + qd(2))) - s5*(-qd(3) + qd(4))) - 80*s6*(-c5*(-qd(3) + qd(4)) - s5*(-c3*s4*(qd(1) + qd(2)) + c4*s3*(qd(1) + qd(2)))))*(c3*c4*(qd(1) + qd(2)) - qd(5) + qd(6) + s3*s4*(qd(1) + qd(2)))) - 0.0247925*c3*qd(3)*(qd(1) + qd(2)) - c3*(qd(1) + qd(2))*(-0.00947011*c3*(qd(1) + qd(2)) - 0.0247925*qd(3) + 0.775113*s3*(qd(1) + qd(2))) + c3*(-0.020170031*c4*(- qd(3)*s3*(qd(1) + qd(2))) - 0.00163355*c4*(c3*qd(3)*(qd(1) + qd(2))) - c4*(3.29301e-6*c4*(- qd(3)*s3*(qd(1) + qd(2))) - 295*c5*m7*(80*c6*(- qd(5)*(c5*(-c3*s4*(qd(1) + qd(2)) + c4*s3*(qd(1) + qd(2))) - s5*(-qd(3) + qd(4))) - s5*(c4*(c3*qd(3)*(qd(1) + qd(2))) + qd(4)*(-c3*c4*(qd(1) + qd(2)) - s3*s4*(qd(1) + qd(2))) - qd(3)*s3*(qd(1) + qd(2))))) + c6*(c5*(c4*(c3*(c2*(- 270*qd(1)^2) - (qd(1) + qd(2))*(90*qd(1) + 90*qd(2)))) - s4*(- s3*(c2*(- 270*qd(1)^2) - (qd(1) + qd(2))*(90*qd(1) + 90*qd(2))))) + 80*qd(5)*(c5*(-c3*s4*(qd(1) + qd(2)) + c4*s3*(qd(1) + qd(2))) - s5*(-qd(3) + qd(4))) + 80*s5*(c4*(c3*qd(3)*(qd(1) + qd(2))) + qd(4)*(-c3*c4*(qd(1) + qd(2)) - s3*s4*(qd(1) + qd(2))) - qd(3)*s3*(qd(1) + qd(2)))) - s5*(- 295*c3^2*(qd(1) + qd(2))^2 + s2*(- 270*qd(1)^2) - 295*s3^2*(qd(1) + qd(2))^2) - (80*c5*(-c3*s4*(qd(1) + qd(2)) + c4*s3*(qd(1) + qd(2))) - 80*s5*(-qd(3) + qd(4)))*(-c3*c4*(qd(1) + qd(2)) + qd(5) - s3*s4*(qd(1) + qd(2)))) + 80*qd(6)*(c6*(c5*(-c3*s4*(qd(1) + qd(2)) + c4*s3*(qd(1) + qd(2))) - s5*(-qd(3) + qd(4))) - s6*(-c5*(-qd(3) + qd(4)) - s5*(-c3*s4*(qd(1) + qd(2)) + c4*s3*(qd(1) + qd(2))))) + 80*s6*(c5*(c4*(c3*qd(3)*(qd(1) + qd(2))) + qd(4)*(-c3*c4*(qd(1) + qd(2)) - s3*s4*(qd(1) + qd(2))) - s4*(- qd(3)*s3*(qd(1) + qd(2)))) + qd(5)*(-c5*(-qd(3) + qd(4)) - s5*(-c3*s4*(qd(1) + qd(2)) + c4*s3*(qd(1) + qd(2))))) - s6*(80*c5*(c4*(c3*qd(3)*(qd(1) + qd(2))) + qd(4)*(-c3*c4*(qd(1) + qd(2)) - s3*s4*(qd(1) + qd(2))) - s4*(- qd(3)*s3*(qd(1) + qd(2)))) - c5*(- 295*c3^2*(qd(1) + qd(2))^2 + s2*(- 270*qd(1)^2) - 295*s3^2*(qd(1) + qd(2))^2) + 80*qd(5)*(-c5*(-qd(3) + qd(4)) - s5*(-c3*s4*(qd(1) + qd(2)) + c4*s3*(qd(1) + qd(2)))) - s5*(c4*(c3*(c2*(- 270*qd(1)^2) - (qd(1) + qd(2))*(90*qd(1) + 90*qd(2)))) - s4*(- s3*(c2*(- 270*qd(1)^2) - (qd(1) + qd(2))*(90*qd(1) + 90*qd(2))))) + (80*c5*(-qd(3) + qd(4)) + 80*s5*(-c3*s4*(qd(1) + qd(2)) + c4*s3*(qd(1) + qd(2))))*(-c3*c4*(qd(1) + qd(2)) + qd(5) - s3*s4*(qd(1) + qd(2)))) - (80*c6*(c5*(-c3*s4*(qd(1) + qd(2)) + c4*s3*(qd(1) + qd(2))) - s5*(-qd(3) + qd(4))) - 80*s6*(-c5*(-qd(3) + qd(4)) - s5*(-c3*s4*(qd(1) + qd(2)) + c4*s3*(qd(1) + qd(2)))))*(c3*c4*(qd(1) + qd(2)) - qd(5) + qd(6) + s3*s4*(qd(1) + qd(2)))) - 0.000409305*c5*(c4*(c3*qd(3)*(qd(1) + qd(2)) ) + qd(4)*(-c3*c4*(qd(1) + qd(2)) - s3*s4*(qd(1) + qd(2))) - s4*(- qd(3)*s3*(qd(1) + qd(2)))) - 295*m6*(c5*(c4*(c3*(c2*(- 270*qd(1)^2) - (qd(1) + qd(2))*(90*qd(1) + 90*qd(2)))) - s4*(- s3*(c2*(- 270*qd(1)^2) - (qd(1) + qd(2))*(90*qd(1) + 90*qd(2))))) - s5*(- 295*c3^2*(qd(1) + qd(2))^2 + s2*(- 270*qd(1)^2) - 295*s3^2*(qd(1) + qd(2))^2)) + 295*m7*s5*(80*c6*(c5*(c4*(c3*qd(3)*(qd(1) + qd(2))) + qd(4)*(-c3*c4*(qd(1) + qd(2)) - s3*s4*(qd(1) + qd(2))) - s4*(- qd(3)*s3*(qd(1) + qd(2)))) + qd(5)*(-c5*(-qd(3) + qd(4)) - s5*(-c3*s4*(qd(1) + qd(2)) + c4*s3*(qd(1) + qd(2))))) - c6*(80*c5*(c4*(c3*qd(3)*(qd(1) + qd(2))) + qd(4)*(-c3*c4*(qd(1) + qd(2)) - s3*s4*(qd(1) + qd(2))) - s4*(- qd(3)*s3*(qd(1) + qd(2)))) - c5*(- 295*c3^2*(qd(1) + qd(2))^2 + s2*(- 270*qd(1)^2) - 295*s3^2*(qd(1) + qd(2))^2) + 80*qd(5)*(-c5*(-qd(3) + qd(4)) - s5*(-c3*s4*(qd(1) + qd(2)) + c4*s3*(qd(1) + qd(2)))) - s5*(c4*(c3*(c2*(- 270*qd(1)^2) - (qd(1) + qd(2))*(90*qd(1) + 90*qd(2)))) - s4*(- s3*(c2*(- 270*qd(1)^2) - (qd(1) + qd(2))*(90*qd(1) + 90*qd(2))))) + (80*c5*(-qd(3) + qd(4)) + 80*s5*(-c3*s4*(qd(1) + qd(2)) + c4*s3*(qd(1) + qd(2))))*(-c3*c4*(qd(1) + qd(2)) + qd(5) - s3*s4*(qd(1) + qd(2)))) + 80*qd(6)*(-c6*(-c5*(-qd(3) + qd(4)) - s5*(-c3*s4*(qd(1) + qd(2)) + c4*s3*(qd(1) + qd(2)))) - s6*(c5*(-c3*s4*(qd(1) + qd(2)) + c4*s3*(qd(1) + qd(2))) - s5*(-qd(3) + qd(4)))) - 80*s6*( - qd(5)*(c5*(-c3*s4*(qd(1) + qd(2)) + c4*s3*(qd(1) + qd(2))) - s5*(-qd(3) + qd(4))) - s5*(c4*(c3*qd(3)*(qd(1) + qd(2))) + qd(4)*(-c3*c4*(qd(1) + qd(2)) - s3*s4*(qd(1) + qd(2))) - s4*(- qd(3)*s3*(qd(1) + qd(2))))) - s6*(c5*(c4*(c3*(c2*(- 270*qd(1)^2) - (qd(1) + qd(2))*(90*qd(1) + 90*qd(2)))) - s4*(- s3*(c2*(- 270*qd(1)^2) - (qd(1) + qd(2))*(90*qd(1) + 90*qd(2))))) + 80*qd(5)*(c5*(-c3*s4*(qd(1) + qd(2)) + c4*s3*(qd(1) + qd(2))) - s5*(-qd(3) + qd(4))) + 80*s5*(c4*(c3*qd(3)*(qd(1) + qd(2))) + qd(4)*(-c3*c4*(qd(1) + qd(2)) - s3*s4*(qd(1) + qd(2))) - s4*(- qd(3)*s3*(qd(1) + qd(2)))) - s5*(- 295*c3^2*(qd(1) + qd(2))^2 + s2*(- 270*qd(1)^2) - 295*s3^2*(qd(1) + qd(2))^2) - (80*c5*(-c3*s4*(qd(1) + qd(2)) + c4*s3*(qd(1) + qd(2))) - 80*s5*(-qd(3) + qd(4)))*(-c3*c4*(qd(1) + qd(2)) + qd(5) - s3*s4*(qd(1) + qd(2)))) + (80*c6*(-c5*(-qd(3) + qd(4)) - s5*(-c3*s4*(qd(1) + qd(2)) + c4*s3*(qd(1) + qd(2)))) + 80*s6*(c5*(-c3*s4*(qd(1) + qd(2)) + c4*s3*(qd(1) + qd(2))) - s5*(-qd(3) + qd(4))))*(c3*c4*(qd(1) + qd(2)) - qd(5) + qd(6) + s3*s4*(qd(1) + qd(2)))) + 3.29301e-6*qd(4)*(-c3*s4*(qd(1) + qd(2)) + c4*s3*(qd(1) + qd(2))) - 0.000409305*qd(5)*(-c5*(-qd(3) + qd(4)) - s5*(-c3*s4*(qd(1) + qd(2)) + c4*s3*(qd(1) + qd(2)))) - 0.00355535*qd(5)*(c5*(-c3*s4*(qd(1) + qd(2)) + c4*s3*(qd(1) + qd(2))) - s5*(-qd(3) + qd(4))) + 3.29301e-6*s4*(c3*qd(3)*(qd(1) + qd(2))) - 0.00355535*s5*(c4*(c3*qd(3)*(qd(1) + qd(2))) + qd(4)*(-c3*c4*(qd(1) + qd(2)) - s3*s4*(qd(1) + qd(2))) - s4*(- qd(3)*s3*(qd(1) + qd(2)))) - (c5*(-c3*s4*(qd(1) + qd(2)) + c4*s3*(qd(1) + qd(2))) - s5*(-qd(3) + qd(4)))*(-0.00358942*c3*c4*(qd(1) + qd(2)) + 0.00358942*qd(5) - 0.00358942*s3*s4*(qd(1) + qd(2))) - (-c6*(-c5*(-qd(3) + qd(4)) - s5*(-c3*s4*(qd(1) + qd(2)) + c4*s3*(qd(1) + qd(2)))) - s6*(c5*(-c3*s4*(qd(1) + qd(2)) + c4*s3*(qd(1) + qd(2))) - s5*(-qd(3) + qd(4))))*(6.20477e-6*c6*(c5*(-c3*s4*(qd(1) + qd(2)) + c4*s3*(qd(1) + qd(2))) - s5*(-qd(3) + qd(4))) - 6.20477e-6*s6*(-c5*(-qd(3) + qd(4)) - s5*(-c3*s4*(qd(1) + qd(2)) + c4*s3*(qd(1) + qd(2))))) + (-3.01352e-6*c6*(-c5*(-qd(3) + qd(4)) - s5*(-c3*s4*(qd(1) + qd(2)) + c4*s3*(qd(1) + qd(2)))) - 3.01352e-6*s6*(c5*(-c3*s4*(qd(1) + qd(2)) + c4*s3*(qd(1) + qd(2))) - s5*(-qd(3) + qd(4))))*(c6*(c5*(-c3*s4*(qd(1) + qd(2)) + c4*s3*(qd(1) + qd(2))) - s5*(-qd(3) + qd(4))) - s6*(-c5*(-qd(3) + qd(4)) - s5*(-c3*s4*(qd(1) + qd(2)) + c4*s3*(qd(1) + qd(2))))) + (-c3*c4*(qd(1) + qd(2)) + qd(5) - s3*s4*(qd(1) + qd(2)))*(0.000409305*c5*(-qd(3) + qd(4)) + 0.00151607*c5*(-c3*s4*(qd(1) + qd(2)) + c4*s3*(qd(1) + qd(2))) - 0.00151607*s5*(-qd(3) + qd(4)) + 0.000409305*s5*(-c3*s4*(qd(1) + qd(2)) + c4*s3*(qd(1) + qd(2)))) - 90*c5*m7*(80*c6*(c5*(c4*(c3*qd(3)*(qd(1) + qd(2))) + qd(4)*(-c3*c4*(qd(1) + qd(2)) - s3*s4*(qd(1) + qd(2))) - s4*(- qd(3)*s3*(qd(1) + qd(2)))) + qd(5)*(-c5*(-qd(3) + qd(4)) - s5*(-c3*s4*(qd(1) + qd(2)) + c4*s3*(qd(1) + qd(2))))) - c6*(80*c5*(c4*(c3*qd(3)*(qd(1) + qd(2))) + qd(4)*(-c3*c4*(qd(1) + qd(2)) - s3*s4*(qd(1) + qd(2))) - s4*(- qd(3)*s3*(qd(1) + qd(2)))) - c5*( - 295*c3^2*(qd(1) + qd(2))^2 + s2*(- 270*qd(1)^2) - 295*s3^2*(qd(1) + qd(2))^2) + 80*qd(5)*(-c5*(-qd(3) + qd(4)) - s5*(-c3*s4*(qd(1) + qd(2)) + c4*s3*(qd(1) + qd(2)))) - s5*(c4*(c3*(c2*(- 270*qd(1)^2) - (qd(1) + qd(2))*(90*qd(1) + 90*qd(2)))) - s4*(- s3*(c2*(- 270*qd(1)^2) - (qd(1) + qd(2))*(90*qd(1) + 90*qd(2))))) + (80*c5*(-qd(3) + qd(4)) + 80*s5*(-c3*s4*(qd(1) + qd(2)) + c4*s3*(qd(1) + qd(2))))*(-c3*c4*(qd(1) + qd(2)) + qd(5) - s3*s4*(qd(1) + qd(2)))) + 80*qd(6)*(-c6*(-c5*(-qd(3) + qd(4)) - s5*(-c3*s4*(qd(1) + qd(2)) + c4*s3*(qd(1) + qd(2)))) - s6*(c5*(-c3*s4*(qd(1) + qd(2)) + c4*s3*(qd(1) + qd(2))) - s5*(-qd(3) + qd(4)))) - 80*s6*(- qd(5)*(c5*(-c3*s4*(qd(1) + qd(2)) + c4*s3*(qd(1) + qd(2))) - s5*(-qd(3) + qd(4))) - s5*(c4*(c3*qd(3)*(qd(1) + qd(2))) + qd(4)*(-c3*c4*(qd(1) + qd(2)) - s3*s4*(qd(1) + qd(2))) - s4*(- qd(3)*s3*(qd(1) + qd(2))))) - s6*(c5*(c4*(c3*(c2*(- 270*qd(1)^2) - (qd(1) + qd(2))*(90*qd(1) + 90*qd(2)))) - s4*(- s3*(c2*( - 270*qd(1)^2) - (qd(1) + qd(2))*(90*qd(1) + 90*qd(2))))) + 80*qd(5)*(c5*(-c3*s4*(qd(1) + qd(2)) + c4*s3*(qd(1) + qd(2))) - s5*(-qd(3) + qd(4))) + 80*s5*(c4*(c3*qd(3)*(qd(1) + qd(2))) + qd(4)*(-c3*c4*(qd(1) + qd(2)) - s3*s4*(qd(1) + qd(2))) - s4*(- qd(3)*s3*(qd(1) + qd(2)))) - s5*(- 295*c3^2*(qd(1) + qd(2))^2 + s2*(- 270*qd(1)^2) - 295*s3^2*(qd(1) + qd(2))^2) - (80*c5*(-c3*s4*(qd(1) + qd(2)) + c4*s3*(qd(1) + qd(2))) - 80*s5*(-qd(3) + qd(4)))*(-c3*c4*(qd(1) + qd(2)) + qd(5) - s3*s4*(qd(1) + qd(2)))) + (80*c6*(-c5*(-qd(3) + qd(4)) - s5*(-c3*s4*(qd(1) + qd(2)) + c4*s3*(qd(1) + qd(2)))) + 80*s6*(c5*(-c3*s4*(qd(1) + qd(2)) + c4*s3*(qd(1) + qd(2))) - s5*(-qd(3) + qd(4))))*(c3*c4*(qd(1) + qd(2)) - qd(5) + qd(6) + s3*s4*(qd(1) + qd(2)))) - 90*m5*(- 295*c3^2*(qd(1) + qd(2))^2 + s2*(- 270*qd(1)^2) - 295*s3^2*(qd(1) + qd(2))^2 - (-c3*c4*(qd(1) + qd(2)) - s3*s4*(qd(1) + qd(2)))*(295*c3*c4*(qd(1) + qd(2)) + 295*s3*s4*(qd(1) + qd(2))) + (-295*c3*s4*(qd(1) + qd(2)) + 295*c4*s3*(qd(1) + qd(2)))*(-c3*s4*(qd(1) + qd(2)) + c4*s3*(qd(1) + qd(2)))) + 90*m6*(-c4*(- s3*(c2*(- 270*qd(1)^2) - (qd(1) + qd(2))*(90*qd(1) + 90*qd(2)))) - s4*(c3*(c2*(- 270*qd(1)^2) - (qd(1) + qd(2))*(90*qd(1) + 90*qd(2))))) - 90*m7*s5*(80*c6*(- qd(5)*(c5*(-c3*s4*(qd(1) + qd(2)) + c4*s3*(qd(1) + qd(2))) - s5*(-qd(3) + qd(4))) - s5*(c4*(c3*qd(3)*(qd(1) + qd(2)))) + qd(4)*(-c3*c4*(qd(1) + qd(2)) - s3*s4*(qd(1) + qd(2))) - s4*(- qd(3)*s3*(qd(1) + qd(2))))) + c6*(c5*(c4*(c3*(c2*(- 270*qd(1)^2) - (qd(1) + qd(2))*(90*qd(1) + 90*qd(2)))) - s4*(- s3*(c2*(- 270*qd(1)^2) - (qd(1) + qd(2))*(90*qd(1) + 90*qd(2))))) + 80*qd(5)*(c5*(-c3*s4*(qd(1) + qd(2)) + c4*s3*(qd(1) + qd(2))) - s5*(-qd(3) + qd(4))) + 80*s5*(c4*(c3*qd(3)*(qd(1) + qd(2))) + qd(4)*(-c3*c4*(qd(1) + qd(2)) - s3*s4*(qd(1) + qd(2))) - s4*(- qd(3)*s3*(qd(1) + qd(2)))) - s5*(- 295*c3^2*(qd(1) + qd(2))^2 + s2*(- 270*qd(1)^2) - 295*s3^2*(qd(1) + qd(2))^2) - (80*c5*(-c3*s4*(qd(1) + qd(2)) + c4*s3*(qd(1) + qd(2))) - 80*s5*(-qd(3) + qd(4)))*(-c3*c4*(qd(1) + qd(2)) + qd(5) - s3*s4*(qd(1) + qd(2)))) + 80*qd(6)*(c6*(c5*(-c3*s4*(qd(1) + qd(2)) + c4*s3*(qd(1) + qd(2))) - s5*(-qd(3) + qd(4))) - s6*(-c5*(-qd(3) + qd(4)) - s5*(-c3*s4*(qd(1) + qd(2)) + c4*s3*(qd(1) + qd(2))))) + 80*s6*(c5*(c4*(c3*qd(3)*(qd(1) + qd(2))) + qd(4)*(-c3*c4*(qd(1) + qd(2)) - s3*s4*(qd(1) + qd(2))) - s4*(- qd(3)*s3*(qd(1) + qd(2)))) + qd(5)*(-c5*(-qd(3) + qd(4)) - s5*(-c3*s4*(qd(1) + qd(2)) + c4*s3*(qd(1) + qd(2))))) - s6*(80*c5*(c4*(c3*qd(3)*(qd(1) + qd(2))) + qd(4)*(-c3*c4*(qd(1) + qd(2)) - s3*s4*(qd(1) + qd(2))) - s4*(- qd(3)*s3*(qd(1) + qd(2)))) - c5*( - 295*c3^2*(qd(1) + qd(2))^2 + s2*(- 270*qd(1)^2) - 295*s3^2*(qd(1) + qd(2))^2) + 80*qd(5)*(-c5*(-qd(3) + qd(4)) - s5*(-c3*s4*(qd(1) + qd(2)) + c4*s3*(qd(1) + qd(2)))) - s5*(c4*(c3*(c2*(- 270*qd(1)^2) - (qd(1) + qd(2))*(90*qd(1) + 90*qd(2)))) - s4*(- s3*(c2*(- 270*qd(1)^2) - (qd(1) + qd(2))*(90*qd(1) + 90*qd(2))))) + (80*c5*(-qd(3) + qd(4)) + 80*s5*(-c3*s4*(qd(1) + qd(2)) + c4*s3*(qd(1) + qd(2))))*(-c3*c4*(qd(1) + qd(2)) + qd(5) - s3*s4*(qd(1) + qd(2)))) - (80*c6*(c5*(-c3*s4*(qd(1) + qd(2)) + c4*s3*(qd(1) + qd(2))) - s5*(-qd(3) + qd(4))) - 80*s6*(-c5*(-qd(3) + qd(4)) - s5*(-c3*s4*(qd(1) + qd(2)) + c4*s3*(qd(1) + qd(2)))))*(c3*c4*(qd(1) + qd(2)) - qd(5) + qd(6) + s3*s4*(qd(1) + qd(2))) - 0.00163355*qd(4)*(-c3*c4*(qd(1) + qd(2)) - s3*s4*(qd(1) + qd(2))) - 0.020170031*qd(4)*(-c3*s4*(qd(1) + qd(2)) + c4*s3*(qd(1) + qd(2))) + 0.00163355*s4*(- qd(3)*s3*(qd(1) + qd(2))) - 0.020170031*s4*(c3*qd(3)*(qd(1) + qd(2))) - s4*(0.00151607*c5*(c4*(c3*qd(3)*(qd(1) + qd(2))) + qd(4)*(-c3*c4*(qd(1) + qd(2)) - s3*s4*(qd(1) + qd(2))) - s4*(- qd(3)*s3*(qd(1) + qd(2)))) + c5*(6.20477e-6*c6*(c5*(c4*(c3*qd(3)*(qd(1) + qd(2))) + qd(4)*(-c3*c4*(qd(1) + qd(2)) - s3*s4*(qd(1) + qd(2))) - s4*(- qd(3)*s3*(qd(1) + qd(2)))) + qd(5)*(-c5*(-qd(3) + qd(4)) - s5*(-c3*s4*(qd(1) + qd(2)) + c4*s3*(qd(1) + qd(2))))) + 6.20477e-6*qd(6)*(-c6*(-c5*(-qd(3) + qd(4)) - s5*(-c3*s4*(qd(1) + qd(2)) + c4*s3*(qd(1) + qd(2)))) - s6*(c5*(-c3*s4*(qd(1) + qd(2)) + c4*s3*(qd(1) + qd(2))) - s5*(-qd(3) + qd(4)))) - 6.20477e-6*s6*(- qd(5)*(c5*(-c3*s4*(qd(1) + qd(2)) + c4*s3*(qd(1) + qd(2))) - s5*(-qd(3) + qd(4))) - s5*(c4*(c3*qd(3)*(qd(1) + qd(2))) + qd(4)*(-c3*c4*(qd(1) + qd(2)) - s3*s4*(qd(1) + qd(2))) - s4*(- qd(3)*s3*(qd(1) + qd(2))))) + (-c6*(-c5*(-qd(3) + qd(4)) - s5*(-c3*s4*(qd(1) + qd(2)) + c4*s3*(qd(1) + qd(2)))) - s6*(c5*(-c3*s4*(qd(1) + qd(2)) + c4*s3*(qd(1) + qd(2))) - s5*(-qd(3) + qd(4))))*(3.29301e-6*c3*c4*(qd(1) + qd(2)) - 3.29301e-6*qd(5) + 3.29301e-6*qd(6) + 3.29301e-6*s3*s4*(qd(1) + qd(2))) - (-3.01352e-6*c6*(-c5*(-qd(3) + qd(4)) - s5*(-c3*s4*(qd(1) + qd(2)) + c4*s3*(qd(1) + qd(2)))) - 3.01352e-6*s6*(c5*(-c3*s4*(qd(1) + qd(2)) + c4*s3*(qd(1) + qd(2))) - s5*(-qd(3) + qd(4))))*(c3*c4*(qd(1) + qd(2)) - qd(5) + qd(6) + s3*s4*(qd(1) + qd(2)))) + 295*m6*(-c5*( - 295*c3^2*(qd(1) + qd(2))^2 + s2*(- 270*qd(1)^2) - 295*s3^2*(qd(1) + qd(2))^2) - s5*(c4*(c3*(c2*(- 270*qd(1)^2) - (qd(1) + qd(2))*(90*qd(1) + 90*qd(2)))) - s4*(- s3*(c2*(- 270*qd(1)^2) - (qd(1) + qd(2))*(90*qd(1) + 90*qd(2)))))) + 295*m7*(c4*(- s3*(c2*(- 270*qd(1)^2) - (qd(1) + qd(2))*(90*qd(1) + 90*qd(2)))) + s4*(c3*(c2*(- 270*qd(1)^2) - (qd(1) + qd(2))*(90*qd(1) + 90*qd(2)))) + (-c5*(-qd(3) + qd(4)) - s5*(-c3*s4*(qd(1) + qd(2)) + c4*s3*(qd(1) + qd(2))))*(80*c5*(-qd(3) + qd(4)) + 80*s5*(-c3*s4*(qd(1) + qd(2)) + c4*s3*(qd(1) + qd(2)))) - (c5*(-c3*s4*(qd(1) + qd(2)) + c4*s3*(qd(1) + qd(2))) - s5*(-qd(3) + qd(4)))*(80*c5*(-c3*s4*(qd(1) + qd(2)) + c4*s3*(qd(1) + qd(2))) - 80*s5*(-qd(3) + qd(4))) - (-c6*(-c5*(-qd(3) + qd(4)) - s5*(-c3*s4*(qd(1) + qd(2)) + c4*s3*(qd(1) + qd(2)))) - s6*(c5*(-c3*s4*(qd(1) + qd(2)) + c4*s3*(qd(1) + qd(2))) - s5*(-qd(3) + qd(4))))*(80*c6*(-c5*(-qd(3) + qd(4)) - s5*(-c3*s4*(qd(1) + qd(2)) + c4*s3*(qd(1) + qd(2)))) + 80*s6*(c5*(-c3*s4*(qd(1) + qd(2)) + c4*s3*(qd(1) + qd(2))) - s5*(-qd(3) + qd(4)))) + (c6*(c5*(-c3*s4*(qd(1) + qd(2)) + c4*s3*(qd(1) + qd(2))) - s5*(-qd(3) + qd(4))) - s6*(-c5*(-qd(3) + qd(4)) - s5*(-c3*s4*(qd(1) + qd(2)) + c4*s3*(qd(1) + qd(2)))))*(80*c6*(c5*(-c3*s4*(qd(1) + qd(2)) + c4*s3*(qd(1) + qd(2))) - s5*(-qd(3) + qd(4))) - 80*s6*(-c5*(-qd(3) + qd(4)) - s5*(-c3*s4*(qd(1) + qd(2)) + c4*s3*(qd(1) + qd(2)))))) + 0.00151607*qd(5)*(-c5*(-qd(3) + qd(4)) - s5*(-c3*s4*(qd(1) + qd(2)) + c4*s3*(qd(1) + qd(2)))) + 0.000409305*qd(5)*(c5*(-c3*s4*(qd(1) + qd(2)) + c4*s3*(qd(1) + qd(2))) - s5*(-qd(3) + qd(4))) + 0.000409305*s5*(c4*(c3*qd(3)*(qd(1) + qd(2)))) + qd(4)*(-c3*c4*(qd(1) + qd(2)) - s3*s4*(qd(1) + qd(2))) - s4*(- qd(3)*s3*(qd(1) + qd(2)))) - s5*(-3.01352e-6*c6*( - qd(5)*(c5*(-c3*s4*(qd(1) + qd(2)) + c4*s3*(qd(1) + qd(2))) - s5*(-qd(3) + qd(4))) - s5*(c4*(c3*qd(3)*(qd(1) + qd(2))) + qd(4)*(-c3*c4*(qd(1) + qd(2)) - s3*s4*(qd(1) + qd(2))) - qd(3)*s3*(qd(1) + qd(2))))) - 3.01352e-6*qd(6)*(c6*(c5*(-c3*s4*(qd(1) + qd(2)) + c4*s3*(qd(1) + qd(2))) - s5*(-qd(3) + qd(4))) - s6*(-c5*(-qd(3) + qd(4)) - s5*(-c3*s4*(qd(1) + qd(2)) + c4*s3*(qd(1) + qd(2))))) - 3.01352e-6*s6*(c5*(c4*(c3*qd(3)*(qd(1) + qd(2))) + qd(4)*(-c3*c4*(qd(1) + qd(2)) - s3*s4*(qd(1) + qd(2))) - s4*( - qd(3)*s3*(qd(1) + qd(2)))) + qd(5)*(-c5*(-qd(3) + qd(4)) - s5*(-c3*s4*(qd(1) + qd(2)) + c4*s3*(qd(1) + qd(2))))) + (6.20477e-6*c6*(c5*(-c3*s4*(qd(1) + qd(2)) + c4*s3*(qd(1) + qd(2))) - s5*(-qd(3) + qd(4))) - 6.20477e-6*s6*(-c5*(-qd(3) + qd(4)) - s5*(-c3*s4*(qd(1) + qd(2)) + c4*s3*(qd(1) + qd(2)))))*(c3*c4*(qd(1) + qd(2)) - qd(5) + qd(6) + s3*s4*(qd(1) + qd(2))) - (c6*(c5*(-c3*s4*(qd(1) + qd(2)) + c4*s3*(qd(1) + qd(2))) - s5*(-qd(3) + qd(4))) - s6*(-c5*(-qd(3) + qd(4)) - s5*(-c3*s4*(qd(1) + qd(2)) + c4*s3*(qd(1) + qd(2)))))*(3.29301e-6*c3*c4*(qd(1) + qd(2)) - 3.29301e-6*qd(5) + 3.29301e-6*qd(6) + 3.29301e-6*s3*s4*(qd(1) + qd(2))) + (-c5*(-qd(3) + qd(4)) - s5*(-c3*s4*(qd(1) + qd(2)) + c4*s3*(qd(1) + qd(2))))*(-0.00358942*c3*c4*(qd(1) + qd(2)) + 0.00358942*qd(5) - 0.00358942*s3*s4*(qd(1) + qd(2))) - (-c3*c4*(qd(1) + qd(2)) + qd(5) - s3*s4*(qd(1) + qd(2)))*(-0.00355535*c5*(-qd(3) + qd(4)) - 0.000409305*c5*(-c3*s4*(qd(1) + qd(2)) + c4*s3*(qd(1) + qd(2))) + 0.000409305*s5*(-qd(3) + qd(4)) - 0.00355535*s5*(-c3*s4*(qd(1) + qd(2)) + c4*s3*(qd(1) + qd(2)))) + (-qd(3) + qd(4))*(0.00163355*c3*c4*(qd(1) + qd(2)) - 0.00950111*c3*s4*(qd(1) + qd(2)) + 0.00950111*c4*s3*(qd(1) + qd(2)) + 8.41256e-6*qd(3) - 8.41256e-6*qd(4) + 0.00163355*s3*s4*(qd(1) + qd(2))) - (-c3*s4*(qd(1) + qd(2)) + c4*s3*(qd(1) + qd(2)))*(2.69102e-6*c3*c4*(qd(1) + qd(2)) + 8.41256e-6*c3*s4*(qd(1) + qd(2)) - 8.41256e-6*c4*s3*(qd(1) + qd(2)) - 0.024130024*qd(3) + 0.024130024*qd(4) + 2.69102e-6*s3*s4*(qd(1) + qd(2))) + 270*c5*m7*(80*c6*(c5*(c4*(c3*qd(3)*(qd(1) + qd(2))) + qd(4)*(-c3*c4*(qd(1) + qd(2)) - s3*s4*(qd(1) + qd(2))) - s4*( - qd(3)*s3*(qd(1) + qd(2)))) + qd(5)*(-c5*(-qd(3) + qd(4)) - s5*(-c3*s4*(qd(1) + qd(2)) + c4*s3*(qd(1) + qd(2))))) - c6*(80*c5*(c4*(c3*qd(3)*(qd(1) + qd(2))) + qd(4)*(-c3*c4*(qd(1) + qd(2)) - s3*s4*(qd(1) + qd(2))) - s4*(- qd(3)*s3*(qd(1) + qd(2)))) - c5*(- 295*c3^2*(qd(1) + qd(2))^2 + s2*(- 270*qd(1)^2) - 295*s3^2*(qd(1) + qd(2))^2) + 80*qd(5)*(-c5*(-qd(3) + qd(4)) - s5*(-c3*s4*(qd(1) + qd(2)) + c4*s3*(qd(1) + qd(2)))) - s5*(c4*(+ c3*(c2*(- 270*qd(1)^2) - (qd(1) + qd(2))*(90*qd(1) + 90*qd(2)))) - s4*(- s3*(c2*(- 270*qd(1)^2) - (qd(1) + qd(2))*(90*qd(1) + 90*qd(2))))) + (80*c5*(-qd(3) + qd(4)) + 80*s5*(-c3*s4*(qd(1) + qd(2)) + c4*s3*(qd(1) + qd(2))))*(-c3*c4*(qd(1) + qd(2)) + qd(5) - s3*s4*(qd(1) + qd(2)))) + 80*qd(6)*(-c6*(-c5*(-qd(3) + qd(4)) - s5*(-c3*s4*(qd(1) + qd(2)) + c4*s3*(qd(1) + qd(2)))) - s6*(c5*(-c3*s4*(qd(1) + qd(2)) + c4*s3*(qd(1) + qd(2))) - s5*(-qd(3) + qd(4)))) - 80*s6*(- qd(5)*(c5*(-c3*s4*(qd(1) + qd(2)) + c4*s3*(qd(1) + qd(2))) - s5*(-qd(3) + qd(4))) - s5*(c4*(c3*qd(3)*(qd(1) + qd(2))) + qd(4)*(-c3*c4*(qd(1) + qd(2)) - s3*s4*(qd(1) + qd(2))) - s4*( - qd(3)*s3*(qd(1) + qd(2))))) - s6*(+ c5*(c4*(+ c3*(c2*(- 270*qd(1)^2) - (qd(1) + qd(2))*(90*qd(1) + 90*qd(2)))) - s4*(- s3*(c2*(- 270*qd(1)^2) - (qd(1) + qd(2))*(90*qd(1) + 90*qd(2))))) + 80*qd(5)*(c5*(-c3*s4*(qd(1) + qd(2)) + c4*s3*(qd(1) + qd(2))) - s5*(-qd(3) + qd(4))) + 80*s5*(c4*(c3*qd(3)*(qd(1) + qd(2))) + qd(4)*(-c3*c4*(qd(1) + qd(2)) - s3*s4*(qd(1) + qd(2))) - s4*(- qd(3)*s3*(qd(1) + qd(2)))) - 295*c3^2*(qd(1) + qd(2))^2 + s2*(- 270*qd(1)^2) - 295*s3^2*(qd(1) + qd(2))^2) - (80*c5*(-c3*s4*(qd(1) + qd(2)) + c4*s3*(qd(1) + qd(2))) - 80*s5*(-qd(3) + qd(4)))*(-c3*c4*(qd(1) + qd(2)) + qd(5) - s3*s4*(qd(1) + qd(2)))) + (80*c6*(-c5*(-qd(3) + qd(4)) - s5*(-c3*s4*(qd(1) + qd(2)) + c4*s3*(qd(1) + qd(2)))) + 80*s6*(c5*(-c3*s4*(qd(1) + qd(2)) + c4*s3*(qd(1) + qd(2))) - s5*(-qd(3) + qd(4))))*(c3*c4*(qd(1) + qd(2)) - qd(5) + qd(6) + s3*s4*(qd(1) + qd(2))) - 335*m3*(c2*(- 270*qd(1)^2) - (qd(1) + qd(2))*(270*qd(1) + 270*qd(2))) - s2*(- 270*qd(1)^2) + 270*m4*(90*c3*s3*(qd(1) + qd(2))^2 - s3*(c2*(- 270*qd(1)^2) - (qd(1) + qd(2))*(90*qd(1) + 90*qd(2)))) - 295*c3^2*(qd(1) + qd(2))^2 + s2*(- 270*qd(1)^2) - 295*s3^2*(qd(1) + qd(2))^2 - (-c3*c4*(qd(1) + qd(2)) - s3*s4*(qd(1) + qd(2)))*(295*c3*c4*(qd(1) + qd(2)) + 295*s3*s4*(qd(1) + qd(2))) + (-295*c3*s4*(qd(1) + qd(2)) + 295*c4*s3*(qd(1) + qd(2)))*(-c3*s4*(qd(1) + qd(2)) + c4*s3*(qd(1) + qd(2))) - 270*m6*(-c4*(- s3*(c2*(- 270*qd(1)^2) - (qd(1) + qd(2))*(90*qd(1) + 90*qd(2)))) - s4*(+ c3*(c2*(- 270*qd(1)^2) - (qd(1) + qd(2))*(90*qd(1) + 90*qd(2))))) + 270*m7*s5*(80*c6*(- qd(5)*(c5*(-c3*s4*(qd(1) + qd(2)) + c4*s3*(qd(1) + qd(2))) - s5*(-qd(3) + qd(4))) - s5*(c4*(c3*qd(3)*(qd(1) + qd(2))) + qd(4)*(-c3*c4*(qd(1) + qd(2)) - s3*s4*(qd(1) + qd(2))) - qd(3)*s3*(qd(1) + qd(2))))) + c6*(c5*(c4*(c3*(c2*(- 270*qd(1)^2) - (qd(1) + qd(2))*(90*qd(1) + 90*qd(2)))) - s4*(- s3*(c2*(- 270*qd(1)^2) - (qd(1) + qd(2))*(90*qd(1) + 90*qd(2))))) + 80*qd(5)*(c5*(-c3*s4*(qd(1) + qd(2)) + c4*s3*(qd(1) + qd(2))) - s5*(-qd(3) + qd(4))) + 80*s5*(c4*(c3*qd(3)*(qd(1) + qd(2))) + qd(4)*(-c3*c4*(qd(1) + qd(2)) - s3*s4*(qd(1) + qd(2))) - s4*( - qd(3)*s3*(qd(1) + qd(2)))) - s5*(- 295*c3^2*(qd(1) + qd(2))^2 + s2*(- 270*qd(1)^2) - 295*s3^2*(qd(1) + qd(2))^2) - (80*c5*(-c3*s4*(qd(1) + qd(2)) + c4*s3*(qd(1) + qd(2))) - 80*s5*(-qd(3) + qd(4)))*(-c3*c4*(qd(1) + qd(2)) + qd(5) - s3*s4*(qd(1) + qd(2)))) + 80*qd(6)*(c6*(c5*(-c3*s4*(qd(1) + qd(2)) + c4*s3*(qd(1) + qd(2))) - s5*(-qd(3) + qd(4))) - s6*(-c5*(-qd(3) + qd(4)) - s5*(-c3*s4*(qd(1) + qd(2)) + c4*s3*(qd(1) + qd(2))))) + 80*s6*(c5*(c4*(c3*qd(3)*(qd(1) + qd(2))) + qd(4)*(-c3*c4*(qd(1) + qd(2)) - s3*s4*(qd(1) + qd(2))) - s4*(- qd(3)*s3*(qd(1) + qd(2)))) + qd(5)*(-c5*(-qd(3) + qd(4)) - s5*(-c3*s4*(qd(1) + qd(2)) + c4*s3*(qd(1) + qd(2))))) - s6*(80*c5*(c4*(c3*qd(3)*(qd(1) + qd(2))) + qd(4)*(-c3*c4*(qd(1) + qd(2)) - s3*s4*(qd(1) + qd(2))) - s4*( - qd(3)*s3*(qd(1) + qd(2)))) - c5*( - 295*c3^2*(qd(1) + qd(2))^2 + s2*(- 270*qd(1)^2) - 295*s3^2*(qd(1) + qd(2))^2) + 80*qd(5)*(-c5*(-qd(3) + qd(4)) - s5*(-c3*s4*(qd(1) + qd(2)) + c4*s3*(qd(1) + qd(2)))) - s5*(c4*(c3*(c2*(- 270*qd(1)^2) - (qd(1) + qd(2))*(90*qd(1) + 90*qd(2)))) - s4*( - s3*(c2*(- 270*qd(1)^2) - (qd(1) + qd(2))*(90*qd(1) + 90*qd(2))))) + (80*c5*(-qd(3) + qd(4)) + 80*s5*(-c3*s4*(qd(1) + qd(2)) + c4*s3*(qd(1) + qd(2))))*(-c3*c4*(qd(1) + qd(2)) + qd(5) - s3*s4*(qd(1) + qd(2)))) - (80*c6*(c5*(-c3*s4*(qd(1) + qd(2)) + c4*s3*(qd(1) + qd(2))) - s5*(-qd(3) + qd(4))) - 80*s6*(-c5*(-qd(3) + qd(4)) - s5*(-c3*s4*(qd(1) + qd(2)) + c4*s3*(qd(1) + qd(2)))))*(c3*c4*(qd(1) + qd(2)) - qd(5) + qd(6) + s3*s4*(qd(1) + qd(2))) + 0.00744338*qd(3)*s3*(qd(1) + qd(2)) + 75*s2*(c3*(c4*(c5*m7*(80*c6*(- qd(5)*(c5*(-c3*s4*(qd(1) + qd(2)) + c4*s3*(qd(1) + qd(2))) - s5*(-qd(3) + qd(4))) - s5*(c4*(c3*qd(3)*(qd(1) + qd(2))) + qd(4)*(-c3*c4*(qd(1) + qd(2)) - s3*s4*(qd(1) + qd(2))) - s4*(- qd(3)*s3*(qd(1) + qd(2))))) + c6*(+ c5*(c4*(c3*(c2*(- 270*qd(1)^2) - (qd(1) + qd(2))*(90*qd(1) + 90*qd(2)))) - s3*(c2*(- 270*qd(1)^2) - (qd(1) + qd(2))*(90*qd(1) + 90*qd(2))))) + 80*qd(5)*(c5*(-c3*s4*(qd(1) + qd(2)) + c4*s3*(qd(1) + qd(2))) - s5*(-qd(3) + qd(4))) + 80*s5*(c4*(c3*qd(3)*(qd(1) + qd(2))) + qd(4)*(-c3*c4*(qd(1) + qd(2)) - s3*s4*(qd(1) + qd(2))) - s4*(- qd(3)*s3*(qd(1) + qd(2)))) - 295*c3^2*(qd(1) + qd(2))^2 + s2*(- 270*qd(1)^2) - 295*s3^2*(qd(1) + qd(2))^2) - (80*c5*(-c3*s4*(qd(1) + qd(2)) + c4*s3*(qd(1) + qd(2))) - 80*s5*(-qd(3) + qd(4)))*(-c3*c4*(qd(1) + qd(2)) + qd(5) - s3*s4*(qd(1) + qd(2)))) + 80*qd(6)*(c6*(c5*(-c3*s4*(qd(1) + qd(2)) + c4*s3*(qd(1) + qd(2))) - s5*(-qd(3) + qd(4))) - s6*(-c5*(-qd(3) + qd(4)) - s5*(-c3*s4*(qd(1) + qd(2)) + c4*s3*(qd(1) + qd(2))))) + 80*s6*(c5*(c4*(c3*qd(3)*(qd(1) + qd(2))) + qd(4)*(-c3*c4*(qd(1) + qd(2)) - s3*s4*(qd(1) + qd(2))) - s4*(- qd(3)*s3*(qd(1) + qd(2)))) + qd(5)*(-c5*(-qd(3) + qd(4)) - s5*(-c3*s4*(qd(1) + qd(2)) + c4*s3*(qd(1) + qd(2))))) - s6*(80*c5*(c4*(c3*qd(3)*(qd(1) + qd(2))) + qd(4)*(-c3*c4*(qd(1) + qd(2)) - s3*s4*(qd(1) + qd(2))) - s4*(- qd(3)*s3*(qd(1) + qd(2)))) - c5*(- 295*c3^2*(qd(1) + qd(2))^2 + s2*(- 270*qd(1)^2) - 295*s3^2*(qd(1) + qd(2))^2) + 80*qd(5)*(-c5*(-qd(3) + qd(4)) - s5*(-c3*s4*(qd(1) + qd(2)) + c4*s3*(qd(1) + qd(2)))) - s5*(c4*(+ c3*(c2*( - 270*qd(1)^2) - (qd(1) + qd(2))*(90*qd(1) + 90*qd(2)))) - s4*(- s3*(c2*(- 270*qd(1)^2) - (qd(1) + qd(2))*(90*qd(1) + 90*qd(2))))) + (80*c5*(-qd(3) + qd(4)) + 80*s5*(-c3*s4*(qd(1) + qd(2)) + c4*s3*(qd(1) + qd(2))))*(-c3*c4*(qd(1) + qd(2)) + qd(5) - s3*s4*(qd(1) + qd(2)))) - (80*c6*(c5*(-c3*s4*(qd(1) + qd(2)) + c4*s3*(qd(1) + qd(2))) - s5*(-qd(3) + qd(4))) - 80*s6*(-c5*(-qd(3) + qd(4)) - s5*(-c3*s4*(qd(1) + qd(2)) + c4*s3*(qd(1) + qd(2)))))*(c3*c4*(qd(1) + qd(2)) - qd(5) + qd(6) + s3*s4*(qd(1) + qd(2)))) + m6*(c5*(c4*(c3*(c2*(- 270*qd(1)^2) - (qd(1) + qd(2))*(90*qd(1) + 90*qd(2)))) - s4*(- s3*(c2*(- 270*qd(1)^2) - (qd(1) + qd(2))*(90*qd(1) + 90*qd(2))))) - s5*(- 295*c3^2*(qd(1) + qd(2))^2 + s2*(- 270*qd(1)^2) - 295*s3^2*(qd(1) + qd(2))^2)) - m7*s5*(80*c6*(c5*(c4*(c3*qd(3)*(qd(1) + qd(2))) + qd(4)*(-c3*c4*(qd(1) + qd(2)) - s3*s4*(qd(1) + qd(2))) - s4*(- qd(3)*s3*(qd(1) + qd(2)))) + qd(5)*(-c5*(-qd(3) + qd(4)) - s5*(-c3*s4*(qd(1) + qd(2)) + c4*s3*(qd(1) + qd(2)))))) - c6*(80*c5*(c4*(c3*qd(3)*(qd(1) + qd(2))) + qd(4)*(-c3*c4*(qd(1) + qd(2)) - s3*s4*(qd(1) + qd(2))) - s4*(- qd(3)*s3*(qd(1) + qd(2)))) - c5*(- 295*c3^2*(qd(1) + qd(2))^2 + s2*(- 270*qd(1)^2) - 295*s3^2*(qd(1) + qd(2))^2) + 80*qd(5)*(-c5*(-qd(3) + qd(4)) - s5*(-c3*s4*(qd(1) + qd(2)) + c4*s3*(qd(1) + qd(2)))) - s5*(c4*( c3*(c2*(- 270*qd(1)^2) - (qd(1) + qd(2))*(90*qd(1) + 90*qd(2)))) - s4*(- s3*(c2*(- 270*qd(1)^2) - (qd(1) + qd(2))*(90*qd(1) + 90*qd(2))))) + (80*c5*(-qd(3) + qd(4)) + 80*s5*(-c3*s4*(qd(1) + qd(2)) + c4*s3*(qd(1) + qd(2))))*(-c3*c4*(qd(1) + qd(2)) + qd(5) - s3*s4*(qd(1) + qd(2)))) + 80*qd(6)*(-c6*(-c5*(-qd(3) + qd(4)) - s5*(-c3*s4*(qd(1) + qd(2)) + c4*s3*(qd(1) + qd(2)))) - s6*(c5*(-c3*s4*(qd(1) + qd(2)) + c4*s3*(qd(1) + qd(2))) - s5*(-qd(3) + qd(4)))) - 80*s6*( - qd(5)*(c5*(-c3*s4*(qd(1) + qd(2)) + c4*s3*(qd(1) + qd(2))) - s5*(-qd(3) + qd(4))) - s5*(c4*(c3*qd(3)*(qd(1) + qd(2))) + qd(4)*(-c3*c4*(qd(1) + qd(2)) - s3*s4*(qd(1) + qd(2))) - s4*(- qd(3)*s3*(qd(1) + qd(2))))) - s6*( c5*(c4*( c3*(c2*(- 270*qd(1)^2) - (qd(1) + qd(2))*(90*qd(1) + 90*qd(2)))) - s4*(- s3*(c2*(- 270*qd(1)^2) - (qd(1) + qd(2))*(90*qd(1) + 90*qd(2))))) + 80*qd(5)*(c5*(-c3*s4*(qd(1) + qd(2)) + c4*s3*(qd(1) + qd(2))) - s5*(-qd(3) + qd(4))) + 80*s5*(c4*(c3*qd(3)*(qd(1) + qd(2))) + qd(4)*(-c3*c4*(qd(1) + qd(2)) - s3*s4*(qd(1) + qd(2))) - s4*(- qd(3)*s3*(qd(1) + qd(2)))) - s5*(- 295*c3^2*(qd(1) + qd(2))^2 + s2*(- 270*qd(1)^2) - 295*s3^2*(qd(1) + qd(2))^2) - (80*c5*(-c3*s4*(qd(1) + qd(2)) + c4*s3*(qd(1) + qd(2))) - 80*s5*(-qd(3) + qd(4)))*(-c3*c4*(qd(1) + qd(2)) + qd(5) - s3*s4*(qd(1) + qd(2)))) + (80*c6*(-c5*(-qd(3) + qd(4)) - s5*(-c3*s4*(qd(1) + qd(2)) + c4*s3*(qd(1) + qd(2)))) + 80*s6*(c5*(-c3*s4*(qd(1) + qd(2)) + c4*s3*(qd(1) + qd(2))) - s5*(-qd(3) + qd(4))))*(c3*c4*(qd(1) + qd(2)) - qd(5) + qd(6) + s3*s4*(qd(1) + qd(2)))) + m5*(c4*(c3*(c2*(- 270*qd(1)^2) - (qd(1) + qd(2))*(90*qd(1) + 90*qd(2)))) + 295*c4*(- qd(3)*s3*(qd(1) + qd(2))) + 295*qd(4)*(-c3*s4*(qd(1) + qd(2)) + c4*s3*(qd(1) + qd(2))) - s4*(- s3*(c2*(- 270*qd(1)^2) - (qd(1) + qd(2))*(90*qd(1) + 90*qd(2)))) + 295*s4*(c3*qd(3)*(qd(1) + qd(2)))) - (-qd(3) + qd(4))*(-295*c3*s4*(qd(1) + qd(2)) + 295*c4*s3*(qd(1) + qd(2))) - s4*(m6*(-c5*(- 295*c3^2*(qd(1) + qd(2))^2 + s2*( - 270*qd(1)^2) - 295*s3^2*(qd(1) + qd(2))^2) - s5*(c4*( c3*(c2*(- 270*qd(1)^2)  - (qd(1) + qd(2))*(90*qd(1) + 90*qd(2)))) - s4*(- s3*(c2*(- 270*qd(1)^2)  - (qd(1) + qd(2))*(90*qd(1) + 90*qd(2)))))) + m7*(c4*( - s3*(c2*(- 270*qd(1)^2) - (qd(1) + qd(2))*(90*qd(1) + 90*qd(2)))) + s4*(c3*(c2*(- 270*qd(1)^2) - (qd(1) + qd(2))*(90*qd(1) + 90*qd(2)))) + (-c5*(-qd(3) + qd(4)) - s5*(-c3*s4*(qd(1) + qd(2)) + c4*s3*(qd(1) + qd(2))))*(80*c5*(-qd(3) + qd(4)) + 80*s5*(-c3*s4*(qd(1) + qd(2)) + c4*s3*(qd(1) + qd(2)))) - (c5*(-c3*s4*(qd(1) + qd(2)) + c4*s3*(qd(1) + qd(2))) - s5*(-qd(3) + qd(4)))*(80*c5*(-c3*s4*(qd(1) + qd(2)) + c4*s3*(qd(1) + qd(2))) - 80*s5*(-qd(3) + qd(4))) - (-c6*(-c5*(-qd(3) + qd(4)) - s5*(-c3*s4*(qd(1) + qd(2)) + c4*s3*(qd(1) + qd(2)))) - s6*(c5*(-c3*s4*(qd(1) + qd(2)) + c4*s3*(qd(1) + qd(2))) - s5*(-qd(3) + qd(4))))*(80*c6*(-c5*(-qd(3) + qd(4)) - s5*(-c3*s4*(qd(1) + qd(2)) + c4*s3*(qd(1) + qd(2)))) + 80*s6*(c5*(-c3*s4*(qd(1) + qd(2)) + c4*s3*(qd(1) + qd(2))) - s5*(-qd(3) + qd(4)))) + (c6*(c5*(-c3*s4*(qd(1) + qd(2)) + c4*s3*(qd(1) + qd(2))) - s5*(-qd(3) + qd(4))) - s6*(-c5*(-qd(3) + qd(4)) - s5*(-c3*s4*(qd(1) + qd(2)) + c4*s3*(qd(1) + qd(2)))))*(80*c6*(c5*(-c3*s4*(qd(1) + qd(2)) + c4*s3*(qd(1) + qd(2))) - s5*(-qd(3) + qd(4))) - 80*s6*(-c5*(-qd(3) + qd(4)) - s5*(-c3*s4*(qd(1) + qd(2)) + c4*s3*(qd(1) + qd(2))))))) + m4*(-90*c3^2*(qd(1) + qd(2))^2 + c3*(c2*(- 270*qd(1)^2) - (qd(1) + qd(2))*(90*qd(1) + 90*qd(2))) - 90*qd(3)^2) - s3*(-c4*(m6*(-c5*( - 295*c3^2*(qd(1) + qd(2))^2 + s2*(- 270*qd(1)^2) - 295*s3^2*(qd(1) + qd(2))^2) - s5*(c4*(+ c3*(c2*( - 270*qd(1)^2) - (qd(1) + qd(2))*(90*qd(1) + 90*qd(2)))) - s4*(2- s3*(c2*(- 270*qd(1)^2) - (qd(1) + qd(2))*(90*qd(1) + 90*qd(2)))))) + m7*(c4*(- s3*(c2*(- 270*qd(1)^2) - (qd(1) + qd(2))*(90*qd(1) + 90*qd(2)))) + s4*(c3*(c2*(- 270*qd(1)^2) - (qd(1) + qd(2))*(90*qd(1) + 90*qd(2)))) + (-c5*(-qd(3) + qd(4)) - s5*(-c3*s4*(qd(1) + qd(2)) + c4*s3*(qd(1) + qd(2))))*(80*c5*(-qd(3) + qd(4)) + 80*s5*(-c3*s4*(qd(1) + qd(2)) + c4*s3*(qd(1) + qd(2)))) - (c5*(-c3*s4*(qd(1) + qd(2)) + c4*s3*(qd(1) + qd(2))) - s5*(-qd(3) + qd(4)))*(80*c5*(-c3*s4*(qd(1) + qd(2)) + c4*s3*(qd(1) + qd(2))) - 80*s5*(-qd(3) + qd(4))) - (-c6*(-c5*(-qd(3) + qd(4)) - s5*(-c3*s4*(qd(1) + qd(2)) + c4*s3*(qd(1) + qd(2)))) - s6*(c5*(-c3*s4*(qd(1) + qd(2)) + c4*s3*(qd(1) + qd(2))) - s5*(-qd(3) + qd(4))))*(80*c6*(-c5*(-qd(3) + qd(4)) - s5*(-c3*s4*(qd(1) + qd(2)) + c4*s3*(qd(1) + qd(2)))) + 80*s6*(c5*(-c3*s4*(qd(1) + qd(2)) + c4*s3*(qd(1) + qd(2))) - s5*(-qd(3) + qd(4)))) + (c6*(c5*(-c3*s4*(qd(1) + qd(2)) + c4*s3*(qd(1) + qd(2))) - s5*(-qd(3) + qd(4))) - s6*(-c5*(-qd(3) + qd(4)) - s5*(-c3*s4*(qd(1) + qd(2)) + c4*s3*(qd(1) + qd(2)))))*(80*c6*(c5*(-c3*s4*(qd(1) + qd(2)) + c4*s3*(qd(1) + qd(2))) - s5*(-qd(3) + qd(4))) - 80*s6*(-c5*(-qd(3) + qd(4)) - s5*(-c3*s4*(qd(1) + qd(2)) + c4*s3*(qd(1) + qd(2))))))) + m5*(-c4*( - s3*(c2*(- 270*qd(1)^2) - (qd(1) + qd(2))*(90*qd(1) + 90*qd(2)))) + 295*c4*(c3*qd(3)*(qd(1) + qd(2))) + 295*qd(4)*(-c3*c4*(qd(1) + qd(2)) - s3*s4*(qd(1) + qd(2))) - s4*( c3*(c2*( - 270*qd(1)^2) - (qd(1) + qd(2))*(90*qd(1) + 90*qd(2)))) - 295*s4*(- qd(3)*s3*(qd(1) + qd(2))) + (-qd(3) + qd(4))*(295*c3*c4*(qd(1) + qd(2)) + 295*s3*s4*(qd(1) + qd(2)))) - s4*(c5*m7*(80*c6*(- qd(5)*(c5*(-c3*s4*(qd(1) + qd(2)) + c4*s3*(qd(1) + qd(2))) - s5*(-qd(3) + qd(4))) - s5*(c4*(c3*qd(3)*(qd(1) + qd(2))) + qd(4)*(-c3*c4*(qd(1) + qd(2)) - s3*s4*(qd(1) + qd(2))) - s4*(- qd(3)*s3*(qd(1) + qd(2))))) + c6*(c5*(c4*(c3*(c2*(- 270*qd(1)^2) - (qd(1) + qd(2))*(90*qd(1) + 90*qd(2)))) - s4*(- s3*(c2*(- 270*qd(1)^2) - (qd(1) + qd(2))*(90*qd(1) + 90*qd(2))))) + 80*qd(5)*(c5*(-c3*s4*(qd(1) + qd(2)) + c4*s3*(qd(1) + qd(2))) - s5*(-qd(3) + qd(4))) + 80*s5*(c4*(c3*qd(3)*(qd(1) + qd(2))) + qd(4)*(-c3*c4*(qd(1) + qd(2)) - s3*s4*(qd(1) + qd(2))) - s4*( - qd(3)*s3*(qd(1) + qd(2)))) - s5*(- 295*c3^2*(qd(1) + qd(2))^2 + s2*(- 270*qd(1)^2) - 295*s3^2*(qd(1) + qd(2))^2) - (80*c5*(-c3*s4*(qd(1) + qd(2)) + c4*s3*(qd(1) + qd(2))) - 80*s5*(-qd(3) + qd(4)))*(-c3*c4*(qd(1) + qd(2)) + qd(5) - s3*s4*(qd(1) + qd(2)))) + 80*qd(6)*(c6*(c5*(-c3*s4*(qd(1) + qd(2)) + c4*s3*(qd(1) + qd(2))) - s5*(-qd(3) + qd(4))) - s6*(-c5*(-qd(3) + qd(4)) - s5*(-c3*s4*(qd(1) + qd(2)) + c4*s3*(qd(1) + qd(2))))) + 80*s6*(c5*(c4*(c3*qd(3)*(qd(1) + qd(2))) + qd(4)*(-c3*c4*(qd(1) + qd(2)) - s3*s4*(qd(1) + qd(2))) - s4*( - qd(3)*s3*(qd(1) + qd(2)))) + qd(5)*(-c5*(-qd(3) + qd(4)) - s5*(-c3*s4*(qd(1) + qd(2)) + c4*s3*(qd(1) + qd(2)))) ) - s6*(80*c5*(c4*(c3*qd(3)*(qd(1) + qd(2))) + qd(4)*(-c3*c4*(qd(1) + qd(2)) - s3*s4*(qd(1) + qd(2))) - s4*(- qd(3)*s3*(qd(1) + qd(2)))) - c5*(- 295*c3^2*(qd(1) + qd(2))^2 + s2*(- 270*qd(1)^2) - 295*s3^2*(qd(1) + qd(2))^2) + 80*qd(5)*(-c5*(-qd(3) + qd(4)) - s5*(-c3*s4*(qd(1) + qd(2)) + c4*s3*(qd(1) + qd(2)))) - s5*(c4*(+ c3*(c2*(- 270*qd(1)^2) - (qd(1) + qd(2))*(90*qd(1) + 90*qd(2)))) - s4*(- s3*(c2*(- 270*qd(1)^2) - (qd(1) + qd(2))*(90*qd(1) + 90*qd(2))))) + (80*c5*(-qd(3) + qd(4)) + 80*s5*(-c3*s4*(qd(1) + qd(2)) + c4*s3*(qd(1) + qd(2))))*(-c3*c4*(qd(1) + qd(2)) + qd(5) - s3*s4*(qd(1) + qd(2)))) - (80*c6*(c5*(-c3*s4*(qd(1) + qd(2)) + c4*s3*(qd(1) + qd(2))) - s5*(-qd(3) + qd(4))) - 80*s6*(-c5*(-qd(3) + qd(4)) - s5*(-c3*s4*(qd(1) + qd(2)) + c4*s3*(qd(1) + qd(2)))))*(c3*c4*(qd(1) + qd(2)) - qd(5) + qd(6) + s3*s4*(qd(1) + qd(2)))) + m6*(c5*(c4*(c3*(c2*(- 270*qd(1)^2) - (qd(1) + qd(2))*(90*qd(1) + 90*qd(2)))) - s4*( - s3*(c2*(- 270*qd(1)^2) - (qd(1) + qd(2))*(90*qd(1) + 90*qd(2))))) - s5*( - 295*c3^2*(qd(1) + qd(2))^2 + s2*(- 270*qd(1)^2) - 295*s3^2*(qd(1) + qd(2))^2)) - m7*s5*(80*c6*(c5*(c4*(c3*qd(3)*(qd(1) + qd(2))) + qd(4)*(-c3*c4*(qd(1) + qd(2)) - s3*s4*(qd(1) + qd(2))) - s4*(- qd(3)*s3*(qd(1) + qd(2)))) + qd(5)*(-c5*(-qd(3) + qd(4)) - s5*(-c3*s4*(qd(1) + qd(2)) + c4*s3*(qd(1) + qd(2))))) - c6*(80*c5*(c4*(c3*qd(3)*(qd(1) + qd(2))) + qd(4)*(-c3*c4*(qd(1) + qd(2)) - s3*s4*(qd(1) + qd(2))) - s4*(- qd(3)*s3*(qd(1) + qd(2)))) - c5*(- 295*c3^2*(qd(1) + qd(2))^2 + s2*(- 270*qd(1)^2) - 295*s3^2*(qd(1) + qd(2))^2) + 80*qd(5)*(-c5*(-qd(3) + qd(4)) - s5*(-c3*s4*(qd(1) + qd(2)) + c4*s3*(qd(1) + qd(2)))) - s5*(c4*(c3*(c2*(- 270*qd(1)^2) - (qd(1) + qd(2))*(90*qd(1) + 90*qd(2)))) - s4*(- s3*(c2*(- 270*qd(1)^2) - (qd(1) + qd(2))*(90*qd(1) + 90*qd(2))))) + (80*c5*(-qd(3) + qd(4)) + 80*s5*(-c3*s4*(qd(1) + qd(2)) + c4*s3*(qd(1) + qd(2))))*(-c3*c4*(qd(1) + qd(2)) + qd(5) - s3*s4*(qd(1) + qd(2)))) + 80*qd(6)*(-c6*(-c5*(-qd(3) + qd(4)) - s5*(-c3*s4*(qd(1) + qd(2)) + c4*s3*(qd(1) + qd(2)))) - s6*(c5*(-c3*s4*(qd(1) + qd(2)) + c4*s3*(qd(1) + qd(2))) - s5*(-qd(3) + qd(4)))) - 80*s6*(- qd(5)*(c5*(-c3*s4*(qd(1) + qd(2)) + c4*s3*(qd(1) + qd(2))) - s5*(-qd(3) + qd(4))) - s5*(c4*(c3*qd(3)*(qd(1) + qd(2))) + qd(4)*(-c3*c4*(qd(1) + qd(2)) - s3*s4*(qd(1) + qd(2))) - s4*(- qd(3)*s3*(qd(1) + qd(2))))) - s6*(c5*(c4*( c3*(c2*(- 270*qd(1)^2) - (qd(1) + qd(2))*(90*qd(1) + 90*qd(2)))) - s4*(- s3*(c2*(- 270*qd(1)^2) - (qd(1) + qd(2))*(90*qd(1) + 90*qd(2))))) + 80*qd(5)*(c5*(-c3*s4*(qd(1) + qd(2)) + c4*s3*(qd(1) + qd(2))) - s5*(-qd(3) + qd(4))) + 80*s5*(c4*(c3*qd(3)*(qd(1) + qd(2))) + qd(4)*(-c3*c4*(qd(1) + qd(2)) - s3*s4*(qd(1) + qd(2))) - s4*( - qd(3)*s3*(qd(1) + qd(2)))) - s5*( - 295*c3^2*(qd(1) + qd(2))^2  + s2*(- 270*qd(1)^2) - 295*s3^2*(qd(1) + qd(2))^2) - (80*c5*(-c3*s4*(qd(1) + qd(2)) + c4*s3*(qd(1) + qd(2))) - 80*s5*(-qd(3) + qd(4)))*(-c3*c4*(qd(1) + qd(2)) + qd(5) - s3*s4*(qd(1) + qd(2)))) + (80*c6*(-c5*(-qd(3) + qd(4)) - s5*(-c3*s4*(qd(1) + qd(2)) + c4*s3*(qd(1) + qd(2)))) + 80*s6*(c5*(-c3*s4*(qd(1) + qd(2)) + c4*s3*(qd(1) + qd(2))) - s5*(-qd(3) + qd(4))))*(c3*c4*(qd(1) + qd(2)) - qd(5) + qd(6) + s3*s4*(qd(1) + qd(2)))))) + 335*s2*(c5*m7*(80*c6*(c5*(c4*(c3*qd(3)*(qd(1) + qd(2))) + qd(4)*(-c3*c4*(qd(1) + qd(2)) - s3*s4*(qd(1) + qd(2))) - s4*(- qd(3)*s3*(qd(1) + qd(2)))) + qd(5)*(-c5*(-qd(3) + qd(4)) - s5*(-c3*s4*(qd(1) + qd(2)) + c4*s3*(qd(1) + qd(2))))) - c6*(80*c5*(c4*(c3*qd(3)*(qd(1) + qd(2))) + qd(4)*(-c3*c4*(qd(1) + qd(2)) - s3*s4*(qd(1) + qd(2))) - s4*( - qd(3)*s3*(qd(1) + qd(2)))) - c5*(- 295*c3^2*(qd(1) + qd(2))^2 + s2*(- 270*qd(1)^2) - 295*s3^2*(qd(1) + qd(2))^2) + 80*qd(5)*(-c5*(-qd(3) + qd(4)) - s5*(-c3*s4*(qd(1) + qd(2)) + c4*s3*(qd(1) + qd(2)))) - s5*(c4*(+ c3*(c2*( - 270*qd(1)^2) - (qd(1) + qd(2))*(90*qd(1) + 90*qd(2)))) - s4*(- s3*(c2*(- 270*qd(1)^2) - (qd(1) + qd(2))*(90*qd(1) + 90*qd(2))))) + (80*c5*(-qd(3) + qd(4)) + 80*s5*(-c3*s4*(qd(1) + qd(2)) + c4*s3*(qd(1) + qd(2))))*(-c3*c4*(qd(1) + qd(2)) + qd(5) - s3*s4*(qd(1) + qd(2)))) + 80*qd(6)*(-c6*(-c5*(-qd(3) + qd(4)) - s5*(-c3*s4*(qd(1) + qd(2)) + c4*s3*(qd(1) + qd(2)))) - s6*(c5*(-c3*s4*(qd(1) + qd(2)) + c4*s3*(qd(1) + qd(2))) - s5*(-qd(3) + qd(4)))) - 80*s6*(- qd(5)*(c5*(-c3*s4*(qd(1) + qd(2)) + c4*s3*(qd(1) + qd(2))) - s5*(-qd(3) + qd(4))) - s5*(c4*(c3*qd(3)*(qd(1) + qd(2))) + qd(4)*(-c3*c4*(qd(1) + qd(2)) - s3*s4*(qd(1) + qd(2))) - s4*(- qd(3)*s3*(qd(1) + qd(2))))) - s6*(+ c5*(c4*(+ c3*(c2*(- 270*qd(1)^2)  - (qd(1) + qd(2))*(90*qd(1) + 90*qd(2)))) - s4*(- s3*(c2*(- 270*qd(1)^2) - (qd(1) + qd(2))*(90*qd(1) + 90*qd(2))))) + 80*qd(5)*(c5*(-c3*s4*(qd(1) + qd(2)) + c4*s3*(qd(1) + qd(2))) - s5*(-qd(3) + qd(4))) + 80*s5*(c4*(c3*qd(3)*(qd(1) + qd(2)))) + qd(4)*(-c3*c4*(qd(1) + qd(2)) - s3*s4*(qd(1) + qd(2))) - s4*(- qd(3)*s3*(qd(1) + qd(2)))) - s5*(- 295*c3^2*(qd(1) + qd(2))^2 + s2*(- 270*qd(1)^2) - 295*s3^2*(qd(1) + qd(2))^2) - (80*c5*(-c3*s4*(qd(1) + qd(2)) + c4*s3*(qd(1) + qd(2))) - 80*s5*(-qd(3) + qd(4)))*(-c3*c4*(qd(1) + qd(2)) + qd(5) - s3*s4*(qd(1) + qd(2)))) + (80*c6*(-c5*(-qd(3) + qd(4)) - s5*(-c3*s4*(qd(1) + qd(2)) + c4*s3*(qd(1) + qd(2)))) + 80*s6*(c5*(-c3*s4*(qd(1) + qd(2)) + c4*s3*(qd(1) + qd(2))) - s5*(-qd(3) + qd(4))))*(c3*c4*(qd(1) + qd(2)) - qd(5) + qd(6) + s3*s4*(qd(1) + qd(2)))) + m4*(90*c3*s3*(qd(1) + qd(2))^2 - s3*(c2*(- 270*qd(1)^2) - (qd(1) + qd(2))*(90*qd(1) + 90*qd(2)))) + m5*(- 295*c3^2*(qd(1) + qd(2))^2 + s2*(- 270*qd(1)^2) - 295*s3^2*(qd(1) + qd(2))^2 - (-c3*c4*(qd(1) + qd(2)) - s3*s4*(qd(1) + qd(2)))*(295*c3*c4*(qd(1) + qd(2)) + 295*s3*s4*(qd(1) + qd(2))) + (-295*c3*s4*(qd(1) + qd(2)) + 295*c4*s3*(qd(1) + qd(2)))*(-c3*s4*(qd(1) + qd(2)) + c4*s3*(qd(1) + qd(2)))) - m6*(-c4*(- s3*(c2*(- 270*qd(1)^2) - (qd(1) + qd(2))*(90*qd(1) + 90*qd(2)))) - s4*(c3*(c2*(- 270*qd(1)^2) - (qd(1) + qd(2))*(90*qd(1) + 90*qd(2))))) + m7*s5*(80*c6*(- qd(5)*(c5*(-c3*s4*(qd(1) + qd(2)) + c4*s3*(qd(1) + qd(2))) - s5*(-qd(3) + qd(4))) - s5*(c4*(c3*qd(3)*(qd(1) + qd(2))) + qd(4)*(-c3*c4*(qd(1) + qd(2)) - s3*s4*(qd(1) + qd(2))) - s4*(- qd(3)*s3*(qd(1) + qd(2))))) + c6*( + c5*(c4*(+ c3*(c2*(- 270*qd(1)^2) - (qd(1) + qd(2))*(90*qd(1) + 90*qd(2)))) - s4*( - s3*(c2*(- 270*qd(1)^2) - (qd(1) + qd(2))*(90*qd(1) + 90*qd(2))))) + 80*qd(5)*(c5*(-c3*s4*(qd(1) + qd(2)) + c4*s3*(qd(1) + qd(2))) - s5*(-qd(3) + qd(4))) + 80*s5*(c4*(c3*qd(3)*(qd(1) + qd(2))) + qd(4)*(-c3*c4*(qd(1) + qd(2)) - s3*s4*(qd(1) + qd(2))) - s4*(- qd(3)*s3*(qd(1) + qd(2)))) - s5*(- 295*c3^2*(qd(1) + qd(2))^2 + s2*(- 270*qd(1)^2) - 295*s3^2*(qd(1) + qd(2))^2) - (80*c5*(-c3*s4*(qd(1) + qd(2)) + c4*s3*(qd(1) + qd(2))) - 80*s5*(-qd(3) + qd(4)))*(-c3*c4*(qd(1) + qd(2)) + qd(5) - s3*s4*(qd(1) + qd(2)))) + 80*qd(6)*(c6*(c5*(-c3*s4*(qd(1) + qd(2)) + c4*s3*(qd(1) + qd(2))) - s5*(-qd(3) + qd(4))) - s6*(-c5*(-qd(3) + qd(4)) - s5*(-c3*s4*(qd(1) + qd(2)) + c4*s3*(qd(1) + qd(2))))) + 80*s6*(c5*(c4*(c3*qd(3)*(qd(1) + qd(2))) + qd(4)*(-c3*c4*(qd(1) + qd(2)) - s3*s4*(qd(1) + qd(2))) - s4*( - qd(3)*s3*(qd(1) + qd(2)))) + qd(5)*(-c5*(-qd(3) + qd(4)) - s5*(-c3*s4*(qd(1) + qd(2)) + c4*s3*(qd(1) + qd(2))))) - s6*(80*c5*(c4*(c3*qd(3)*(qd(1) + qd(2)))) + qd(4)*(-c3*c4*(qd(1) + qd(2)) - s3*s4*(qd(1) + qd(2))) - s4*(- qd(3)*s3*(qd(1) + qd(2)))) - c5*(-c2*(- 295*c3^2*(qd(1) + qd(2))^2 + s2*(- 270*qd(1)^2) - 295*s3^2*(qd(1) + qd(2))^2) + 80*qd(5)*(-c5*(-qd(3) + qd(4)) - s5*(-c3*s4*(qd(1) + qd(2)) + c4*s3*(qd(1) + qd(2)))) - s5*(c4*(c3*(c2*(- 270*qd(1)^2) - (qd(1) + qd(2))*(90*qd(1) + 90*qd(2)))) - s4*( - s3*(c2*(- 270*qd(1)^2) - (qd(1) + qd(2))*(90*qd(1) + 90*qd(2))))) + (80*c5*(-qd(3) + qd(4)) + 80*s5*(-c3*s4*(qd(1) + qd(2)) + c4*s3*(qd(1) + qd(2))))*(-c3*c4*(qd(1) + qd(2)) + qd(5) - s3*s4*(qd(1) + qd(2)))) - (80*c6*(c5*(-c3*s4*(qd(1) + qd(2)) + c4*s3*(qd(1) + qd(2))) - s5*(-qd(3) + qd(4))) - 80*s6*(-c5*(-qd(3) + qd(4)) - s5*(-c3*s4*(qd(1) + qd(2)) + c4*s3*(qd(1) + qd(2)))))*(c3*c4*(qd(1) + qd(2)) - qd(5) + qd(6) + s3*s4*(qd(1) + qd(2)))) + s3*(qd(1) + qd(2))*(0.750399*c3*(qd(1) + qd(2)) - 0.00744338*qd(3) - 0.00947011*s3*(qd(1) + qd(2))) + s3*(0.00163355*c4*(- qd(3)*s3*(qd(1) + qd(2))) + 0.00950111*c4*(c3*qd(3)*(qd(1) + qd(2))) + c4*(+ 0.00151607*c5*(c4*(c3*qd(3)*(qd(1) + qd(2))) + qd(4)*(-c3*c4*(qd(1) + qd(2)) - s3*s4*(qd(1) + qd(2))) - s4*(- qd(3)*s3*(qd(1) + qd(2)))) + c5*(6.20477e-6*c6*(c5*(c4*(c3*qd(3)*(qd(1) + qd(2))) + qd(4)*(-c3*c4*(qd(1) + qd(2)) - s3*s4*(qd(1) + qd(2))) - s4*(- qd(3)*s3*(qd(1) + qd(2)))) + qd(5)*(-c5*(-qd(3) + qd(4)) - s5*(-c3*s4*(qd(1) + qd(2)) + c4*s3*(qd(1) + qd(2)))) ) + 6.20477e-6*qd(6)*(-c6*(-c5*(-qd(3) + qd(4)) - s5*(-c3*s4*(qd(1) + qd(2)) + c4*s3*(qd(1) + qd(2)))) - s6*(c5*(-c3*s4*(qd(1) + qd(2)) + c4*s3*(qd(1) + qd(2))) - s5*(-qd(3) + qd(4)))) - 6.20477e-6*s6*( - qd(5)*(c5*(-c3*s4*(qd(1) + qd(2)) + c4*s3*(qd(1) + qd(2))) - s5*(-qd(3) + qd(4))) - s5*(c4*(c3*qd(3)*(qd(1) + qd(2)) ) + qd(4)*(-c3*c4*(qd(1) + qd(2)) - s3*s4*(qd(1) + qd(2))) - s4*(- qd(3)*s3*(qd(1) + qd(2))))) + (-c6*(-c5*(-qd(3) + qd(4)) - s5*(-c3*s4*(qd(1) + qd(2)) + c4*s3*(qd(1) + qd(2)))) - s6*(c5*(-c3*s4*(qd(1) + qd(2)) + c4*s3*(qd(1) + qd(2))) - s5*(-qd(3) + qd(4))))*(3.29301e-6*c3*c4*(qd(1) + qd(2)) - 3.29301e-6*qd(5) + 3.29301e-6*qd(6) + 3.29301e-6*s3*s4*(qd(1) + qd(2))) - (-3.01352e-6*c6*(-c5*(-qd(3) + qd(4)) - s5*(-c3*s4*(qd(1) + qd(2)) + c4*s3*(qd(1) + qd(2)))) - 3.01352e-6*s6*(c5*(-c3*s4*(qd(1) + qd(2)) + c4*s3*(qd(1) + qd(2))) - s5*(-qd(3) + qd(4))))*(c3*c4*(qd(1) + qd(2)) - qd(5) + qd(6) + s3*s4*(qd(1) + qd(2)))) + 295*m6*(-c5*( - 295*c3^2*(qd(1) + qd(2))^2 + s2*( - 270*qd(1)^2) - 295*s3^2*(qd(1) + qd(2))^2) - s5*(+ c3*(c2*(- 270*qd(1)^2) - (qd(1) + qd(2))*(90*qd(1) + 90*qd(2)))) - s4*(- s3*(c2*(- 270*qd(1)^2) - (qd(1) + qd(2))*(90*qd(1) + 90*qd(2)))))) + 295*m7*(c4*(- s3*(c2*(- 270*qd(1)^2) - (qd(1) + qd(2))*(90*qd(1) + 90*qd(2)))) + s4*(+ c3*(c2*(- 270*qd(1)^2) - (qd(1) + qd(2))*(90*qd(1) + 90*qd(2)))) + (-c5*(-qd(3) + qd(4)) - s5*(-c3*s4*(qd(1) + qd(2)) + c4*s3*(qd(1) + qd(2))))*(80*c5*(-qd(3) + qd(4)) + 80*s5*(-c3*s4*(qd(1) + qd(2)) + c4*s3*(qd(1) + qd(2)))) - (c5*(-c3*s4*(qd(1) + qd(2)) + c4*s3*(qd(1) + qd(2))) - s5*(-qd(3) + qd(4)))*(80*c5*(-c3*s4*(qd(1) + qd(2)) + c4*s3*(qd(1) + qd(2))) - 80*s5*(-qd(3) + qd(4))) - (-c6*(-c5*(-qd(3) + qd(4)) - s5*(-c3*s4*(qd(1) + qd(2)) + c4*s3*(qd(1) + qd(2)))) - s6*(c5*(-c3*s4*(qd(1) + qd(2)) + c4*s3*(qd(1) + qd(2))) - s5*(-qd(3) + qd(4))))*(80*c6*(-c5*(-qd(3) + qd(4)) - s5*(-c3*s4*(qd(1) + qd(2)) + c4*s3*(qd(1) + qd(2)))) + 80*s6*(c5*(-c3*s4*(qd(1) + qd(2)) + c4*s3*(qd(1) + qd(2))) - s5*(-qd(3) + qd(4)))) + (c6*(c5*(-c3*s4*(qd(1) + qd(2)) + c4*s3*(qd(1) + qd(2))) - s5*(-qd(3) + qd(4))) - s6*(-c5*(-qd(3) + qd(4)) - s5*(-c3*s4*(qd(1) + qd(2)) + c4*s3*(qd(1) + qd(2)))))*(80*c6*(c5*(-c3*s4*(qd(1) + qd(2)) + c4*s3*(qd(1) + qd(2))) - s5*(-qd(3) + qd(4))) - 80*s6*(-c5*(-qd(3) + qd(4)) - s5*(-c3*s4*(qd(1) + qd(2)) + c4*s3*(qd(1) + qd(2)))))) + 0.00151607*qd(5)*(-c5*(-qd(3) + qd(4)) - s5*(-c3*s4*(qd(1) + qd(2)) + c4*s3*(qd(1) + qd(2)))) + 0.000409305*qd(5)*(c5*(-c3*s4*(qd(1) + qd(2)) + c4*s3*(qd(1) + qd(2))) - s5*(-qd(3) + qd(4))) + 0.000409305*s5*(c4*(c3*qd(3)*(qd(1) + qd(2))) + qd(4)*(-c3*c4*(qd(1) + qd(2)) - s3*s4*(qd(1) + qd(2))) - s4*(- qd(3)*s3*(qd(1) + qd(2)))) - s5*(-3.01352e-6*c6*( - qd(5)*(c5*(-c3*s4*(qd(1) + qd(2)) + c4*s3*(qd(1) + qd(2))) - s5*(-qd(3) + qd(4))) - s5*(c4*(c3*qd(3)*(qd(1) + qd(2))) + qd(4)*(-c3*c4*(qd(1) + qd(2)) - s3*s4*(qd(1) + qd(2))) - s4*(- qd(3)*s3*(qd(1) + qd(2))))) - 3.01352e-6*qd(6)*(c6*(c5*(-c3*s4*(qd(1) + qd(2)) + c4*s3*(qd(1) + qd(2))) - s5*(-qd(3) + qd(4))) - s6*(-c5*(-qd(3) + qd(4)) - s5*(-c3*s4*(qd(1) + qd(2)) + c4*s3*(qd(1) + qd(2))))) - 3.01352e-6*s6*(c5*(c4*(c3*qd(3)*(qd(1) + qd(2))) + qd(4)*(-c3*c4*(qd(1) + qd(2)) - s3*s4*(qd(1) + qd(2))) - s4*(- qd(3)*s3*(qd(1) + qd(2)))) + qd(5)*(-c5*(-qd(3) + qd(4)) - s5*(-c3*s4*(qd(1) + qd(2)) + c4*s3*(qd(1) + qd(2))))) + (6.20477e-6*c6*(c5*(-c3*s4*(qd(1) + qd(2)) + c4*s3*(qd(1) + qd(2))) - s5*(-qd(3) + qd(4))) - 6.20477e-6*s6*(-c5*(-qd(3) + qd(4)) - s5*(-c3*s4*(qd(1) + qd(2)) + c4*s3*(qd(1) + qd(2)))))*(c3*c4*(qd(1) + qd(2)) - qd(5) + qd(6) + s3*s4*(qd(1) + qd(2))) - (c6*(c5*(-c3*s4*(qd(1) + qd(2)) + c4*s3*(qd(1) + qd(2))) - s5*(-qd(3) + qd(4))) - s6*(-c5*(-qd(3) + qd(4)) - s5*(-c3*s4*(qd(1) + qd(2)) + c4*s3*(qd(1) + qd(2)))))*(3.29301e-6*c3*c4*(qd(1) + qd(2)) - 3.29301e-6*qd(5) + 3.29301e-6*qd(6) + 3.29301e-6*s3*s4*(qd(1) + qd(2)))) + (-c5*(-qd(3) + qd(4)) - s5*(-c3*s4*(qd(1) + qd(2)) + c4*s3*(qd(1) + qd(2))))*(-0.00358942*c3*c4*(qd(1) + qd(2)) + 0.00358942*qd(5) - 0.00358942*s3*s4*(qd(1) + qd(2))) - (-c3*c4*(qd(1) + qd(2)) + qd(5) - s3*s4*(qd(1) + qd(2)))*(-0.00355535*c5*(-qd(3) + qd(4)) - 0.000409305*c5*(-c3*s4*(qd(1) + qd(2)) + c4*s3*(qd(1) + qd(2))) + 0.000409305*s5*(-qd(3) + qd(4)) - 0.00355535*s5*(-c3*s4*(qd(1) + qd(2)) + c4*s3*(qd(1) + qd(2))))) + 0.00950111*qd(4)*(-c3*c4*(qd(1) + qd(2)) - s3*s4*(qd(1) + qd(2))) + 0.00163355*qd(4)*(-c3*s4*(qd(1) + qd(2)) + c4*s3*(qd(1) + qd(2))) - 0.00950111*s4*(- qd(3)*s3*(qd(1) + qd(2))) + 0.00163355*s4*(c3*qd(3)*(qd(1) + qd(2))) - s4*(3.29301e-6*c4*( - qd(3)*s3*(qd(1) + qd(2))) - 295*c5*m7*(80*c6*(- qd(5)*(c5*(-c3*s4*(qd(1) + qd(2)) + c4*s3*(qd(1) + qd(2))) - s5*(-qd(3) + qd(4))) - s5*(c4*(c3*qd(3)*(qd(1) + qd(2))) + qd(4)*(-c3*c4*(qd(1) + qd(2)) - s3*s4*(qd(1) + qd(2))) - s4*(- qd(3)*s3*(qd(1) + qd(2))))) + c6*(c5*(c4*( c3*(c2*(- 270*qd(1)^2) - (qd(1) + qd(2))*(90*qd(1) + 90*qd(2)))) - s4*(- s3*(c2*(- 270*qd(1)^2) - (qd(1) + qd(2))*(90*qd(1) + 90*qd(2))))) + 80*qd(5)*(c5*(-c3*s4*(qd(1) + qd(2)) + c4*s3*(qd(1) + qd(2))) - s5*(-qd(3) + qd(4))) + 80*s5*(c4*(c3*qd(3)*(qd(1) + qd(2))) + qd(4)*(-c3*c4*(qd(1) + qd(2)) - s3*s4*(qd(1) + qd(2))) - s4*(- qd(3)*s3*(qd(1) + qd(2)))) - s5*( - 295*c3^2*(qd(1) + qd(2))^2 + s2*(- 270*qd(1)^2) - 295*s3^2*(qd(1) + qd(2))^2) - (80*c5*(-c3*s4*(qd(1) + qd(2)) + c4*s3*(qd(1) + qd(2))) - 80*s5*(-qd(3) + qd(4)))*(-c3*c4*(qd(1) + qd(2)) + qd(5) - s3*s4*(qd(1) + qd(2)))) + 80*qd(6)*(c6*(c5*(-c3*s4*(qd(1) + qd(2)) + c4*s3*(qd(1) + qd(2))) - s5*(-qd(3) + qd(4))) - s6*(-c5*(-qd(3) + qd(4)) - s5*(-c3*s4*(qd(1) + qd(2)) + c4*s3*(qd(1) + qd(2))))) + 80*s6*(c5*(c4*(c3*qd(3)*(qd(1) + qd(2))) + qd(4)*(-c3*c4*(qd(1) + qd(2)) - s3*s4*(qd(1) + qd(2))) - s4*(- qd(3)*s3*(qd(1) + qd(2)))) + qd(5)*(-c5*(-qd(3) + qd(4)) - s5*(-c3*s4*(qd(1) + qd(2)) + c4*s3*(qd(1) + qd(2)))) ) - s6*(80*c5*(c4*(c3*qd(3)*(qd(1) + qd(2))) + qd(4)*(-c3*c4*(qd(1) + qd(2)) - s3*s4*(qd(1) + qd(2))) - s4*(- qd(3)*s3*(qd(1) + qd(2)))) - c5*(- 295*c3^2*(qd(1) + qd(2))^2 + s2*( - 270*qd(1)^2) - 295*s3^2*(qd(1) + qd(2))^2) + 80*qd(5)*(-c5*(-qd(3) + qd(4)) - s5*(-c3*s4*(qd(1) + qd(2)) + c4*s3*(qd(1) + qd(2))))  - s5*(c4*(c3*(c2*( - 270*qd(1)^2) - (qd(1) + qd(2))*(90*qd(1) + 90*qd(2)))) - s4*( - s3*(c2*(- 270*qd(1)^2) - (qd(1) + qd(2))*(90*qd(1) + 90*qd(2))))) + (80*c5*(-qd(3) + qd(4)) + 80*s5*(-c3*s4*(qd(1) + qd(2)) + c4*s3*(qd(1) + qd(2))))*(-c3*c4*(qd(1) + qd(2)) + qd(5) - s3*s4*(qd(1) + qd(2)))) - (80*c6*(c5*(-c3*s4*(qd(1) + qd(2)) + c4*s3*(qd(1) + qd(2))) - s5*(-qd(3) + qd(4))) - 80*s6*(-c5*(-qd(3) + qd(4)) - s5*(-c3*s4*(qd(1) + qd(2)) + c4*s3*(qd(1) + qd(2)))))*(c3*c4*(qd(1) + qd(2)) - qd(5) + qd(6) + s3*s4*(qd(1) + qd(2))))  - 0.000409305*c5*(c4*(c3*qd(3)*(qd(1) + qd(2))) + qd(4)*(-c3*c4*(qd(1) + qd(2)) - s3*s4*(qd(1) + qd(2))) - s4*(- qd(3)*s3*(qd(1) + qd(2)))) - 295*m6*(c5*(c4*(c3*(c2*(- 270*qd(1)^2) - (qd(1) + qd(2))*(90*qd(1) + 90*qd(2)))) - s4*(- s3*(c2*(- 270*qd(1)^2) - (qd(1) + qd(2))*(90*qd(1) + 90*qd(2))))) - s5*( - 295*c3^2*(qd(1) + qd(2))^2 + s2*(- 270*qd(1)^2) - 295*s3^2*(qd(1) + qd(2))^2)) + 295*m7*s5*(80*c6*(c5*(c4*(c3*qd(3)*(qd(1) + qd(2))) + qd(4)*(-c3*c4*(qd(1) + qd(2)) - s3*s4*(qd(1) + qd(2))) - s4*( - qd(3)*s3*(qd(1) + qd(2)))) + qd(5)*(-c5*(-qd(3) + qd(4)) - s5*(-c3*s4*(qd(1) + qd(2)) + c4*s3*(qd(1) + qd(2))))) - c6*(80*c5*(c4*(c3*qd(3)*(qd(1) + qd(2))) + qd(4)*(-c3*c4*(qd(1) + qd(2)) - s3*s4*(qd(1) + qd(2))) - s4*(- qd(3)*s3*(qd(1) + qd(2)))) - c5*(- 295*c3^2*(qd(1) + qd(2))^2 + s2*(- 270*qd(1)^2) - 295*s3^2*(qd(1) + qd(2))^2) + 80*qd(5)*(-c5*(-qd(3) + qd(4)) - s5*(-c3*s4*(qd(1) + qd(2)) + c4*s3*(qd(1) + qd(2)))) - s5*(c4*( c3*(c2*(- 270*qd(1)^2) - (qd(1) + qd(2))*(90*qd(1) + 90*qd(2)))) - s4*(- s3*(c2*(- 270*qd(1)^2)  - (qd(1) + qd(2))*(90*qd(1) + 90*qd(2))))) + (80*c5*(-qd(3) + qd(4)) + 80*s5*(-c3*s4*(qd(1) + qd(2)) + c4*s3*(qd(1) + qd(2))))*(-c3*c4*(qd(1) + qd(2)) + qd(5) - s3*s4*(qd(1) + qd(2)))) + 80*qd(6)*(-c6*(-c5*(-qd(3) + qd(4)) - s5*(-c3*s4*(qd(1) + qd(2)) + c4*s3*(qd(1) + qd(2)))) - s6*(c5*(-c3*s4*(qd(1) + qd(2)) + c4*s3*(qd(1) + qd(2))) - s5*(-qd(3) + qd(4)))) - 80*s6*(- qd(5)*(c5*(-c3*s4*(qd(1) + qd(2)) + c4*s3*(qd(1) + qd(2))) - s5*(-qd(3) + qd(4))) - s5*(c4*(c3*qd(3)*(qd(1) + qd(2))) + qd(4)*(-c3*c4*(qd(1) + qd(2)) - s3*s4*(qd(1) + qd(2))) - s4*(- qd(3)*s3*(qd(1) + qd(2))))) - s6*( c5*(c4*( c3*(c2*(- 270*qd(1)^2) - (qd(1) + qd(2))*(90*qd(1) + 90*qd(2)))) - s4*(- s3*(c2*(- 270*qd(1)^2) - (qd(1) + qd(2))*(90*qd(1) + 90*qd(2))))) + 80*qd(5)*(c5*(-c3*s4*(qd(1) + qd(2)) + c4*s3*(qd(1) + qd(2))) - s5*(-qd(3) + qd(4))) + 80*s5*(c4*(c3*qd(3)*(qd(1) + qd(2))) + qd(4)*(-c3*c4*(qd(1) + qd(2)) - s3*s4*(qd(1) + qd(2))) - s4*(- qd(3)*s3*(qd(1) + qd(2)))) - s5*( - 295*c3^2*(qd(1) + qd(2))^2 + s2*(- 270*qd(1)^2) - 295*s3^2*(qd(1) + qd(2))^2) - (80*c5*(-c3*s4*(qd(1) + qd(2)) + c4*s3*(qd(1) + qd(2))) - 80*s5*(-qd(3) + qd(4)))*(-c3*c4*(qd(1) + qd(2)) + qd(5) - s3*s4*(qd(1) + qd(2)))) + (80*c6*(-c5*(-qd(3) + qd(4)) - s5*(-c3*s4*(qd(1) + qd(2)) + c4*s3*(qd(1) + qd(2)))) + 80*s6*(c5*(-c3*s4*(qd(1) + qd(2)) + c4*s3*(qd(1) + qd(2))) - s5*(-qd(3) + qd(4))))*(c3*c4*(qd(1) + qd(2)) - qd(5) + qd(6) + s3*s4*(qd(1) + qd(2)))) + 3.29301e-6*qd(4)*(-c3*s4*(qd(1) + qd(2)) + c4*s3*(qd(1) + qd(2))) - 0.000409305*qd(5)*(-c5*(-qd(3) + qd(4)) - s5*(-c3*s4*(qd(1) + qd(2)) + c4*s3*(qd(1) + qd(2)))) - 0.00355535*qd(5)*(c5*(-c3*s4*(qd(1) + qd(2)) + c4*s3*(qd(1) + qd(2))) - s5*(-qd(3) + qd(4))) + 3.29301e-6*s4*(c3*qd(3)*(qd(1) + qd(2))) - 0.00355535*s5*(c4*(c3*qd(3)*(qd(1) + qd(2))) + qd(4)*(-c3*c4*(qd(1) + qd(2)) - s3*s4*(qd(1) + qd(2))) - s4*(- qd(3)*s3*(qd(1) + qd(2)))) - (c5*(-c3*s4*(qd(1) + qd(2)) + c4*s3*(qd(1) + qd(2))) - s5*(-qd(3) + qd(4)))*(-0.00358942*c3*c4*(qd(1) + qd(2)) + 0.00358942*qd(5) - 0.00358942*s3*s4*(qd(1) + qd(2))) - (-c6*(-c5*(-qd(3) + qd(4)) - s5*(-c3*s4*(qd(1) + qd(2)) + c4*s3*(qd(1) + qd(2)))) - s6*(c5*(-c3*s4*(qd(1) + qd(2)) + c4*s3*(qd(1) + qd(2))) - s5*(-qd(3) + qd(4))))*(6.20477e-6*c6*(c5*(-c3*s4*(qd(1) + qd(2)) + c4*s3*(qd(1) + qd(2))) - s5*(-qd(3) + qd(4))) - 6.20477e-6*s6*(-c5*(-qd(3) + qd(4)) - s5*(-c3*s4*(qd(1) + qd(2)) + c4*s3*(qd(1) + qd(2))))) + (-3.01352e-6*c6*(-c5*(-qd(3) + qd(4)) - s5*(-c3*s4*(qd(1) + qd(2)) + c4*s3*(qd(1) + qd(2)))) - 3.01352e-6*s6*(c5*(-c3*s4*(qd(1) + qd(2)) + c4*s3*(qd(1) + qd(2))) - s5*(-qd(3) + qd(4))))*(c6*(c5*(-c3*s4*(qd(1) + qd(2)) + c4*s3*(qd(1) + qd(2))) - s5*(-qd(3) + qd(4))) - s6*(-c5*(-qd(3) + qd(4)) - s5*(-c3*s4*(qd(1) + qd(2)) + c4*s3*(qd(1) + qd(2))))) + (-c3*c4*(qd(1) + qd(2)) + qd(5) - s3*s4*(qd(1) + qd(2)))*(0.000409305*c5*(-qd(3) + qd(4)) + 0.00151607*c5*(-c3*s4*(qd(1) + qd(2)) + c4*s3*(qd(1) + qd(2))) - 0.00151607*s5*(-qd(3) + qd(4)) + 0.000409305*s5*(-c3*s4*(qd(1) + qd(2)) + c4*s3*(qd(1) + qd(2))))) - (-qd(3) + qd(4))*(-0.020170031*c3*c4*(qd(1) + qd(2)) + 0.00163355*c3*s4*(qd(1) + qd(2)) - 0.00163355*c4*s3*(qd(1) + qd(2)) + 2.69102e-6*qd(3) - 2.69102e-6*qd(4) - 0.020170031*s3*s4*(qd(1) + qd(2))) + (-c3*c4*(qd(1) + qd(2)) - s3*s4*(qd(1) + qd(2)))*(2.69102e-6*c3*c4*(qd(1) + qd(2)) + 8.41256e-6*c3*s4*(qd(1) + qd(2)) - 8.41256e-6*c4*s3*(qd(1) + qd(2)) - 0.024130024*qd(3) + 0.024130024*qd(4) + 2.69102e-6*s3*s4*(qd(1) + qd(2)));

